simulink model "KUKA_LBR_Simulink_model_flatness_based_control"  (R2017a)
(part 11 of 19)

dblCoriolisCentrifugalFullRow1Col6 = (q14*(KUKA_LBR_param_.dblLink7InertZZ*(cos(q6)*sin(q2)*sin(q3)*sin(q5) + cos(q2)*(cos(q5)*cos(q6)*sin(q4) - cos(q4)*sin(q6)) - cos(q3)*sin(q2)*(cos(q4)*cos(q5)*cos(q6) + sin(q4)*sin(q6))) - (-(cos(q5)*(cos(q3)*sin(q1) + cos(q1)*cos(q2)*sin(q3))) + (cos(q4)*sin(q1)*sin(q3) - cos(q1)*(cos(q2)*cos(q3)*cos(q4) + sin(q2)*sin(q4)))*sin(q5))*(KUKA_LBR_param_.dblLink7InertXX*(cos(q6)*(-(cos(q4)*sin(q1)*sin(q2)) + (cos(q2)*cos(q3)*sin(q1) + cos(q1)*sin(q3))*sin(q4)) - (cos(q5)*sin(q1)*sin(q2)*sin(q4) + cos(q1)*(cos(q4)*cos(q5)*sin(q3) + cos(q3)*sin(q5)) + cos(q2)*sin(q1)*(cos(q3)*cos(q4)*cos(q5) - sin(q3)*sin(q5)))*sin(q6)) + KUKA_LBR_param_.dblLink7InertXY*(cos(q6)*(sin(q1)*sin(q3)*sin(q4) + cos(q1)*(cos(q4)*sin(q2) - cos(q2)*cos(q3)*sin(q4))) + (-(sin(q1)*(cos(q4)*cos(q5)*sin(q3) + cos(q3)*sin(q5))) + cos(q1)*(cos(q5)*sin(q2)*sin(q4) + cos(q2)*(cos(q3)*cos(q4)*cos(q5) - sin(q3)*sin(q5))))*sin(q6))) - (cos(q1)*(cos(q3)*cos(q5) - cos(q4)*sin(q3)*sin(q5)) - sin(q1)*(sin(q2)*sin(q4)*sin(q5) + cos(q2)*(cos(q5)*sin(q3) + cos(q3)*cos(q4)*sin(q5))))*(KUKA_LBR_param_.dblLink7InertXY*(cos(q6)*(-(cos(q4)*sin(q1)*sin(q2)) + (cos(q2)*cos(q3)*sin(q1) + cos(q1)*sin(q3))*sin(q4)) - (cos(q5)*sin(q1)*sin(q2)*sin(q4) + cos(q1)*(cos(q4)*cos(q5)*sin(q3) + cos(q3)*sin(q5)) + cos(q2)*sin(q1)*(cos(q3)*cos(q4)*cos(q5) - sin(q3)*sin(q5)))*sin(q6)) + KUKA_LBR_param_.dblLink7InertYY*(cos(q6)*(sin(q1)*sin(q3)*sin(q4) + cos(q1)*(cos(q4)*sin(q2) - cos(q2)*cos(q3)*sin(q4))) + (-(sin(q1)*(cos(q4)*cos(q5)*sin(q3) + cos(q3)*sin(q5))) + cos(q1)*(cos(q5)*sin(q2)*sin(q4) + cos(q2)*(cos(q3)*cos(q4)*cos(q5) - sin(q3)*sin(q5))))*sin(q6))) - (cos(q5)*sin(q2)*sin(q3) + (cos(q3)*cos(q4)*sin(q2) - cos(q2)*sin(q4))*sin(q5))*(KUKA_LBR_param_.dblLink7InertXZ*(cos(q6)*(-(cos(q4)*sin(q1)*sin(q2)) + (cos(q2)*cos(q3)*sin(q1) + cos(q1)*sin(q3))*sin(q4)) - (cos(q5)*sin(q1)*sin(q2)*sin(q4) + cos(q1)*(cos(q4)*cos(q5)*sin(q3) + cos(q3)*sin(q5)) + cos(q2)*sin(q1)*(cos(q3)*cos(q4)*cos(q5) - sin(q3)*sin(q5)))*sin(q6)) + KUKA_LBR_param_.dblLink7InertYZ*(cos(q6)*(sin(q1)*sin(q3)*sin(q4) + cos(q1)*(cos(q4)*sin(q2) - cos(q2)*cos(q3)*sin(q4))) + (-(sin(q1)*(cos(q4)*cos(q5)*sin(q3) + cos(q3)*sin(q5))) + cos(q1)*(cos(q5)*sin(q2)*sin(q4) + cos(q2)*(cos(q3)*cos(q4)*cos(q5) - sin(q3)*sin(q5))))*sin(q6))) + KUKA_LBR_param_.dblLink7InertYZ*(sin(q1)*sin(q2)*(cos(q5)*cos(q6)*sin(q4) - cos(q4)*sin(q6)) + cos(q1)*(cos(q4)*cos(q5)*cos(q6)*sin(q3) + cos(q3)*cos(q6)*sin(q5) + sin(q3)*sin(q4)*sin(q6)) + cos(q2)*sin(q1)*(-(cos(q6)*sin(q3)*sin(q5)) + cos(q3)*(cos(q4)*cos(q5)*cos(q6) + sin(q4)*sin(q6)))) + KUKA_LBR_param_.dblLink7InertXZ*(-(sin(q1)*(cos(q4)*cos(q5)*cos(q6)*sin(q3) + cos(q3)*cos(q6)*sin(q5) + sin(q3)*sin(q4)*sin(q6))) + cos(q1)*(sin(q2)*(cos(q5)*cos(q6)*sin(q4) - cos(q4)*sin(q6)) + cos(q2)*(cos(q3)*cos(q4)*cos(q5)*cos(q6) - cos(q6)*sin(q3)*sin(q5) + cos(q3)*sin(q4)*sin(q6)))) - (cos(q1)*(-(cos(q3)*cos(q5)) + cos(q4)*sin(q3)*sin(q5)) + sin(q1)*(sin(q2)*sin(q4)*sin(q5) + cos(q2)*(cos(q5)*sin(q3) + cos(q3)*cos(q4)*sin(q5))))*(KUKA_LBR_param_.dblLink7InertXX*(cos(q6)*(sin(q1)*sin(q3)*sin(q4) + cos(q1)*(cos(q4)*sin(q2) - cos(q2)*cos(q3)*sin(q4))) - (cos(q5)*(cos(q4)*sin(q1)*sin(q3) - cos(q1)*(cos(q2)*cos(q3)*cos(q4) + sin(q2)*sin(q4))) + (cos(q3)*sin(q1) + cos(q1)*cos(q2)*sin(q3))*sin(q5))*sin(q6)) + KUKA_LBR_param_.dblLink7InertXY*(cos(q6)*(cos(q4)*sin(q1)*sin(q2) - (cos(q2)*cos(q3)*sin(q1) + cos(q1)*sin(q3))*sin(q4)) + (cos(q5)*sin(q1)*sin(q2)*sin(q4) + cos(q1)*(cos(q4)*cos(q5)*sin(q3) + cos(q3)*sin(q5)) + cos(q2)*sin(q1)*(cos(q3)*cos(q4)*cos(q5) - sin(q3)*sin(q5)))*sin(q6)) + KUKA_LBR_param_.dblLink7InertXZ*(cos(q2)*(cos(q4)*cos(q6) + cos(q5)*sin(q4)*sin(q6)) + sin(q2)*(sin(q3)*sin(q5)*sin(q6) + cos(q3)*(cos(q6)*sin(q4) - cos(q4)*cos(q5)*sin(q6))))) - (sin(q1)*(-(cos(q3)*cos(q5)) + cos(q4)*sin(q3)*sin(q5)) - cos(q1)*(sin(q2)*sin(q4)*sin(q5) + cos(q2)*(cos(q5)*sin(q3) + cos(q3)*cos(q4)*sin(q5))))*(KUKA_LBR_param_.dblLink7InertXY*(cos(q6)*(sin(q1)*sin(q3)*sin(q4) + cos(q1)*(cos(q4)*sin(q2) - cos(q2)*cos(q3)*sin(q4))) - (cos(q5)*(cos(q4)*sin(q1)*sin(q3) - cos(q1)*(cos(q2)*cos(q3)*cos(q4) + sin(q2)*sin(q4))) + (cos(q3)*sin(q1) + cos(q1)*cos(q2)*sin(q3))*sin(q5))*sin(q6)) + KUKA_LBR_param_.dblLink7InertYY*(cos(q6)*(cos(q4)*sin(q1)*sin(q2) - (cos(q2)*cos(q3)*sin(q1) + cos(q1)*sin(q3))*sin(q4)) + (cos(q5)*sin(q1)*sin(q2)*sin(q4) + cos(q1)*(cos(q4)*cos(q5)*sin(q3) + cos(q3)*sin(q5)) + cos(q2)*sin(q1)*(cos(q3)*cos(q4)*cos(q5) - sin(q3)*sin(q5)))*sin(q6)) + KUKA_LBR_param_.dblLink7InertYZ*(cos(q2)*(cos(q4)*cos(q6) + cos(q5)*sin(q4)*sin(q6)) + sin(q2)*(sin(q3)*sin(q5)*sin(q6) + cos(q3)*(cos(q6)*sin(q4) - cos(q4)*cos(q5)*sin(q6))))) - KUKA_LBR_param_.dblLink7Mass*(sin(q1)*(cos(q6)*(-(KUKA_LBR_param_.dblLink7CogX*cos(q7)*sin(q3)*sin(q4)) + KUKA_LBR_param_.dblLink7CogZ*cos(q3)*sin(q5) + KUKA_LBR_param_.dblLink7CogY*sin(q3)*sin(q4)*sin(q7)) + sin(q6)*(KUKA_LBR_param_.dblLink7CogZ*sin(q3)*sin(q4) + cos(q3)*sin(q5)*(KUKA_LBR_param_.dblLink7CogX*cos(q7) - KUKA_LBR_param_.dblLink7CogY*sin(q7))) + cos(q4)*cos(q5)*sin(q3)*(KUKA_LBR_param_.dblLink7CogZ*cos(q6) + sin(q6)*(KUKA_LBR_param_.dblLink7CogX*cos(q7) - KUKA_LBR_param_.dblLink7CogY*sin(q7)))) - cos(q1)*(sin(q2)*(cos(q4)*(KUKA_LBR_param_.dblLink7CogX*cos(q6)*cos(q7) - KUKA_LBR_param_.dblLink7CogZ*sin(q6) - KUKA_LBR_param_.dblLink7CogY*cos(q6)*sin(q7)) + cos(q5)*sin(q4)*(KUKA_LBR_param_.dblLink7CogZ*cos(q6) + KUKA_LBR_param_.dblLink7CogX*cos(q7)*sin(q6) - KUKA_LBR_param_.dblLink7CogY*sin(q6)*sin(q7))) + cos(q2)*(-(sin(q3)*sin(q5)*(KUKA_LBR_param_.dblLink7CogZ*cos(q6) + sin(q6)*(KUKA_LBR_param_.dblLink7CogX*cos(q7) - KUKA_LBR_param_.dblLink7CogY*sin(q7)))) + cos(q3)*(sin(q4)*(-(KUKA_LBR_param_.dblLink7CogX*cos(q6)*cos(q7)) + KUKA_LBR_param_.dblLink7CogZ*sin(q6) + KUKA_LBR_param_.dblLink7CogY*cos(q6)*sin(q7)) + cos(q4)*cos(q5)*(KUKA_LBR_param_.dblLink7CogZ*cos(q6) + KUKA_LBR_param_.dblLink7CogX*cos(q7)*sin(q6) - KUKA_LBR_param_.dblLink7CogY*sin(q6)*sin(q7))))))*(cos(q1)*(cos(q3)*(-(cos(q6)*sin(q5)*(KUKA_LBR_param_.dblLink7CogY*cos(q7) + KUKA_LBR_param_.dblLink7CogX*sin(q7))) + cos(q5)*(KUKA_LBR_param_.dblLink7CogX*cos(q7) - KUKA_LBR_param_.dblLink7CogY*sin(q7))) - sin(q3)*(sin(q4)*sin(q6)*(KUKA_LBR_param_.dblLink7CogY*cos(q7) + KUKA_LBR_param_.dblLink7CogX*sin(q7)) + cos(q4)*(cos(q5)*cos(q6)*(KUKA_LBR_param_.dblLink7CogY*cos(q7) + KUKA_LBR_param_.dblLink7CogX*sin(q7)) + sin(q5)*(KUKA_LBR_param_.dblLink7CogX*cos(q7) - KUKA_LBR_param_.dblLink7CogY*sin(q7))))) + sin(q1)*(-(sin(q2)*(KUKA_LBR_param_.dblLink7CogX*cos(q7)*sin(q4)*sin(q5) - KUKA_LBR_param_.dblLink7CogY*sin(q4)*sin(q5)*sin(q7) + cos(q5)*cos(q6)*sin(q4)*(KUKA_LBR_param_.dblLink7CogY*cos(q7) + KUKA_LBR_param_.dblLink7CogX*sin(q7)) - cos(q4)*sin(q6)*(KUKA_LBR_param_.dblLink7CogY*cos(q7) + KUKA_LBR_param_.dblLink7CogX*sin(q7)))) + cos(q2)*(sin(q3)*(cos(q6)*sin(q5)*(KUKA_LBR_param_.dblLink7CogY*cos(q7) + KUKA_LBR_param_.dblLink7CogX*sin(q7)) + cos(q5)*(-(KUKA_LBR_param_.dblLink7CogX*cos(q7)) + KUKA_LBR_param_.dblLink7CogY*sin(q7))) - cos(q3)*(sin(q4)*sin(q6)*(KUKA_LBR_param_.dblLink7CogY*cos(q7) + KUKA_LBR_param_.dblLink7CogX*sin(q7)) + cos(q4)*(cos(q5)*cos(q6)*(KUKA_LBR_param_.dblLink7CogY*cos(q7) + KUKA_LBR_param_.dblLink7CogX*sin(q7)) + sin(q5)*(KUKA_LBR_param_.dblLink7CogX*cos(q7) - KUKA_LBR_param_.dblLink7CogY*sin(q7))))))) - KUKA_LBR_param_.dblLink7Mass*(cos(q1)*(-(cos(q3)*sin(q5)*(KUKA_LBR_param_.dblLink7CogZ*cos(q6) + sin(q6)*(KUKA_LBR_param_.dblLink7CogX*cos(q7) - KUKA_LBR_param_.dblLink7CogY*sin(q7)))) + sin(q3)*(-(cos(q4)*cos(q5)*(KUKA_LBR_param_.dblLink7CogZ*cos(q6) + sin(q6)*(KUKA_LBR_param_.dblLink7CogX*cos(q7) - KUKA_LBR_param_.dblLink7CogY*sin(q7)))) - sin(q4)*(KUKA_LBR_param_.dblLink7CogZ*sin(q6) + cos(q6)*(-(KUKA_LBR_param_.dblLink7CogX*cos(q7)) + KUKA_LBR_param_.dblLink7CogY*sin(q7))))) + sin(q1)*(sin(q2)*(cos(q4)*(-(KUKA_LBR_param_.dblLink7CogX*cos(q6)*cos(q7)) + KUKA_LBR_param_.dblLink7CogZ*sin(q6) + KUKA_LBR_param_.dblLink7CogY*cos(q6)*sin(q7)) - cos(q5)*sin(q4)*(KUKA_LBR_param_.dblLink7CogZ*cos(q6) + KUKA_LBR_param_.dblLink7CogX*cos(q7)*sin(q6) - KUKA_LBR_param_.dblLink7CogY*sin(q6)*sin(q7))) - cos(q2)*(-(sin(q3)*sin(q5)*(KUKA_LBR_param_.dblLink7CogZ*cos(q6) + sin(q6)*(KUKA_LBR_param_.dblLink7CogX*cos(q7) - KUKA_LBR_param_.dblLink7CogY*sin(q7)))) + cos(q3)*(sin(q4)*(-(KUKA_LBR_param_.dblLink7CogX*cos(q6)*cos(q7)) + KUKA_LBR_param_.dblLink7CogZ*sin(q6) + KUKA_LBR_param_.dblLink7CogY*cos(q6)*sin(q7)) + cos(q4)*cos(q5)*(KUKA_LBR_param_.dblLink7CogZ*cos(q6) + KUKA_LBR_param_.dblLink7CogX*cos(q7)*sin(q6) - KUKA_LBR_param_.dblLink7CogY*sin(q6)*sin(q7))))))*(sin(q1)*(cos(q3)*(cos(q6)*sin(q5)*(KUKA_LBR_param_.dblLink7CogY*cos(q7) + KUKA_LBR_param_.dblLink7CogX*sin(q7)) + cos(q5)*(-(KUKA_LBR_param_.dblLink7CogX*cos(q7)) + KUKA_LBR_param_.dblLink7CogY*sin(q7))) + sin(q3)*(sin(q4)*sin(q6)*(KUKA_LBR_param_.dblLink7CogY*cos(q7) + KUKA_LBR_param_.dblLink7CogX*sin(q7)) + cos(q4)*(cos(q5)*cos(q6)*(KUKA_LBR_param_.dblLink7CogY*cos(q7) + KUKA_LBR_param_.dblLink7CogX*sin(q7)) + sin(q5)*(KUKA_LBR_param_.dblLink7CogX*cos(q7) - KUKA_LBR_param_.dblLink7CogY*sin(q7))))) - cos(q1)*(sin(q2)*(cos(q7)*(KUKA_LBR_param_.dblLink7CogX*sin(q4)*sin(q5) - KUKA_LBR_param_.dblLink7CogY*cos(q4)*sin(q6)) - (KUKA_LBR_param_.dblLink7CogY*sin(q4)*sin(q5) + KUKA_LBR_param_.dblLink7CogX*cos(q4)*sin(q6))*sin(q7) + cos(q5)*cos(q6)*sin(q4)*(KUKA_LBR_param_.dblLink7CogY*cos(q7) + KUKA_LBR_param_.dblLink7CogX*sin(q7))) + cos(q2)*(sin(q3)*(-(cos(q6)*sin(q5)*(KUKA_LBR_param_.dblLink7CogY*cos(q7) + KUKA_LBR_param_.dblLink7CogX*sin(q7))) + cos(q5)*(KUKA_LBR_param_.dblLink7CogX*cos(q7) - KUKA_LBR_param_.dblLink7CogY*sin(q7))) + cos(q3)*(sin(q4)*sin(q6)*(KUKA_LBR_param_.dblLink7CogY*cos(q7) + KUKA_LBR_param_.dblLink7CogX*sin(q7)) + cos(q4)*(cos(q5)*cos(q6)*(KUKA_LBR_param_.dblLink7CogY*cos(q7) + KUKA_LBR_param_.dblLink7CogX*sin(q7)) + sin(q5)*(KUKA_LBR_param_.dblLink7CogX*cos(q7) - KUKA_LBR_param_.dblLink7CogY*sin(q7))))))) - KUKA_LBR_param_.dblLink7Mass*(-(cos(q1)*(cos(q6)*(-(KUKA_LBR_param_.dblLink7CogX*cos(q7)*sin(q3)*sin(q4)) + KUKA_LBR_param_.dblLink7CogZ*cos(q3)*sin(q5) + KUKA_LBR_param_.dblLink7CogY*sin(q3)*sin(q4)*sin(q7)) + sin(q6)*(KUKA_LBR_param_.dblLink7CogZ*sin(q3)*sin(q4) + cos(q3)*sin(q5)*(KUKA_LBR_param_.dblLink7CogX*cos(q7) - KUKA_LBR_param_.dblLink7CogY*sin(q7))) + cos(q4)*cos(q5)*sin(q3)*(KUKA_LBR_param_.dblLink7CogZ*cos(q6) + sin(q6)*(KUKA_LBR_param_.dblLink7CogX*cos(q7) - KUKA_LBR_param_.dblLink7CogY*sin(q7))))) - sin(q1)*(sin(q2)*(cos(q4)*(KUKA_LBR_param_.dblLink7CogX*cos(q6)*cos(q7) - KUKA_LBR_param_.dblLink7CogZ*sin(q6) - KUKA_LBR_param_.dblLink7CogY*cos(q6)*sin(q7)) + cos(q5)*sin(q4)*(KUKA_LBR_param_.dblLink7CogZ*cos(q6) + KUKA_LBR_param_.dblLink7CogX*cos(q7)*sin(q6) - KUKA_LBR_param_.dblLink7CogY*sin(q6)*sin(q7))) + cos(q2)*(-(sin(q3)*sin(q5)*(KUKA_LBR_param_.dblLink7CogZ*cos(q6) + sin(q6)*(KUKA_LBR_param_.dblLink7CogX*cos(q7) - KUKA_LBR_param_.dblLink7CogY*sin(q7)))) + cos(q3)*(sin(q4)*(-(KUKA_LBR_param_.dblLink7CogX*cos(q6)*cos(q7)) + KUKA_LBR_param_.dblLink7CogZ*sin(q6) + KUKA_LBR_param_.dblLink7CogY*cos(q6)*sin(q7)) + cos(q4)*cos(q5)*(KUKA_LBR_param_.dblLink7CogZ*cos(q6) + KUKA_LBR_param_.dblLink7CogX*cos(q7)*sin(q6) - KUKA_LBR_param_.dblLink7CogY*sin(q6)*sin(q7))))))*(sin(q1)*(cos(q3)*(-(cos(q6)*sin(q5)*(KUKA_LBR_param_.dblLink7CogY*cos(q7) + KUKA_LBR_param_.dblLink7CogX*sin(q7))) + cos(q5)*(KUKA_LBR_param_.dblLink7CogX*cos(q7) - KUKA_LBR_param_.dblLink7CogY*sin(q7))) - sin(q3)*(sin(q4)*sin(q6)*(KUKA_LBR_param_.dblLink7CogY*cos(q7) + KUKA_LBR_param_.dblLink7CogX*sin(q7)) + cos(q4)*(cos(q5)*cos(q6)*(KUKA_LBR_param_.dblLink7CogY*cos(q7) + KUKA_LBR_param_.dblLink7CogX*sin(q7)) + sin(q5)*(KUKA_LBR_param_.dblLink7CogX*cos(q7) - KUKA_LBR_param_.dblLink7CogY*sin(q7))))) + cos(q1)*(sin(q2)*(cos(q7)*(KUKA_LBR_param_.dblLink7CogX*sin(q4)*sin(q5) - KUKA_LBR_param_.dblLink7CogY*cos(q4)*sin(q6)) - (KUKA_LBR_param_.dblLink7CogY*sin(q4)*sin(q5) + KUKA_LBR_param_.dblLink7CogX*cos(q4)*sin(q6))*sin(q7) + cos(q5)*cos(q6)*sin(q4)*(KUKA_LBR_param_.dblLink7CogY*cos(q7) + KUKA_LBR_param_.dblLink7CogX*sin(q7))) + cos(q2)*(sin(q3)*(-(cos(q6)*sin(q5)*(KUKA_LBR_param_.dblLink7CogY*cos(q7) + KUKA_LBR_param_.dblLink7CogX*sin(q7))) + cos(q5)*(KUKA_LBR_param_.dblLink7CogX*cos(q7) - KUKA_LBR_param_.dblLink7CogY*sin(q7))) + cos(q3)*(sin(q4)*sin(q6)*(KUKA_LBR_param_.dblLink7CogY*cos(q7) + KUKA_LBR_param_.dblLink7CogX*sin(q7)) + cos(q4)*(cos(q5)*cos(q6)*(KUKA_LBR_param_.dblLink7CogY*cos(q7) + KUKA_LBR_param_.dblLink7CogX*sin(q7)) + sin(q5)*(KUKA_LBR_param_.dblLink7CogX*cos(q7) - KUKA_LBR_param_.dblLink7CogY*sin(q7))))))) - KUKA_LBR_param_.dblLink7Mass*(KUKA_LBR_param_.dblLink7CogZ*cos(q5)*cos(q6)*sin(q1)*sin(q2)*sin(q4) - KUKA_LBR_param_.dblLink7CogX*cos(q1)*cos(q6)*cos(q7)*sin(q3)*sin(q4) + KUKA_LBR_param_.dblLink7CogZ*cos(q1)*cos(q3)*cos(q6)*sin(q5) + KUKA_LBR_param_.dblLink7CogX*cos(q5)*cos(q7)*sin(q1)*sin(q2)*sin(q4)*sin(q6) + KUKA_LBR_param_.dblLink7CogZ*cos(q1)*sin(q3)*sin(q4)*sin(q6) + KUKA_LBR_param_.dblLink7CogX*cos(q1)*cos(q3)*cos(q7)*sin(q5)*sin(q6) + KUKA_LBR_param_.dblLink7CogY*cos(q1)*cos(q6)*sin(q3)*sin(q4)*sin(q7) - KUKA_LBR_param_.dblLink7CogY*cos(q5)*sin(q1)*sin(q2)*sin(q4)*sin(q6)*sin(q7) - KUKA_LBR_param_.dblLink7CogY*cos(q1)*cos(q3)*sin(q5)*sin(q6)*sin(q7) + cos(q4)*(cos(q6)*(KUKA_LBR_param_.dblLink7CogX*cos(q7)*sin(q1)*sin(q2) + KUKA_LBR_param_.dblLink7CogZ*cos(q1)*cos(q5)*sin(q3) - KUKA_LBR_param_.dblLink7CogY*sin(q1)*sin(q2)*sin(q7)) - sin(q6)*(KUKA_LBR_param_.dblLink7CogZ*sin(q1)*sin(q2) + cos(q1)*cos(q5)*sin(q3)*(-(KUKA_LBR_param_.dblLink7CogX*cos(q7)) + KUKA_LBR_param_.dblLink7CogY*sin(q7)))) + cos(q2)*sin(q1)*(-(sin(q3)*sin(q5)*(KUKA_LBR_param_.dblLink7CogZ*cos(q6) + sin(q6)*(KUKA_LBR_param_.dblLink7CogX*cos(q7) - KUKA_LBR_param_.dblLink7CogY*sin(q7)))) + cos(q3)*(sin(q4)*(-(KUKA_LBR_param_.dblLink7CogX*cos(q6)*cos(q7)) + KUKA_LBR_param_.dblLink7CogZ*sin(q6) + KUKA_LBR_param_.dblLink7CogY*cos(q6)*sin(q7)) + cos(q4)*cos(q5)*(KUKA_LBR_param_.dblLink7CogZ*cos(q6) + KUKA_LBR_param_.dblLink7CogX*cos(q7)*sin(q6) - KUKA_LBR_param_.dblLink7CogY*sin(q6)*sin(q7)))))*(-(sin(q1)*(cos(q3)*(cos(q6)*sin(q5)*(KUKA_LBR_param_.dblLink7CogY*cos(q7) + KUKA_LBR_param_.dblLink7CogX*sin(q7)) + cos(q5)*(-(KUKA_LBR_param_.dblLink7CogX*cos(q7)) + KUKA_LBR_param_.dblLink7CogY*sin(q7))) + sin(q3)*(sin(q4)*sin(q6)*(KUKA_LBR_param_.dblLink7CogY*cos(q7) + KUKA_LBR_param_.dblLink7CogX*sin(q7)) + cos(q4)*(cos(q5)*cos(q6)*(KUKA_LBR_param_.dblLink7CogY*cos(q7) + KUKA_LBR_param_.dblLink7CogX*sin(q7)) + sin(q5)*(KUKA_LBR_param_.dblLink7CogX*cos(q7) - KUKA_LBR_param_.dblLink7CogY*sin(q7)))))) + cos(q1)*(sin(q2)*(cos(q7)*(KUKA_LBR_param_.dblLink7CogX*sin(q4)*sin(q5) - KUKA_LBR_param_.dblLink7CogY*cos(q4)*sin(q6)) - (KUKA_LBR_param_.dblLink7CogY*sin(q4)*sin(q5) + KUKA_LBR_param_.dblLink7CogX*cos(q4)*sin(q6))*sin(q7) + cos(q5)*cos(q6)*sin(q4)*(KUKA_LBR_param_.dblLink7CogY*cos(q7) + KUKA_LBR_param_.dblLink7CogX*sin(q7))) + cos(q2)*(sin(q3)*(-(cos(q6)*sin(q5)*(KUKA_LBR_param_.dblLink7CogY*cos(q7) + KUKA_LBR_param_.dblLink7CogX*sin(q7))) + cos(q5)*(KUKA_LBR_param_.dblLink7CogX*cos(q7) - KUKA_LBR_param_.dblLink7CogY*sin(q7))) + cos(q3)*(sin(q4)*sin(q6)*(KUKA_LBR_param_.dblLink7CogY*cos(q7) + KUKA_LBR_param_.dblLink7CogX*sin(q7)) + cos(q4)*(cos(q5)*cos(q6)*(KUKA_LBR_param_.dblLink7CogY*cos(q7) + KUKA_LBR_param_.dblLink7CogX*sin(q7)) + sin(q5)*(KUKA_LBR_param_.dblLink7CogX*cos(q7) - KUKA_LBR_param_.dblLink7CogY*sin(q7))))))) - KUKA_LBR_param_.dblLink7Mass*(-(sin(q1)*(cos(q6)*(-(KUKA_LBR_param_.dblLink7CogX*cos(q7)*sin(q3)*sin(q4)) + KUKA_LBR_param_.dblLink7CogZ*cos(q3)*sin(q5) + KUKA_LBR_param_.dblLink7CogY*sin(q3)*sin(q4)*sin(q7)) + sin(q6)*(KUKA_LBR_param_.dblLink7CogZ*sin(q3)*sin(q4) + cos(q3)*sin(q5)*(KUKA_LBR_param_.dblLink7CogX*cos(q7) - KUKA_LBR_param_.dblLink7CogY*sin(q7))) + cos(q4)*cos(q5)*sin(q3)*(KUKA_LBR_param_.dblLink7CogZ*cos(q6) + sin(q6)*(KUKA_LBR_param_.dblLink7CogX*cos(q7) - KUKA_LBR_param_.dblLink7CogY*sin(q7))))) + cos(q1)*(sin(q2)*(cos(q4)*(KUKA_LBR_param_.dblLink7CogX*cos(q6)*cos(q7) - KUKA_LBR_param_.dblLink7CogZ*sin(q6) - KUKA_LBR_param_.dblLink7CogY*cos(q6)*sin(q7)) + cos(q5)*sin(q4)*(KUKA_LBR_param_.dblLink7CogZ*cos(q6) + KUKA_LBR_param_.dblLink7CogX*cos(q7)*sin(q6) - KUKA_LBR_param_.dblLink7CogY*sin(q6)*sin(q7))) + cos(q2)*(-(sin(q3)*sin(q5)*(KUKA_LBR_param_.dblLink7CogZ*cos(q6) + sin(q6)*(KUKA_LBR_param_.dblLink7CogX*cos(q7) - KUKA_LBR_param_.dblLink7CogY*sin(q7)))) + cos(q3)*(sin(q4)*(-(KUKA_LBR_param_.dblLink7CogX*cos(q6)*cos(q7)) + KUKA_LBR_param_.dblLink7CogZ*sin(q6) + KUKA_LBR_param_.dblLink7CogY*cos(q6)*sin(q7)) + cos(q4)*cos(q5)*(KUKA_LBR_param_.dblLink7CogZ*cos(q6) + KUKA_LBR_param_.dblLink7CogX*cos(q7)*sin(q6) - KUKA_LBR_param_.dblLink7CogY*sin(q6)*sin(q7))))))*(cos(q1)*(cos(q3)*(-(cos(q6)*sin(q5)*(KUKA_LBR_param_.dblLink7CogY*cos(q7) + KUKA_LBR_param_.dblLink7CogX*sin(q7))) + cos(q5)*(KUKA_LBR_param_.dblLink7CogX*cos(q7) - KUKA_LBR_param_.dblLink7CogY*sin(q7))) - sin(q3)*(sin(q4)*sin(q6)*(KUKA_LBR_param_.dblLink7CogY*cos(q7) + KUKA_LBR_param_.dblLink7CogX*sin(q7)) + cos(q4)*(cos(q5)*cos(q6)*(KUKA_LBR_param_.dblLink7CogY*cos(q7) + KUKA_LBR_param_.dblLink7CogX*sin(q7)) + sin(q5)*(KUKA_LBR_param_.dblLink7CogX*cos(q7) - KUKA_LBR_param_.dblLink7CogY*sin(q7))))) - sin(q1)*(sin(q2)*(cos(q7)*(KUKA_LBR_param_.dblLink7CogX*sin(q4)*sin(q5) - KUKA_LBR_param_.dblLink7CogY*cos(q4)*sin(q6)) - (KUKA_LBR_param_.dblLink7CogY*sin(q4)*sin(q5) + KUKA_LBR_param_.dblLink7CogX*cos(q4)*sin(q6))*sin(q7) + cos(q5)*cos(q6)*sin(q4)*(KUKA_LBR_param_.dblLink7CogY*cos(q7) + KUKA_LBR_param_.dblLink7CogX*sin(q7))) + cos(q2)*(sin(q3)*(-(cos(q6)*sin(q5)*(KUKA_LBR_param_.dblLink7CogY*cos(q7) + KUKA_LBR_param_.dblLink7CogX*sin(q7))) + cos(q5)*(KUKA_LBR_param_.dblLink7CogX*cos(q7) - KUKA_LBR_param_.dblLink7CogY*sin(q7))) + cos(q3)*(sin(q4)*sin(q6)*(KUKA_LBR_param_.dblLink7CogY*cos(q7) + KUKA_LBR_param_.dblLink7CogX*sin(q7)) + cos(q4)*(cos(q5)*cos(q6)*(KUKA_LBR_param_.dblLink7CogY*cos(q7) + KUKA_LBR_param_.dblLink7CogX*sin(q7)) + sin(q5)*(KUKA_LBR_param_.dblLink7CogX*cos(q7) - KUKA_LBR_param_.dblLink7CogY*sin(q7))))))) - KUKA_LBR_param_.dblLink7Mass*(-(sin(q1)*(cos(q6)*(-(KUKA_LBR_param_.dblLink7CogX*cos(q7)*sin(q3)*sin(q4)) + KUKA_LBR_param_.dblLink7CogZ*cos(q3)*sin(q5) + KUKA_LBR_param_.dblLink7CogY*sin(q3)*sin(q4)*sin(q7)) + sin(q6)*(KUKA_LBR_param_.dblLink7CogZ*sin(q3)*sin(q4) + cos(q3)*sin(q5)*(KUKA_LBR_param_.dblLink7CogX*cos(q7) - KUKA_LBR_param_.dblLink7CogY*sin(q7))) + cos(q4)*cos(q5)*sin(q3)*(KUKA_LBR_param_.dblLink7CogZ*cos(q6) + sin(q6)*(KUKA_LBR_param_.dblLink7CogX*cos(q7) - KUKA_LBR_param_.dblLink7CogY*sin(q7))))) + cos(q1)*(sin(q2)*(cos(q4)*(KUKA_LBR_param_.dblLink7CogX*cos(q6)*cos(q7) - KUKA_LBR_param_.dblLink7CogZ*sin(q6) - KUKA_LBR_param_.dblLink7CogY*cos(q6)*sin(q7)) + cos(q5)*sin(q4)*(KUKA_LBR_param_.dblLink7CogZ*cos(q6) + KUKA_LBR_param_.dblLink7CogX*cos(q7)*sin(q6) - KUKA_LBR_param_.dblLink7CogY*sin(q6)*sin(q7))) + cos(q2)*(-(sin(q3)*sin(q5)*(KUKA_LBR_param_.dblLink7CogZ*cos(q6) + sin(q6)*(KUKA_LBR_param_.dblLink7CogX*cos(q7) - KUKA_LBR_param_.dblLink7CogY*sin(q7)))) + cos(q3)*(sin(q4)*(-(KUKA_LBR_param_.dblLink7CogX*cos(q6)*cos(q7)) + KUKA_LBR_param_.dblLink7CogZ*sin(q6) + KUKA_LBR_param_.dblLink7CogY*cos(q6)*sin(q7)) + cos(q4)*cos(q5)*(KUKA_LBR_param_.dblLink7CogZ*cos(q6) + KUKA_LBR_param_.dblLink7CogX*cos(q7)*sin(q6) - KUKA_LBR_param_.dblLink7CogY*sin(q6)*sin(q7))))))*(cos(q1)*(cos(q3)*(cos(q6)*sin(q5)*(KUKA_LBR_param_.dblLink7CogY*cos(q7) + KUKA_LBR_param_.dblLink7CogX*sin(q7)) + cos(q5)*(-(KUKA_LBR_param_.dblLink7CogX*cos(q7)) + KUKA_LBR_param_.dblLink7CogY*sin(q7))) + sin(q3)*(sin(q4)*sin(q6)*(KUKA_LBR_param_.dblLink7CogY*cos(q7) + KUKA_LBR_param_.dblLink7CogX*sin(q7)) + cos(q4)*(cos(q5)*cos(q6)*(KUKA_LBR_param_.dblLink7CogY*cos(q7) + KUKA_LBR_param_.dblLink7CogX*sin(q7)) + sin(q5)*(KUKA_LBR_param_.dblLink7CogX*cos(q7) - KUKA_LBR_param_.dblLink7CogY*sin(q7))))) + sin(q1)*(sin(q2)*(cos(q7)*(KUKA_LBR_param_.dblLink7CogX*sin(q4)*sin(q5) - KUKA_LBR_param_.dblLink7CogY*cos(q4)*sin(q6)) - (KUKA_LBR_param_.dblLink7CogY*sin(q4)*sin(q5) + KUKA_LBR_param_.dblLink7CogX*cos(q4)*sin(q6))*sin(q7) + cos(q5)*cos(q6)*sin(q4)*(KUKA_LBR_param_.dblLink7CogY*cos(q7) + KUKA_LBR_param_.dblLink7CogX*sin(q7))) + cos(q2)*(sin(q3)*(-(cos(q6)*sin(q5)*(KUKA_LBR_param_.dblLink7CogY*cos(q7) + KUKA_LBR_param_.dblLink7CogX*sin(q7))) + cos(q5)*(KUKA_LBR_param_.dblLink7CogX*cos(q7) - KUKA_LBR_param_.dblLink7CogY*sin(q7))) + cos(q3)*(sin(q4)*sin(q6)*(KUKA_LBR_param_.dblLink7CogY*cos(q7) + KUKA_LBR_param_.dblLink7CogX*sin(q7)) + cos(q4)*(cos(q5)*cos(q6)*(KUKA_LBR_param_.dblLink7CogY*cos(q7) + KUKA_LBR_param_.dblLink7CogX*sin(q7)) + sin(q5)*(KUKA_LBR_param_.dblLink7CogX*cos(q7) - KUKA_LBR_param_.dblLink7CogY*sin(q7))))))) + KUKA_LBR_param_.dblLink7Mass*(sin(q1)*(-(cos(q3)*sin(q5)*(KUKA_LBR_param_.dblLink7CogZ*cos(q6) + sin(q6)*(KUKA_LBR_param_.dblLink7CogX*cos(q7) - KUKA_LBR_param_.dblLink7CogY*sin(q7)))) + sin(q3)*(-(cos(q4)*cos(q5)*(KUKA_LBR_param_.dblLink7CogZ*cos(q6) + sin(q6)*(KUKA_LBR_param_.dblLink7CogX*cos(q7) - KUKA_LBR_param_.dblLink7CogY*sin(q7)))) - sin(q4)*(KUKA_LBR_param_.dblLink7CogZ*sin(q6) + cos(q6)*(-(KUKA_LBR_param_.dblLink7CogX*cos(q7)) + KUKA_LBR_param_.dblLink7CogY*sin(q7))))) + cos(q1)*(sin(q2)*(cos(q4)*(KUKA_LBR_param_.dblLink7CogX*cos(q6)*cos(q7) - KUKA_LBR_param_.dblLink7CogZ*sin(q6) - KUKA_LBR_param_.dblLink7CogY*cos(q6)*sin(q7)) + cos(q5)*sin(q4)*(KUKA_LBR_param_.dblLink7CogZ*cos(q6) + KUKA_LBR_param_.dblLink7CogX*cos(q7)*sin(q6) - KUKA_LBR_param_.dblLink7CogY*sin(q6)*sin(q7))) + cos(q2)*(-(sin(q3)*sin(q5)*(KUKA_LBR_param_.dblLink7CogZ*cos(q6) + sin(q6)*(KUKA_LBR_param_.dblLink7CogX*cos(q7) - KUKA_LBR_param_.dblLink7CogY*sin(q7)))) + cos(q3)*(sin(q4)*(-(KUKA_LBR_param_.dblLink7CogX*cos(q6)*cos(q7)) + KUKA_LBR_param_.dblLink7CogZ*sin(q6) + KUKA_LBR_param_.dblLink7CogY*cos(q6)*sin(q7)) + cos(q4)*cos(q5)*(KUKA_LBR_param_.dblLink7CogZ*cos(q6) + KUKA_LBR_param_.dblLink7CogX*cos(q7)*sin(q6) - KUKA_LBR_param_.dblLink7CogY*sin(q6)*sin(q7))))))*(cos(q1)*(cos(q3)*(cos(q6)*sin(q5)*(KUKA_LBR_param_.dblLink7CogY*cos(q7) + KUKA_LBR_param_.dblLink7CogX*sin(q7)) + cos(q5)*(-(KUKA_LBR_param_.dblLink7CogX*cos(q7)) + KUKA_LBR_param_.dblLink7CogY*sin(q7))) + sin(q3)*(sin(q4)*sin(q6)*(KUKA_LBR_param_.dblLink7CogY*cos(q7) + KUKA_LBR_param_.dblLink7CogX*sin(q7)) + cos(q4)*(cos(q5)*cos(q6)*(KUKA_LBR_param_.dblLink7CogY*cos(q7) + KUKA_LBR_param_.dblLink7CogX*sin(q7)) + sin(q5)*(KUKA_LBR_param_.dblLink7CogX*cos(q7) - KUKA_LBR_param_.dblLink7CogY*sin(q7))))) + sin(q1)*(sin(q2)*(cos(q7)*(KUKA_LBR_param_.dblLink7CogX*sin(q4)*sin(q5) - KUKA_LBR_param_.dblLink7CogY*cos(q4)*sin(q6)) - (KUKA_LBR_param_.dblLink7CogY*sin(q4)*sin(q5) + KUKA_LBR_param_.dblLink7CogX*cos(q4)*sin(q6))*sin(q7) + cos(q5)*cos(q6)*sin(q4)*(KUKA_LBR_param_.dblLink7CogY*cos(q7) + KUKA_LBR_param_.dblLink7CogX*sin(q7))) + cos(q2)*(sin(q3)*(-(cos(q6)*sin(q5)*(KUKA_LBR_param_.dblLink7CogY*cos(q7) + KUKA_LBR_param_.dblLink7CogX*sin(q7))) + cos(q5)*(KUKA_LBR_param_.dblLink7CogX*cos(q7) - KUKA_LBR_param_.dblLink7CogY*sin(q7))) + cos(q3)*(sin(q4)*sin(q6)*(KUKA_LBR_param_.dblLink7CogY*cos(q7) + KUKA_LBR_param_.dblLink7CogX*sin(q7)) + cos(q4)*(cos(q5)*cos(q6)*(KUKA_LBR_param_.dblLink7CogY*cos(q7) + KUKA_LBR_param_.dblLink7CogX*sin(q7)) + sin(q5)*(KUKA_LBR_param_.dblLink7CogX*cos(q7) - KUKA_LBR_param_.dblLink7CogY*sin(q7))))))) + KUKA_LBR_param_.dblLink7Mass*(KUKA_LBR_param_.dblLink7CogZ*cos(q5)*cos(q6)*sin(q1)*sin(q2)*sin(q4) - KUKA_LBR_param_.dblLink7CogX*cos(q1)*cos(q6)*cos(q7)*sin(q3)*sin(q4) + KUKA_LBR_param_.dblLink7CogZ*cos(q1)*cos(q3)*cos(q6)*sin(q5) + KUKA_LBR_param_.dblLink7CogX*cos(q5)*cos(q7)*sin(q1)*sin(q2)*sin(q4)*sin(q6) + KUKA_LBR_param_.dblLink7CogZ*cos(q1)*sin(q3)*sin(q4)*sin(q6) + KUKA_LBR_param_.dblLink7CogX*cos(q1)*cos(q3)*cos(q7)*sin(q5)*sin(q6) + KUKA_LBR_param_.dblLink7CogY*cos(q1)*cos(q6)*sin(q3)*sin(q4)*sin(q7) - KUKA_LBR_param_.dblLink7CogY*cos(q5)*sin(q1)*sin(q2)*sin(q4)*sin(q6)*sin(q7) - KUKA_LBR_param_.dblLink7CogY*cos(q1)*cos(q3)*sin(q5)*sin(q6)*sin(q7) + cos(q4)*(cos(q6)*(KUKA_LBR_param_.dblLink7CogX*cos(q7)*sin(q1)*sin(q2) + KUKA_LBR_param_.dblLink7CogZ*cos(q1)*cos(q5)*sin(q3) - KUKA_LBR_param_.dblLink7CogY*sin(q1)*sin(q2)*sin(q7)) - sin(q6)*(KUKA_LBR_param_.dblLink7CogZ*sin(q1)*sin(q2) + cos(q1)*cos(q5)*sin(q3)*(-(KUKA_LBR_param_.dblLink7CogX*cos(q7)) + KUKA_LBR_param_.dblLink7CogY*sin(q7)))) + cos(q2)*sin(q1)*(-(sin(q3)*sin(q5)*(KUKA_LBR_param_.dblLink7CogZ*cos(q6) + sin(q6)*(KUKA_LBR_param_.dblLink7CogX*cos(q7) - KUKA_LBR_param_.dblLink7CogY*sin(q7)))) + cos(q3)*(sin(q4)*(-(KUKA_LBR_param_.dblLink7CogX*cos(q6)*cos(q7)) + KUKA_LBR_param_.dblLink7CogZ*sin(q6) + KUKA_LBR_param_.dblLink7CogY*cos(q6)*sin(q7)) + cos(q4)*cos(q5)*(KUKA_LBR_param_.dblLink7CogZ*cos(q6) + KUKA_LBR_param_.dblLink7CogX*cos(q7)*sin(q6) - KUKA_LBR_param_.dblLink7CogY*sin(q6)*sin(q7)))))*(sin(q1)*(cos(q3)*(-(cos(q6)*sin(q5)*(KUKA_LBR_param_.dblLink7CogY*cos(q7) + KUKA_LBR_param_.dblLink7CogX*sin(q7))) + cos(q5)*(KUKA_LBR_param_.dblLink7CogX*cos(q7) - KUKA_LBR_param_.dblLink7CogY*sin(q7))) - sin(q3)*(sin(q4)*sin(q6)*(KUKA_LBR_param_.dblLink7CogY*cos(q7) + KUKA_LBR_param_.dblLink7CogX*sin(q7)) + cos(q4)*(cos(q5)*cos(q6)*(KUKA_LBR_param_.dblLink7CogY*cos(q7) + KUKA_LBR_param_.dblLink7CogX*sin(q7)) + sin(q5)*(KUKA_LBR_param_.dblLink7CogX*cos(q7) - KUKA_LBR_param_.dblLink7CogY*sin(q7))))) + cos(q1)*(sin(q2)*(KUKA_LBR_param_.dblLink7CogX*cos(q7)*sin(q4)*sin(q5) - KUKA_LBR_param_.dblLink7CogY*sin(q4)*sin(q5)*sin(q7) + cos(q5)*cos(q6)*sin(q4)*(KUKA_LBR_param_.dblLink7CogY*cos(q7) + KUKA_LBR_param_.dblLink7CogX*sin(q7)) - cos(q4)*sin(q6)*(KUKA_LBR_param_.dblLink7CogY*cos(q7) + KUKA_LBR_param_.dblLink7CogX*sin(q7))) + cos(q2)*(sin(q3)*(-(cos(q6)*sin(q5)*(KUKA_LBR_param_.dblLink7CogY*cos(q7) + KUKA_LBR_param_.dblLink7CogX*sin(q7))) + cos(q5)*(KUKA_LBR_param_.dblLink7CogX*cos(q7) - KUKA_LBR_param_.dblLink7CogY*sin(q7))) + cos(q3)*(sin(q4)*sin(q6)*(KUKA_LBR_param_.dblLink7CogY*cos(q7) + KUKA_LBR_param_.dblLink7CogX*sin(q7)) + cos(q4)*(cos(q5)*cos(q6)*(KUKA_LBR_param_.dblLink7CogY*cos(q7) + KUKA_LBR_param_.dblLink7CogX*sin(q7)) + sin(q5)*(KUKA_LBR_param_.dblLink7CogX*cos(q7) - KUKA_LBR_param_.dblLink7CogY*sin(q7))))))) - 2*KUKA_LBR_param_.dblLink7Mass*(sin(q1)*(cos(q6)*sin(q3)*sin(q4) - (cos(q4)*cos(q5)*sin(q3) + cos(q3)*sin(q5))*sin(q6)) + cos(q1)*(cos(q5)*sin(q2)*sin(q4)*sin(q6) + cos(q4)*(cos(q6)*sin(q2) + cos(q2)*cos(q3)*cos(q5)*sin(q6)) - cos(q2)*(cos(q3)*cos(q6)*sin(q4) + sin(q3)*sin(q5)*sin(q6))))*(KUKA_LBR_param_.dblLink7CogY*cos(q7) + KUKA_LBR_param_.dblLink7CogX*sin(q7))*(cos(q1)*(cos(q3)*(cos(q5)*(KUKA_LBR_param_.dblLink7CogY*cos(q7) + KUKA_LBR_param_.dblLink7CogX*sin(q7)) + sin(q5)*(KUKA_LBR_param_.dblLink7CogX*cos(q6)*cos(q7) - KUKA_LBR_param_.dblLink7CogZ*sin(q6) - KUKA_LBR_param_.dblLink7CogY*cos(q6)*sin(q7))) + sin(q3)*(sin(q4)*(KUKA_LBR_param_.dblLink45Len + KUKA_LBR_param_.dblLink7CogZ*cos(q6) + KUKA_LBR_param_.dblLink7CogX*cos(q7)*sin(q6) - KUKA_LBR_param_.dblLink7CogY*sin(q6)*sin(q7)) - cos(q4)*(sin(q5)*(KUKA_LBR_param_.dblLink7CogY*cos(q7) + KUKA_LBR_param_.dblLink7CogX*sin(q7)) + cos(q5)*(-(KUKA_LBR_param_.dblLink7CogX*cos(q6)*cos(q7)) + KUKA_LBR_param_.dblLink7CogZ*sin(q6) + KUKA_LBR_param_.dblLink7CogY*cos(q6)*sin(q7))))) + sin(q1)*(-(sin(q2)*(KUKA_LBR_param_.dblLink23Len + KUKA_LBR_param_.dblLink7CogY*cos(q7)*sin(q4)*sin(q5) + KUKA_LBR_param_.dblLink7CogX*sin(q4)*sin(q5)*sin(q7) + cos(q5)*sin(q4)*(-(KUKA_LBR_param_.dblLink7CogX*cos(q6)*cos(q7)) + KUKA_LBR_param_.dblLink7CogZ*sin(q6) + KUKA_LBR_param_.dblLink7CogY*cos(q6)*sin(q7)) + cos(q4)*(KUKA_LBR_param_.dblLink45Len + KUKA_LBR_param_.dblLink7CogZ*cos(q6) + KUKA_LBR_param_.dblLink7CogX*cos(q7)*sin(q6) - KUKA_LBR_param_.dblLink7CogY*sin(q6)*sin(q7)))) + cos(q2)*(-(sin(q3)*(cos(q5)*(KUKA_LBR_param_.dblLink7CogY*cos(q7) + KUKA_LBR_param_.dblLink7CogX*sin(q7)) + sin(q5)*(KUKA_LBR_param_.dblLink7CogX*cos(q6)*cos(q7) - KUKA_LBR_param_.dblLink7CogZ*sin(q6) - KUKA_LBR_param_.dblLink7CogY*cos(q6)*sin(q7)))) + cos(q3)*(sin(q4)*(KUKA_LBR_param_.dblLink45Len + KUKA_LBR_param_.dblLink7CogZ*cos(q6) + KUKA_LBR_param_.dblLink7CogX*cos(q7)*sin(q6) - KUKA_LBR_param_.dblLink7CogY*sin(q6)*sin(q7)) - cos(q4)*(sin(q5)*(KUKA_LBR_param_.dblLink7CogY*cos(q7) + KUKA_LBR_param_.dblLink7CogX*sin(q7)) + cos(q5)*(-(KUKA_LBR_param_.dblLink7CogX*cos(q6)*cos(q7)) + KUKA_LBR_param_.dblLink7CogZ*sin(q6) + KUKA_LBR_param_.dblLink7CogY*cos(q6)*sin(q7))))))) - 2*KUKA_LBR_param_.dblLink7Mass*(-(cos(q1)*cos(q6)*sin(q3)*sin(q4)) + cos(q5)*sin(q1)*sin(q2)*sin(q4)*sin(q6) + cos(q1)*cos(q3)*sin(q5)*sin(q6) + cos(q4)*(cos(q6)*sin(q1)*sin(q2) + cos(q5)*(cos(q2)*cos(q3)*sin(q1) + cos(q1)*sin(q3))*sin(q6)) - cos(q2)*sin(q1)*(cos(q3)*cos(q6)*sin(q4) + sin(q3)*sin(q5)*sin(q6)))*(KUKA_LBR_param_.dblLink7CogY*cos(q7) + KUKA_LBR_param_.dblLink7CogX*sin(q7))*(sin(q1)*(cos(q3)*(cos(q5)*(KUKA_LBR_param_.dblLink7CogY*cos(q7) + KUKA_LBR_param_.dblLink7CogX*sin(q7)) + sin(q5)*(KUKA_LBR_param_.dblLink7CogX*cos(q6)*cos(q7) - KUKA_LBR_param_.dblLink7CogZ*sin(q6) - KUKA_LBR_param_.dblLink7CogY*cos(q6)*sin(q7))) + sin(q3)*(sin(q4)*(KUKA_LBR_param_.dblLink45Len + KUKA_LBR_param_.dblLink7CogZ*cos(q6) + KUKA_LBR_param_.dblLink7CogX*cos(q7)*sin(q6) - KUKA_LBR_param_.dblLink7CogY*sin(q6)*sin(q7)) - cos(q4)*(sin(q5)*(KUKA_LBR_param_.dblLink7CogY*cos(q7) + KUKA_LBR_param_.dblLink7CogX*sin(q7)) + cos(q5)*(-(KUKA_LBR_param_.dblLink7CogX*cos(q6)*cos(q7)) + KUKA_LBR_param_.dblLink7CogZ*sin(q6) + KUKA_LBR_param_.dblLink7CogY*cos(q6)*sin(q7))))) + cos(q1)*(sin(q2)*(KUKA_LBR_param_.dblLink23Len + KUKA_LBR_param_.dblLink7CogY*cos(q7)*sin(q4)*sin(q5) + KUKA_LBR_param_.dblLink7CogX*sin(q4)*sin(q5)*sin(q7) + cos(q5)*sin(q4)*(-(KUKA_LBR_param_.dblLink7CogX*cos(q6)*cos(q7)) + KUKA_LBR_param_.dblLink7CogZ*sin(q6) + KUKA_LBR_param_.dblLink7CogY*cos(q6)*sin(q7)) + cos(q4)*(KUKA_LBR_param_.dblLink45Len + KUKA_LBR_param_.dblLink7CogZ*cos(q6) + KUKA_LBR_param_.dblLink7CogX*cos(q7)*sin(q6) - KUKA_LBR_param_.dblLink7CogY*sin(q6)*sin(q7))) + cos(q2)*(sin(q3)*(cos(q5)*(KUKA_LBR_param_.dblLink7CogY*cos(q7) + KUKA_LBR_param_.dblLink7CogX*sin(q7)) + sin(q5)*(KUKA_LBR_param_.dblLink7CogX*cos(q6)*cos(q7) - KUKA_LBR_param_.dblLink7CogZ*sin(q6) - KUKA_LBR_param_.dblLink7CogY*cos(q6)*sin(q7))) + cos(q3)*(-(sin(q4)*(KUKA_LBR_param_.dblLink45Len + KUKA_LBR_param_.dblLink7CogZ*cos(q6) + KUKA_LBR_param_.dblLink7CogX*cos(q7)*sin(q6) - KUKA_LBR_param_.dblLink7CogY*sin(q6)*sin(q7))) + cos(q4)*(sin(q5)*(KUKA_LBR_param_.dblLink7CogY*cos(q7) + KUKA_LBR_param_.dblLink7CogX*sin(q7)) + cos(q5)*(-(KUKA_LBR_param_.dblLink7CogX*cos(q6)*cos(q7)) + KUKA_LBR_param_.dblLink7CogZ*sin(q6) + KUKA_LBR_param_.dblLink7CogY*cos(q6)*sin(q7)))))))))/2.0;
dblCoriolisCentrifugalFullRow1Col7 = (q14*(-((cos(q6)*(sin(q1)*sin(q3)*sin(q4) + cos(q1)*(cos(q4)*sin(q2) - cos(q2)*cos(q3)*sin(q4))) - (cos(q5)*(cos(q4)*sin(q1)*sin(q3) - cos(q1)*(cos(q2)*cos(q3)*cos(q4) + sin(q2)*sin(q4))) + (cos(q3)*sin(q1) + cos(q1)*cos(q2)*sin(q3))*sin(q5))*sin(q6))*(KUKA_LBR_param_.dblLink7InertXX*(cos(q6)*(-(cos(q4)*sin(q1)*sin(q2)) + (cos(q2)*cos(q3)*sin(q1) + cos(q1)*sin(q3))*sin(q4)) - (cos(q5)*sin(q1)*sin(q2)*sin(q4) + cos(q1)*(cos(q4)*cos(q5)*sin(q3) + cos(q3)*sin(q5)) + cos(q2)*sin(q1)*(cos(q3)*cos(q4)*cos(q5) - sin(q3)*sin(q5)))*sin(q6)) + KUKA_LBR_param_.dblLink7InertXY*(cos(q6)*(sin(q1)*sin(q3)*sin(q4) + cos(q1)*(cos(q4)*sin(q2) - cos(q2)*cos(q3)*sin(q4))) + (-(sin(q1)*(cos(q4)*cos(q5)*sin(q3) + cos(q3)*sin(q5))) + cos(q1)*(cos(q5)*sin(q2)*sin(q4) + cos(q2)*(cos(q3)*cos(q4)*cos(q5) - sin(q3)*sin(q5))))*sin(q6)))) - (cos(q6)*(cos(q4)*sin(q1)*sin(q2) - (cos(q2)*cos(q3)*sin(q1) + cos(q1)*sin(q3))*sin(q4)) + (cos(q5)*sin(q1)*sin(q2)*sin(q4) + cos(q1)*(cos(q4)*cos(q5)*sin(q3) + cos(q3)*sin(q5)) + cos(q2)*sin(q1)*(cos(q3)*cos(q4)*cos(q5) - sin(q3)*sin(q5)))*sin(q6))*(KUKA_LBR_param_.dblLink7InertXY*(cos(q6)*(-(cos(q4)*sin(q1)*sin(q2)) + (cos(q2)*cos(q3)*sin(q1) + cos(q1)*sin(q3))*sin(q4)) - (cos(q5)*sin(q1)*sin(q2)*sin(q4) + cos(q1)*(cos(q4)*cos(q5)*sin(q3) + cos(q3)*sin(q5)) + cos(q2)*sin(q1)*(cos(q3)*cos(q4)*cos(q5) - sin(q3)*sin(q5)))*sin(q6)) + KUKA_LBR_param_.dblLink7InertYY*(cos(q6)*(sin(q1)*sin(q3)*sin(q4) + cos(q1)*(cos(q4)*sin(q2) - cos(q2)*cos(q3)*sin(q4))) + (-(sin(q1)*(cos(q4)*cos(q5)*sin(q3) + cos(q3)*sin(q5))) + cos(q1)*(cos(q5)*sin(q2)*sin(q4) + cos(q2)*(cos(q3)*cos(q4)*cos(q5) - sin(q3)*sin(q5))))*sin(q6))) - (KUKA_LBR_param_.dblLink7InertXZ*(cos(q6)*(-(cos(q4)*sin(q1)*sin(q2)) + (cos(q2)*cos(q3)*sin(q1) + cos(q1)*sin(q3))*sin(q4)) - (cos(q5)*sin(q1)*sin(q2)*sin(q4) + cos(q1)*(cos(q4)*cos(q5)*sin(q3) + cos(q3)*sin(q5)) + cos(q2)*sin(q1)*(cos(q3)*cos(q4)*cos(q5) - sin(q3)*sin(q5)))*sin(q6)) + KUKA_LBR_param_.dblLink7InertYZ*(cos(q6)*(sin(q1)*sin(q3)*sin(q4) + cos(q1)*(cos(q4)*sin(q2) - cos(q2)*cos(q3)*sin(q4))) + (-(sin(q1)*(cos(q4)*cos(q5)*sin(q3) + cos(q3)*sin(q5))) + cos(q1)*(cos(q5)*sin(q2)*sin(q4) + cos(q2)*(cos(q3)*cos(q4)*cos(q5) - sin(q3)*sin(q5))))*sin(q6)))*(cos(q2)*(cos(q4)*cos(q6) + cos(q5)*sin(q4)*sin(q6)) + sin(q2)*(sin(q3)*sin(q5)*sin(q6) + cos(q3)*(cos(q6)*sin(q4) - cos(q4)*cos(q5)*sin(q6)))) - (cos(q6)*(-(cos(q4)*sin(q1)*sin(q2)) + (cos(q2)*cos(q3)*sin(q1) + cos(q1)*sin(q3))*sin(q4)) - (cos(q5)*sin(q1)*sin(q2)*sin(q4) + cos(q1)*(cos(q4)*cos(q5)*sin(q3) + cos(q3)*sin(q5)) + cos(q2)*sin(q1)*(cos(q3)*cos(q4)*cos(q5) - sin(q3)*sin(q5)))*sin(q6))*(KUKA_LBR_param_.dblLink7InertXX*(cos(q6)*(sin(q1)*sin(q3)*sin(q4) + cos(q1)*(cos(q4)*sin(q2) - cos(q2)*cos(q3)*sin(q4))) - (cos(q5)*(cos(q4)*sin(q1)*sin(q3) - cos(q1)*(cos(q2)*cos(q3)*cos(q4) + sin(q2)*sin(q4))) + (cos(q3)*sin(q1) + cos(q1)*cos(q2)*sin(q3))*sin(q5))*sin(q6)) + KUKA_LBR_param_.dblLink7InertXY*(cos(q6)*(cos(q4)*sin(q1)*sin(q2) - (cos(q2)*cos(q3)*sin(q1) + cos(q1)*sin(q3))*sin(q4)) + (cos(q5)*sin(q1)*sin(q2)*sin(q4) + cos(q1)*(cos(q4)*cos(q5)*sin(q3) + cos(q3)*sin(q5)) + cos(q2)*sin(q1)*(cos(q3)*cos(q4)*cos(q5) - sin(q3)*sin(q5)))*sin(q6)) + KUKA_LBR_param_.dblLink7InertXZ*(cos(q2)*(cos(q4)*cos(q6) + cos(q5)*sin(q4)*sin(q6)) + sin(q2)*(sin(q3)*sin(q5)*sin(q6) + cos(q3)*(cos(q6)*sin(q4) - cos(q4)*cos(q5)*sin(q6))))) - (cos(q6)*(sin(q1)*sin(q3)*sin(q4) + cos(q1)*(cos(q4)*sin(q2) - cos(q2)*cos(q3)*sin(q4))) + (-(sin(q1)*(cos(q4)*cos(q5)*sin(q3) + cos(q3)*sin(q5))) + cos(q1)*(cos(q5)*sin(q2)*sin(q4) + cos(q2)*(cos(q3)*cos(q4)*cos(q5) - sin(q3)*sin(q5))))*sin(q6))*(KUKA_LBR_param_.dblLink7InertXY*(cos(q6)*(sin(q1)*sin(q3)*sin(q4) + cos(q1)*(cos(q4)*sin(q2) - cos(q2)*cos(q3)*sin(q4))) - (cos(q5)*(cos(q4)*sin(q1)*sin(q3) - cos(q1)*(cos(q2)*cos(q3)*cos(q4) + sin(q2)*sin(q4))) + (cos(q3)*sin(q1) + cos(q1)*cos(q2)*sin(q3))*sin(q5))*sin(q6)) + KUKA_LBR_param_.dblLink7InertYY*(cos(q6)*(cos(q4)*sin(q1)*sin(q2) - (cos(q2)*cos(q3)*sin(q1) + cos(q1)*sin(q3))*sin(q4)) + (cos(q5)*sin(q1)*sin(q2)*sin(q4) + cos(q1)*(cos(q4)*cos(q5)*sin(q3) + cos(q3)*sin(q5)) + cos(q2)*sin(q1)*(cos(q3)*cos(q4)*cos(q5) - sin(q3)*sin(q5)))*sin(q6)) + KUKA_LBR_param_.dblLink7InertYZ*(cos(q2)*(cos(q4)*cos(q6) + cos(q5)*sin(q4)*sin(q6)) + sin(q2)*(sin(q3)*sin(q5)*sin(q6) + cos(q3)*(cos(q6)*sin(q4) - cos(q4)*cos(q5)*sin(q6))))) - 2*KUKA_LBR_param_.dblLink7Mass*(cos(q1)*(cos(q3)*(-(cos(q6)*sin(q5)*(KUKA_LBR_param_.dblLink7CogY*cos(q7) + KUKA_LBR_param_.dblLink7CogX*sin(q7))) + cos(q5)*(KUKA_LBR_param_.dblLink7CogX*cos(q7) - KUKA_LBR_param_.dblLink7CogY*sin(q7))) - sin(q3)*(sin(q4)*sin(q6)*(KUKA_LBR_param_.dblLink7CogY*cos(q7) + KUKA_LBR_param_.dblLink7CogX*sin(q7)) + cos(q4)*(cos(q5)*cos(q6)*(KUKA_LBR_param_.dblLink7CogY*cos(q7) + KUKA_LBR_param_.dblLink7CogX*sin(q7)) + sin(q5)*(KUKA_LBR_param_.dblLink7CogX*cos(q7) - KUKA_LBR_param_.dblLink7CogY*sin(q7))))) + sin(q1)*(-(sin(q2)*(KUKA_LBR_param_.dblLink7CogX*cos(q7)*sin(q4)*sin(q5) - KUKA_LBR_param_.dblLink7CogY*sin(q4)*sin(q5)*sin(q7) + cos(q5)*cos(q6)*sin(q4)*(KUKA_LBR_param_.dblLink7CogY*cos(q7) + KUKA_LBR_param_.dblLink7CogX*sin(q7)) - cos(q4)*sin(q6)*(KUKA_LBR_param_.dblLink7CogY*cos(q7) + KUKA_LBR_param_.dblLink7CogX*sin(q7)))) + cos(q2)*(sin(q3)*(cos(q6)*sin(q5)*(KUKA_LBR_param_.dblLink7CogY*cos(q7) + KUKA_LBR_param_.dblLink7CogX*sin(q7)) + cos(q5)*(-(KUKA_LBR_param_.dblLink7CogX*cos(q7)) + KUKA_LBR_param_.dblLink7CogY*sin(q7))) - cos(q3)*(sin(q4)*sin(q6)*(KUKA_LBR_param_.dblLink7CogY*cos(q7) + KUKA_LBR_param_.dblLink7CogX*sin(q7)) + cos(q4)*(cos(q5)*cos(q6)*(KUKA_LBR_param_.dblLink7CogY*cos(q7) + KUKA_LBR_param_.dblLink7CogX*sin(q7)) + sin(q5)*(KUKA_LBR_param_.dblLink7CogX*cos(q7) - KUKA_LBR_param_.dblLink7CogY*sin(q7)))))))*(sin(q1)*(cos(q3)*(cos(q6)*sin(q5)*(KUKA_LBR_param_.dblLink7CogY*cos(q7) + KUKA_LBR_param_.dblLink7CogX*sin(q7)) + cos(q5)*(-(KUKA_LBR_param_.dblLink7CogX*cos(q7)) + KUKA_LBR_param_.dblLink7CogY*sin(q7))) + sin(q3)*(sin(q4)*sin(q6)*(KUKA_LBR_param_.dblLink7CogY*cos(q7) + KUKA_LBR_param_.dblLink7CogX*sin(q7)) + cos(q4)*(cos(q5)*cos(q6)*(KUKA_LBR_param_.dblLink7CogY*cos(q7) + KUKA_LBR_param_.dblLink7CogX*sin(q7)) + sin(q5)*(KUKA_LBR_param_.dblLink7CogX*cos(q7) - KUKA_LBR_param_.dblLink7CogY*sin(q7))))) - cos(q1)*(sin(q2)*(cos(q7)*(KUKA_LBR_param_.dblLink7CogX*sin(q4)*sin(q5) - KUKA_LBR_param_.dblLink7CogY*cos(q4)*sin(q6)) - (KUKA_LBR_param_.dblLink7CogY*sin(q4)*sin(q5) + KUKA_LBR_param_.dblLink7CogX*cos(q4)*sin(q6))*sin(q7) + cos(q5)*cos(q6)*sin(q4)*(KUKA_LBR_param_.dblLink7CogY*cos(q7) + KUKA_LBR_param_.dblLink7CogX*sin(q7))) + cos(q2)*(sin(q3)*(-(cos(q6)*sin(q5)*(KUKA_LBR_param_.dblLink7CogY*cos(q7) + KUKA_LBR_param_.dblLink7CogX*sin(q7))) + cos(q5)*(KUKA_LBR_param_.dblLink7CogX*cos(q7) - KUKA_LBR_param_.dblLink7CogY*sin(q7))) + cos(q3)*(sin(q4)*sin(q6)*(KUKA_LBR_param_.dblLink7CogY*cos(q7) + KUKA_LBR_param_.dblLink7CogX*sin(q7)) + cos(q4)*(cos(q5)*cos(q6)*(KUKA_LBR_param_.dblLink7CogY*cos(q7) + KUKA_LBR_param_.dblLink7CogX*sin(q7)) + sin(q5)*(KUKA_LBR_param_.dblLink7CogX*cos(q7) - KUKA_LBR_param_.dblLink7CogY*sin(q7))))))) - 2*KUKA_LBR_param_.dblLink7Mass*(sin(q1)*(cos(q3)*(-(cos(q6)*sin(q5)*(KUKA_LBR_param_.dblLink7CogY*cos(q7) + KUKA_LBR_param_.dblLink7CogX*sin(q7))) + cos(q5)*(KUKA_LBR_param_.dblLink7CogX*cos(q7) - KUKA_LBR_param_.dblLink7CogY*sin(q7))) - sin(q3)*(sin(q4)*sin(q6)*(KUKA_LBR_param_.dblLink7CogY*cos(q7) + KUKA_LBR_param_.dblLink7CogX*sin(q7)) + cos(q4)*(cos(q5)*cos(q6)*(KUKA_LBR_param_.dblLink7CogY*cos(q7) + KUKA_LBR_param_.dblLink7CogX*sin(q7)) + sin(q5)*(KUKA_LBR_param_.dblLink7CogX*cos(q7) - KUKA_LBR_param_.dblLink7CogY*sin(q7))))) + cos(q1)*(sin(q2)*(cos(q7)*(KUKA_LBR_param_.dblLink7CogX*sin(q4)*sin(q5) - KUKA_LBR_param_.dblLink7CogY*cos(q4)*sin(q6)) - (KUKA_LBR_param_.dblLink7CogY*sin(q4)*sin(q5) + KUKA_LBR_param_.dblLink7CogX*cos(q4)*sin(q6))*sin(q7) + cos(q5)*cos(q6)*sin(q4)*(KUKA_LBR_param_.dblLink7CogY*cos(q7) + KUKA_LBR_param_.dblLink7CogX*sin(q7))) + cos(q2)*(sin(q3)*(-(cos(q6)*sin(q5)*(KUKA_LBR_param_.dblLink7CogY*cos(q7) + KUKA_LBR_param_.dblLink7CogX*sin(q7))) + cos(q5)*(KUKA_LBR_param_.dblLink7CogX*cos(q7) - KUKA_LBR_param_.dblLink7CogY*sin(q7))) + cos(q3)*(sin(q4)*sin(q6)*(KUKA_LBR_param_.dblLink7CogY*cos(q7) + KUKA_LBR_param_.dblLink7CogX*sin(q7)) + cos(q4)*(cos(q5)*cos(q6)*(KUKA_LBR_param_.dblLink7CogY*cos(q7) + KUKA_LBR_param_.dblLink7CogX*sin(q7)) + sin(q5)*(KUKA_LBR_param_.dblLink7CogX*cos(q7) - KUKA_LBR_param_.dblLink7CogY*sin(q7)))))))*(cos(q1)*(cos(q3)*(-(cos(q6)*sin(q5)*(KUKA_LBR_param_.dblLink7CogY*cos(q7) + KUKA_LBR_param_.dblLink7CogX*sin(q7))) + cos(q5)*(KUKA_LBR_param_.dblLink7CogX*cos(q7) - KUKA_LBR_param_.dblLink7CogY*sin(q7))) - sin(q3)*(sin(q4)*sin(q6)*(KUKA_LBR_param_.dblLink7CogY*cos(q7) + KUKA_LBR_param_.dblLink7CogX*sin(q7)) + cos(q4)*(cos(q5)*cos(q6)*(KUKA_LBR_param_.dblLink7CogY*cos(q7) + KUKA_LBR_param_.dblLink7CogX*sin(q7)) + sin(q5)*(KUKA_LBR_param_.dblLink7CogX*cos(q7) - KUKA_LBR_param_.dblLink7CogY*sin(q7))))) - sin(q1)*(sin(q2)*(cos(q7)*(KUKA_LBR_param_.dblLink7CogX*sin(q4)*sin(q5) - KUKA_LBR_param_.dblLink7CogY*cos(q4)*sin(q6)) - (KUKA_LBR_param_.dblLink7CogY*sin(q4)*sin(q5) + KUKA_LBR_param_.dblLink7CogX*cos(q4)*sin(q6))*sin(q7) + cos(q5)*cos(q6)*sin(q4)*(KUKA_LBR_param_.dblLink7CogY*cos(q7) + KUKA_LBR_param_.dblLink7CogX*sin(q7))) + cos(q2)*(sin(q3)*(-(cos(q6)*sin(q5)*(KUKA_LBR_param_.dblLink7CogY*cos(q7) + KUKA_LBR_param_.dblLink7CogX*sin(q7))) + cos(q5)*(KUKA_LBR_param_.dblLink7CogX*cos(q7) - KUKA_LBR_param_.dblLink7CogY*sin(q7))) + cos(q3)*(sin(q4)*sin(q6)*(KUKA_LBR_param_.dblLink7CogY*cos(q7) + KUKA_LBR_param_.dblLink7CogX*sin(q7)) + cos(q4)*(cos(q5)*cos(q6)*(KUKA_LBR_param_.dblLink7CogY*cos(q7) + KUKA_LBR_param_.dblLink7CogX*sin(q7)) + sin(q5)*(KUKA_LBR_param_.dblLink7CogX*cos(q7) - KUKA_LBR_param_.dblLink7CogY*sin(q7))))))) - 2*KUKA_LBR_param_.dblLink7Mass*(-(sin(q1)*(cos(q3)*(cos(q6)*sin(q5)*(KUKA_LBR_param_.dblLink7CogY*cos(q7) + KUKA_LBR_param_.dblLink7CogX*sin(q7)) + cos(q5)*(-(KUKA_LBR_param_.dblLink7CogX*cos(q7)) + KUKA_LBR_param_.dblLink7CogY*sin(q7))) + sin(q3)*(sin(q4)*sin(q6)*(KUKA_LBR_param_.dblLink7CogY*cos(q7) + KUKA_LBR_param_.dblLink7CogX*sin(q7)) + cos(q4)*(cos(q5)*cos(q6)*(KUKA_LBR_param_.dblLink7CogY*cos(q7) + KUKA_LBR_param_.dblLink7CogX*sin(q7)) + sin(q5)*(KUKA_LBR_param_.dblLink7CogX*cos(q7) - KUKA_LBR_param_.dblLink7CogY*sin(q7)))))) + cos(q1)*(sin(q2)*(cos(q7)*(KUKA_LBR_param_.dblLink7CogX*sin(q4)*sin(q5) - KUKA_LBR_param_.dblLink7CogY*cos(q4)*sin(q6)) - (KUKA_LBR_param_.dblLink7CogY*sin(q4)*sin(q5) + KUKA_LBR_param_.dblLink7CogX*cos(q4)*sin(q6))*sin(q7) + cos(q5)*cos(q6)*sin(q4)*(KUKA_LBR_param_.dblLink7CogY*cos(q7) + KUKA_LBR_param_.dblLink7CogX*sin(q7))) + cos(q2)*(sin(q3)*(-(cos(q6)*sin(q5)*(KUKA_LBR_param_.dblLink7CogY*cos(q7) + KUKA_LBR_param_.dblLink7CogX*sin(q7))) + cos(q5)*(KUKA_LBR_param_.dblLink7CogX*cos(q7) - KUKA_LBR_param_.dblLink7CogY*sin(q7))) + cos(q3)*(sin(q4)*sin(q6)*(KUKA_LBR_param_.dblLink7CogY*cos(q7) + KUKA_LBR_param_.dblLink7CogX*sin(q7)) + cos(q4)*(cos(q5)*cos(q6)*(KUKA_LBR_param_.dblLink7CogY*cos(q7) + KUKA_LBR_param_.dblLink7CogX*sin(q7)) + sin(q5)*(KUKA_LBR_param_.dblLink7CogX*cos(q7) - KUKA_LBR_param_.dblLink7CogY*sin(q7)))))))*(cos(q1)*(cos(q3)*(cos(q6)*sin(q5)*(KUKA_LBR_param_.dblLink7CogY*cos(q7) + KUKA_LBR_param_.dblLink7CogX*sin(q7)) + cos(q5)*(-(KUKA_LBR_param_.dblLink7CogX*cos(q7)) + KUKA_LBR_param_.dblLink7CogY*sin(q7))) + sin(q3)*(sin(q4)*sin(q6)*(KUKA_LBR_param_.dblLink7CogY*cos(q7) + KUKA_LBR_param_.dblLink7CogX*sin(q7)) + cos(q4)*(cos(q5)*cos(q6)*(KUKA_LBR_param_.dblLink7CogY*cos(q7) + KUKA_LBR_param_.dblLink7CogX*sin(q7)) + sin(q5)*(KUKA_LBR_param_.dblLink7CogX*cos(q7) - KUKA_LBR_param_.dblLink7CogY*sin(q7))))) + sin(q1)*(sin(q2)*(cos(q7)*(KUKA_LBR_param_.dblLink7CogX*sin(q4)*sin(q5) - KUKA_LBR_param_.dblLink7CogY*cos(q4)*sin(q6)) - (KUKA_LBR_param_.dblLink7CogY*sin(q4)*sin(q5) + KUKA_LBR_param_.dblLink7CogX*cos(q4)*sin(q6))*sin(q7) + cos(q5)*cos(q6)*sin(q4)*(KUKA_LBR_param_.dblLink7CogY*cos(q7) + KUKA_LBR_param_.dblLink7CogX*sin(q7))) + cos(q2)*(sin(q3)*(-(cos(q6)*sin(q5)*(KUKA_LBR_param_.dblLink7CogY*cos(q7) + KUKA_LBR_param_.dblLink7CogX*sin(q7))) + cos(q5)*(KUKA_LBR_param_.dblLink7CogX*cos(q7) - KUKA_LBR_param_.dblLink7CogY*sin(q7))) + cos(q3)*(sin(q4)*sin(q6)*(KUKA_LBR_param_.dblLink7CogY*cos(q7) + KUKA_LBR_param_.dblLink7CogX*sin(q7)) + cos(q4)*(cos(q5)*cos(q6)*(KUKA_LBR_param_.dblLink7CogY*cos(q7) + KUKA_LBR_param_.dblLink7CogX*sin(q7)) + sin(q5)*(KUKA_LBR_param_.dblLink7CogX*cos(q7) - KUKA_LBR_param_.dblLink7CogY*sin(q7))))))) + 2*KUKA_LBR_param_.dblLink7Mass*(cos(q1)*(cos(q3)*(cos(q6)*sin(q5)*(KUKA_LBR_param_.dblLink7CogY*cos(q7) + KUKA_LBR_param_.dblLink7CogX*sin(q7)) + cos(q5)*(-(KUKA_LBR_param_.dblLink7CogX*cos(q7)) + KUKA_LBR_param_.dblLink7CogY*sin(q7))) + sin(q3)*(sin(q4)*sin(q6)*(KUKA_LBR_param_.dblLink7CogY*cos(q7) + KUKA_LBR_param_.dblLink7CogX*sin(q7)) + cos(q4)*(cos(q5)*cos(q6)*(KUKA_LBR_param_.dblLink7CogY*cos(q7) + KUKA_LBR_param_.dblLink7CogX*sin(q7)) + sin(q5)*(KUKA_LBR_param_.dblLink7CogX*cos(q7) - KUKA_LBR_param_.dblLink7CogY*sin(q7))))) + sin(q1)*(sin(q2)*(cos(q7)*(KUKA_LBR_param_.dblLink7CogX*sin(q4)*sin(q5) - KUKA_LBR_param_.dblLink7CogY*cos(q4)*sin(q6)) - (KUKA_LBR_param_.dblLink7CogY*sin(q4)*sin(q5) + KUKA_LBR_param_.dblLink7CogX*cos(q4)*sin(q6))*sin(q7) + cos(q5)*cos(q6)*sin(q4)*(KUKA_LBR_param_.dblLink7CogY*cos(q7) + KUKA_LBR_param_.dblLink7CogX*sin(q7))) + cos(q2)*(sin(q3)*(-(cos(q6)*sin(q5)*(KUKA_LBR_param_.dblLink7CogY*cos(q7) + KUKA_LBR_param_.dblLink7CogX*sin(q7))) + cos(q5)*(KUKA_LBR_param_.dblLink7CogX*cos(q7) - KUKA_LBR_param_.dblLink7CogY*sin(q7))) + cos(q3)*(sin(q4)*sin(q6)*(KUKA_LBR_param_.dblLink7CogY*cos(q7) + KUKA_LBR_param_.dblLink7CogX*sin(q7)) + cos(q4)*(cos(q5)*cos(q6)*(KUKA_LBR_param_.dblLink7CogY*cos(q7) + KUKA_LBR_param_.dblLink7CogX*sin(q7)) + sin(q5)*(KUKA_LBR_param_.dblLink7CogX*cos(q7) - KUKA_LBR_param_.dblLink7CogY*sin(q7)))))))*(sin(q1)*(cos(q3)*(-(cos(q6)*sin(q5)*(KUKA_LBR_param_.dblLink7CogY*cos(q7) + KUKA_LBR_param_.dblLink7CogX*sin(q7))) + cos(q5)*(KUKA_LBR_param_.dblLink7CogX*cos(q7) - KUKA_LBR_param_.dblLink7CogY*sin(q7))) - sin(q3)*(sin(q4)*sin(q6)*(KUKA_LBR_param_.dblLink7CogY*cos(q7) + KUKA_LBR_param_.dblLink7CogX*sin(q7)) + cos(q4)*(cos(q5)*cos(q6)*(KUKA_LBR_param_.dblLink7CogY*cos(q7) + KUKA_LBR_param_.dblLink7CogX*sin(q7)) + sin(q5)*(KUKA_LBR_param_.dblLink7CogX*cos(q7) - KUKA_LBR_param_.dblLink7CogY*sin(q7))))) + cos(q1)*(sin(q2)*(KUKA_LBR_param_.dblLink7CogX*cos(q7)*sin(q4)*sin(q5) - KUKA_LBR_param_.dblLink7CogY*sin(q4)*sin(q5)*sin(q7) + cos(q5)*cos(q6)*sin(q4)*(KUKA_LBR_param_.dblLink7CogY*cos(q7) + KUKA_LBR_param_.dblLink7CogX*sin(q7)) - cos(q4)*sin(q6)*(KUKA_LBR_param_.dblLink7CogY*cos(q7) + KUKA_LBR_param_.dblLink7CogX*sin(q7))) + cos(q2)*(sin(q3)*(-(cos(q6)*sin(q5)*(KUKA_LBR_param_.dblLink7CogY*cos(q7) + KUKA_LBR_param_.dblLink7CogX*sin(q7))) + cos(q5)*(KUKA_LBR_param_.dblLink7CogX*cos(q7) - KUKA_LBR_param_.dblLink7CogY*sin(q7))) + cos(q3)*(sin(q4)*sin(q6)*(KUKA_LBR_param_.dblLink7CogY*cos(q7) + KUKA_LBR_param_.dblLink7CogX*sin(q7)) + cos(q4)*(cos(q5)*cos(q6)*(KUKA_LBR_param_.dblLink7CogY*cos(q7) + KUKA_LBR_param_.dblLink7CogX*sin(q7)) + sin(q5)*(KUKA_LBR_param_.dblLink7CogX*cos(q7) - KUKA_LBR_param_.dblLink7CogY*sin(q7))))))) - 2*KUKA_LBR_param_.dblLink7Mass*(sin(q1)*(cos(q3)*(cos(q5)*(KUKA_LBR_param_.dblLink7CogY*cos(q7) + KUKA_LBR_param_.dblLink7CogX*sin(q7)) + cos(q6)*sin(q5)*(KUKA_LBR_param_.dblLink7CogX*cos(q7) - KUKA_LBR_param_.dblLink7CogY*sin(q7))) + sin(q3)*(sin(q4)*sin(q6)*(KUKA_LBR_param_.dblLink7CogX*cos(q7) - KUKA_LBR_param_.dblLink7CogY*sin(q7)) + cos(q4)*(-(sin(q5)*(KUKA_LBR_param_.dblLink7CogY*cos(q7) + KUKA_LBR_param_.dblLink7CogX*sin(q7))) + cos(q5)*cos(q6)*(KUKA_LBR_param_.dblLink7CogX*cos(q7) - KUKA_LBR_param_.dblLink7CogY*sin(q7))))) + cos(q1)*(sin(q2)*(KUKA_LBR_param_.dblLink7CogY*cos(q7)*sin(q4)*sin(q5) + KUKA_LBR_param_.dblLink7CogX*cos(q4)*cos(q7)*sin(q6) + KUKA_LBR_param_.dblLink7CogX*sin(q4)*sin(q5)*sin(q7) - KUKA_LBR_param_.dblLink7CogY*cos(q4)*sin(q6)*sin(q7) - cos(q5)*cos(q6)*sin(q4)*(KUKA_LBR_param_.dblLink7CogX*cos(q7) - KUKA_LBR_param_.dblLink7CogY*sin(q7))) + cos(q2)*(sin(q3)*(cos(q5)*(KUKA_LBR_param_.dblLink7CogY*cos(q7) + KUKA_LBR_param_.dblLink7CogX*sin(q7)) + cos(q6)*sin(q5)*(KUKA_LBR_param_.dblLink7CogX*cos(q7) - KUKA_LBR_param_.dblLink7CogY*sin(q7))) + cos(q3)*(sin(q4)*sin(q6)*(-(KUKA_LBR_param_.dblLink7CogX*cos(q7)) + KUKA_LBR_param_.dblLink7CogY*sin(q7)) + cos(q4)*(-(KUKA_LBR_param_.dblLink7CogX*cos(q5)*cos(q6)*cos(q7)) + KUKA_LBR_param_.dblLink7CogY*cos(q7)*sin(q5) + KUKA_LBR_param_.dblLink7CogY*cos(q5)*cos(q6)*sin(q7) + KUKA_LBR_param_.dblLink7CogX*sin(q5)*sin(q7))))))*(cos(q1)*(cos(q3)*(cos(q5)*(KUKA_LBR_param_.dblLink7CogY*cos(q7) + KUKA_LBR_param_.dblLink7CogX*sin(q7)) + sin(q5)*(KUKA_LBR_param_.dblLink7CogX*cos(q6)*cos(q7) - KUKA_LBR_param_.dblLink7CogZ*sin(q6) - KUKA_LBR_param_.dblLink7CogY*cos(q6)*sin(q7))) + sin(q3)*(sin(q4)*(KUKA_LBR_param_.dblLink45Len + KUKA_LBR_param_.dblLink7CogZ*cos(q6) + KUKA_LBR_param_.dblLink7CogX*cos(q7)*sin(q6) - KUKA_LBR_param_.dblLink7CogY*sin(q6)*sin(q7)) - cos(q4)*(sin(q5)*(KUKA_LBR_param_.dblLink7CogY*cos(q7) + KUKA_LBR_param_.dblLink7CogX*sin(q7)) + cos(q5)*(-(KUKA_LBR_param_.dblLink7CogX*cos(q6)*cos(q7)) + KUKA_LBR_param_.dblLink7CogZ*sin(q6) + KUKA_LBR_param_.dblLink7CogY*cos(q6)*sin(q7))))) + sin(q1)*(-(sin(q2)*(KUKA_LBR_param_.dblLink23Len + KUKA_LBR_param_.dblLink7CogY*cos(q7)*sin(q4)*sin(q5) + KUKA_LBR_param_.dblLink7CogX*sin(q4)*sin(q5)*sin(q7) + cos(q5)*sin(q4)*(-(KUKA_LBR_param_.dblLink7CogX*cos(q6)*cos(q7)) + KUKA_LBR_param_.dblLink7CogZ*sin(q6) + KUKA_LBR_param_.dblLink7CogY*cos(q6)*sin(q7)) + cos(q4)*(KUKA_LBR_param_.dblLink45Len + KUKA_LBR_param_.dblLink7CogZ*cos(q6) + KUKA_LBR_param_.dblLink7CogX*cos(q7)*sin(q6) - KUKA_LBR_param_.dblLink7CogY*sin(q6)*sin(q7)))) + cos(q2)*(-(sin(q3)*(cos(q5)*(KUKA_LBR_param_.dblLink7CogY*cos(q7) + KUKA_LBR_param_.dblLink7CogX*sin(q7)) + sin(q5)*(KUKA_LBR_param_.dblLink7CogX*cos(q6)*cos(q7) - KUKA_LBR_param_.dblLink7CogZ*sin(q6) - KUKA_LBR_param_.dblLink7CogY*cos(q6)*sin(q7)))) + cos(q3)*(sin(q4)*(KUKA_LBR_param_.dblLink45Len + KUKA_LBR_param_.dblLink7CogZ*cos(q6) + KUKA_LBR_param_.dblLink7CogX*cos(q7)*sin(q6) - KUKA_LBR_param_.dblLink7CogY*sin(q6)*sin(q7)) - cos(q4)*(sin(q5)*(KUKA_LBR_param_.dblLink7CogY*cos(q7) + KUKA_LBR_param_.dblLink7CogX*sin(q7)) + cos(q5)*(-(KUKA_LBR_param_.dblLink7CogX*cos(q6)*cos(q7)) + KUKA_LBR_param_.dblLink7CogZ*sin(q6) + KUKA_LBR_param_.dblLink7CogY*cos(q6)*sin(q7))))))) + 2*KUKA_LBR_param_.dblLink7Mass*(cos(q1)*(cos(q3)*(cos(q5)*(KUKA_LBR_param_.dblLink7CogY*cos(q7) + KUKA_LBR_param_.dblLink7CogX*sin(q7)) + cos(q6)*sin(q5)*(KUKA_LBR_param_.dblLink7CogX*cos(q7) - KUKA_LBR_param_.dblLink7CogY*sin(q7))) + sin(q3)*(sin(q4)*sin(q6)*(KUKA_LBR_param_.dblLink7CogX*cos(q7) - KUKA_LBR_param_.dblLink7CogY*sin(q7)) + cos(q4)*(-(sin(q5)*(KUKA_LBR_param_.dblLink7CogY*cos(q7) + KUKA_LBR_param_.dblLink7CogX*sin(q7))) + cos(q5)*cos(q6)*(KUKA_LBR_param_.dblLink7CogX*cos(q7) - KUKA_LBR_param_.dblLink7CogY*sin(q7))))) + sin(q1)*(sin(q2)*(-(cos(q7)*(KUKA_LBR_param_.dblLink7CogY*sin(q4)*sin(q5) + KUKA_LBR_param_.dblLink7CogX*cos(q4)*sin(q6))) + (-(KUKA_LBR_param_.dblLink7CogX*sin(q4)*sin(q5)) + KUKA_LBR_param_.dblLink7CogY*cos(q4)*sin(q6))*sin(q7) + cos(q5)*cos(q6)*sin(q4)*(KUKA_LBR_param_.dblLink7CogX*cos(q7) - KUKA_LBR_param_.dblLink7CogY*sin(q7))) + cos(q2)*(-(sin(q3)*(cos(q5)*(KUKA_LBR_param_.dblLink7CogY*cos(q7) + KUKA_LBR_param_.dblLink7CogX*sin(q7)) + cos(q6)*sin(q5)*(KUKA_LBR_param_.dblLink7CogX*cos(q7) - KUKA_LBR_param_.dblLink7CogY*sin(q7)))) + cos(q3)*(sin(q4)*sin(q6)*(KUKA_LBR_param_.dblLink7CogX*cos(q7) - KUKA_LBR_param_.dblLink7CogY*sin(q7)) + cos(q4)*(-(sin(q5)*(KUKA_LBR_param_.dblLink7CogY*cos(q7) + KUKA_LBR_param_.dblLink7CogX*sin(q7))) + cos(q5)*cos(q6)*(KUKA_LBR_param_.dblLink7CogX*cos(q7) - KUKA_LBR_param_.dblLink7CogY*sin(q7)))))))*(sin(q1)*(cos(q3)*(cos(q5)*(KUKA_LBR_param_.dblLink7CogY*cos(q7) + KUKA_LBR_param_.dblLink7CogX*sin(q7)) + sin(q5)*(KUKA_LBR_param_.dblLink7CogX*cos(q6)*cos(q7) - KUKA_LBR_param_.dblLink7CogZ*sin(q6) - KUKA_LBR_param_.dblLink7CogY*cos(q6)*sin(q7))) + sin(q3)*(sin(q4)*(KUKA_LBR_param_.dblLink45Len + KUKA_LBR_param_.dblLink7CogZ*cos(q6) + KUKA_LBR_param_.dblLink7CogX*cos(q7)*sin(q6) - KUKA_LBR_param_.dblLink7CogY*sin(q6)*sin(q7)) - cos(q4)*(sin(q5)*(KUKA_LBR_param_.dblLink7CogY*cos(q7) + KUKA_LBR_param_.dblLink7CogX*sin(q7)) + cos(q5)*(-(KUKA_LBR_param_.dblLink7CogX*cos(q6)*cos(q7)) + KUKA_LBR_param_.dblLink7CogZ*sin(q6) + KUKA_LBR_param_.dblLink7CogY*cos(q6)*sin(q7))))) + cos(q1)*(sin(q2)*(KUKA_LBR_param_.dblLink23Len + KUKA_LBR_param_.dblLink7CogY*cos(q7)*sin(q4)*sin(q5) + KUKA_LBR_param_.dblLink7CogX*sin(q4)*sin(q5)*sin(q7) + cos(q5)*sin(q4)*(-(KUKA_LBR_param_.dblLink7CogX*cos(q6)*cos(q7)) + KUKA_LBR_param_.dblLink7CogZ*sin(q6) + KUKA_LBR_param_.dblLink7CogY*cos(q6)*sin(q7)) + cos(q4)*(KUKA_LBR_param_.dblLink45Len + KUKA_LBR_param_.dblLink7CogZ*cos(q6) + KUKA_LBR_param_.dblLink7CogX*cos(q7)*sin(q6) - KUKA_LBR_param_.dblLink7CogY*sin(q6)*sin(q7))) + cos(q2)*(sin(q3)*(cos(q5)*(KUKA_LBR_param_.dblLink7CogY*cos(q7) + KUKA_LBR_param_.dblLink7CogX*sin(q7)) + sin(q5)*(KUKA_LBR_param_.dblLink7CogX*cos(q6)*cos(q7) - KUKA_LBR_param_.dblLink7CogZ*sin(q6) - KUKA_LBR_param_.dblLink7CogY*cos(q6)*sin(q7))) + cos(q3)*(-(sin(q4)*(KUKA_LBR_param_.dblLink45Len + KUKA_LBR_param_.dblLink7CogZ*cos(q6) + KUKA_LBR_param_.dblLink7CogX*cos(q7)*sin(q6) - KUKA_LBR_param_.dblLink7CogY*sin(q6)*sin(q7))) + cos(q4)*(sin(q5)*(KUKA_LBR_param_.dblLink7CogY*cos(q7) + KUKA_LBR_param_.dblLink7CogX*sin(q7)) + cos(q5)*(-(KUKA_LBR_param_.dblLink7CogX*cos(q6)*cos(q7)) + KUKA_LBR_param_.dblLink7CogZ*sin(q6) + KUKA_LBR_param_.dblLink7CogY*cos(q6)*sin(q7)))))))))/2.0;
dblCoriolisCentrifugalFullRow2Col1 = (q14*((-(KUKA_LBR_param_.dblLink7InertXX*cos(q1)) - KUKA_LBR_param_.dblLink7InertXY*sin(q1))*(cos(q6)*(sin(q1)*sin(q3)*sin(q4) + cos(q1)*(cos(q4)*sin(q2) - cos(q2)*cos(q3)*sin(q4))) - (cos(q5)*(cos(q4)*sin(q1)*sin(q3) - cos(q1)*(cos(q2)*cos(q3)*cos(q4) + sin(q2)*sin(q4))) + (cos(q3)*sin(q1) + cos(q1)*cos(q2)*sin(q3))*sin(q5))*sin(q6)) + (KUKA_LBR_param_.dblLink7InertXY*cos(q1) - KUKA_LBR_param_.dblLink7InertXX*sin(q1))*(cos(q6)*(-(cos(q4)*sin(q1)*sin(q2)) + (cos(q2)*cos(q3)*sin(q1) + cos(q1)*sin(q3))*sin(q4)) - (cos(q5)*sin(q1)*sin(q2)*sin(q4) + cos(q1)*(cos(q4)*cos(q5)*sin(q3) + cos(q3)*sin(q5)) + cos(q2)*sin(q1)*(cos(q3)*cos(q4)*cos(q5) - sin(q3)*sin(q5)))*sin(q6)) + (-(KUKA_LBR_param_.dblLink7InertXY*cos(q1)) - KUKA_LBR_param_.dblLink7InertYY*sin(q1))*(cos(q6)*(cos(q4)*sin(q1)*sin(q2) - (cos(q2)*cos(q3)*sin(q1) + cos(q1)*sin(q3))*sin(q4)) + (cos(q5)*sin(q1)*sin(q2)*sin(q4) + cos(q1)*(cos(q4)*cos(q5)*sin(q3) + cos(q3)*sin(q5)) + cos(q2)*sin(q1)*(cos(q3)*cos(q4)*cos(q5) - sin(q3)*sin(q5)))*sin(q6)) + (KUKA_LBR_param_.dblLink7InertYY*cos(q1) - KUKA_LBR_param_.dblLink7InertXY*sin(q1))*(cos(q6)*(sin(q1)*sin(q3)*sin(q4) + cos(q1)*(cos(q4)*sin(q2) - cos(q2)*cos(q3)*sin(q4))) + (-(sin(q1)*(cos(q4)*cos(q5)*sin(q3) + cos(q3)*sin(q5))) + cos(q1)*(cos(q5)*sin(q2)*sin(q4) + cos(q2)*(cos(q3)*cos(q4)*cos(q5) - sin(q3)*sin(q5))))*sin(q6)) + KUKA_LBR_param_.dblLink7InertZZ*(cos(q5)*sin(q2)*sin(q4)*sin(q6) + cos(q4)*(cos(q6)*sin(q2) + cos(q2)*cos(q3)*cos(q5)*sin(q6)) - cos(q2)*(cos(q3)*cos(q6)*sin(q4) + sin(q3)*sin(q5)*sin(q6))) - KUKA_LBR_param_.dblLink7InertXZ*cos(q1)*(cos(q2)*(cos(q4)*cos(q6) + cos(q5)*sin(q4)*sin(q6)) + sin(q2)*(sin(q3)*sin(q5)*sin(q6) + cos(q3)*(cos(q6)*sin(q4) - cos(q4)*cos(q5)*sin(q6)))) - KUKA_LBR_param_.dblLink7InertYZ*sin(q1)*(cos(q2)*(cos(q4)*cos(q6) + cos(q5)*sin(q4)*sin(q6)) + sin(q2)*(sin(q3)*sin(q5)*sin(q6) + cos(q3)*(cos(q6)*sin(q4) - cos(q4)*cos(q5)*sin(q6)))) - (KUKA_LBR_param_.dblLink7InertXZ*cos(q1) + KUKA_LBR_param_.dblLink7InertYZ*sin(q1))*(cos(q2)*(cos(q4)*cos(q6) + cos(q5)*sin(q4)*sin(q6)) + sin(q2)*(sin(q3)*sin(q5)*sin(q6) + cos(q3)*(cos(q6)*sin(q4) - cos(q4)*cos(q5)*sin(q6)))) + KUKA_LBR_param_.dblLink7Mass*sin(q1)*(-(cos(q2)*(KUKA_LBR_param_.dblLink23Len + KUKA_LBR_param_.dblLink7CogY*cos(q7)*sin(q4)*sin(q5) + KUKA_LBR_param_.dblLink7CogX*sin(q4)*sin(q5)*sin(q7) + cos(q5)*sin(q4)*(-(KUKA_LBR_param_.dblLink7CogX*cos(q6)*cos(q7)) + KUKA_LBR_param_.dblLink7CogZ*sin(q6) + KUKA_LBR_param_.dblLink7CogY*cos(q6)*sin(q7)) + cos(q4)*(KUKA_LBR_param_.dblLink45Len + KUKA_LBR_param_.dblLink7CogZ*cos(q6) + KUKA_LBR_param_.dblLink7CogX*cos(q7)*sin(q6) - KUKA_LBR_param_.dblLink7CogY*sin(q6)*sin(q7)))) - sin(q2)*(-(sin(q3)*(cos(q5)*(KUKA_LBR_param_.dblLink7CogY*cos(q7) + KUKA_LBR_param_.dblLink7CogX*sin(q7)) + sin(q5)*(KUKA_LBR_param_.dblLink7CogX*cos(q6)*cos(q7) - KUKA_LBR_param_.dblLink7CogZ*sin(q6) - KUKA_LBR_param_.dblLink7CogY*cos(q6)*sin(q7)))) + cos(q3)*(sin(q4)*(KUKA_LBR_param_.dblLink45Len + KUKA_LBR_param_.dblLink7CogZ*cos(q6) + KUKA_LBR_param_.dblLink7CogX*cos(q7)*sin(q6) - KUKA_LBR_param_.dblLink7CogY*sin(q6)*sin(q7)) - cos(q4)*(sin(q5)*(KUKA_LBR_param_.dblLink7CogY*cos(q7) + KUKA_LBR_param_.dblLink7CogX*sin(q7)) + cos(q5)*(-(KUKA_LBR_param_.dblLink7CogX*cos(q6)*cos(q7)) + KUKA_LBR_param_.dblLink7CogZ*sin(q6) + KUKA_LBR_param_.dblLink7CogY*cos(q6)*sin(q7))))))*(sin(q1)*(cos(q3)*(cos(q6)*sin(q5)*(KUKA_LBR_param_.dblLink7CogY*cos(q7) + KUKA_LBR_param_.dblLink7CogX*sin(q7)) + cos(q5)*(-(KUKA_LBR_param_.dblLink7CogX*cos(q7)) + KUKA_LBR_param_.dblLink7CogY*sin(q7))) + sin(q3)*(sin(q4)*sin(q6)*(KUKA_LBR_param_.dblLink7CogY*cos(q7) + KUKA_LBR_param_.dblLink7CogX*sin(q7)) + cos(q4)*(cos(q5)*cos(q6)*(KUKA_LBR_param_.dblLink7CogY*cos(q7) + KUKA_LBR_param_.dblLink7CogX*sin(q7)) + sin(q5)*(KUKA_LBR_param_.dblLink7CogX*cos(q7) - KUKA_LBR_param_.dblLink7CogY*sin(q7))))) - cos(q1)*(sin(q2)*(cos(q7)*(KUKA_LBR_param_.dblLink7CogX*sin(q4)*sin(q5) - KUKA_LBR_param_.dblLink7CogY*cos(q4)*sin(q6)) - (KUKA_LBR_param_.dblLink7CogY*sin(q4)*sin(q5) + KUKA_LBR_param_.dblLink7CogX*cos(q4)*sin(q6))*sin(q7) + cos(q5)*cos(q6)*sin(q4)*(KUKA_LBR_param_.dblLink7CogY*cos(q7) + KUKA_LBR_param_.dblLink7CogX*sin(q7))) + cos(q2)*(sin(q3)*(-(cos(q6)*sin(q5)*(KUKA_LBR_param_.dblLink7CogY*cos(q7) + KUKA_LBR_param_.dblLink7CogX*sin(q7))) + cos(q5)*(KUKA_LBR_param_.dblLink7CogX*cos(q7) - KUKA_LBR_param_.dblLink7CogY*sin(q7))) + cos(q3)*(sin(q4)*sin(q6)*(KUKA_LBR_param_.dblLink7CogY*cos(q7) + KUKA_LBR_param_.dblLink7CogX*sin(q7)) + cos(q4)*(cos(q5)*cos(q6)*(KUKA_LBR_param_.dblLink7CogY*cos(q7) + KUKA_LBR_param_.dblLink7CogX*sin(q7)) + sin(q5)*(KUKA_LBR_param_.dblLink7CogX*cos(q7) - KUKA_LBR_param_.dblLink7CogY*sin(q7))))))) - KUKA_LBR_param_.dblLink7Mass*sin(q1)*(cos(q2)*(KUKA_LBR_param_.dblLink23Len + KUKA_LBR_param_.dblLink7CogY*cos(q7)*sin(q4)*sin(q5) + KUKA_LBR_param_.dblLink7CogX*sin(q4)*sin(q5)*sin(q7) + cos(q5)*sin(q4)*(-(KUKA_LBR_param_.dblLink7CogX*cos(q6)*cos(q7)) + KUKA_LBR_param_.dblLink7CogZ*sin(q6) + KUKA_LBR_param_.dblLink7CogY*cos(q6)*sin(q7)) + cos(q4)*(KUKA_LBR_param_.dblLink45Len + KUKA_LBR_param_.dblLink7CogZ*cos(q6) + KUKA_LBR_param_.dblLink7CogX*cos(q7)*sin(q6) - KUKA_LBR_param_.dblLink7CogY*sin(q6)*sin(q7))) + sin(q2)*(-(sin(q3)*(cos(q5)*(KUKA_LBR_param_.dblLink7CogY*cos(q7) + KUKA_LBR_param_.dblLink7CogX*sin(q7)) + sin(q5)*(KUKA_LBR_param_.dblLink7CogX*cos(q6)*cos(q7) - KUKA_LBR_param_.dblLink7CogZ*sin(q6) - KUKA_LBR_param_.dblLink7CogY*cos(q6)*sin(q7)))) + cos(q3)*(sin(q4)*(KUKA_LBR_param_.dblLink45Len + KUKA_LBR_param_.dblLink7CogZ*cos(q6) + KUKA_LBR_param_.dblLink7CogX*cos(q7)*sin(q6) - KUKA_LBR_param_.dblLink7CogY*sin(q6)*sin(q7)) - cos(q4)*(sin(q5)*(KUKA_LBR_param_.dblLink7CogY*cos(q7) + KUKA_LBR_param_.dblLink7CogX*sin(q7)) + cos(q5)*(-(KUKA_LBR_param_.dblLink7CogX*cos(q6)*cos(q7)) + KUKA_LBR_param_.dblLink7CogZ*sin(q6) + KUKA_LBR_param_.dblLink7CogY*cos(q6)*sin(q7))))))*(sin(q1)*(cos(q3)*(-(cos(q6)*sin(q5)*(KUKA_LBR_param_.dblLink7CogY*cos(q7) + KUKA_LBR_param_.dblLink7CogX*sin(q7))) + cos(q5)*(KUKA_LBR_param_.dblLink7CogX*cos(q7) - KUKA_LBR_param_.dblLink7CogY*sin(q7))) - sin(q3)*(sin(q4)*sin(q6)*(KUKA_LBR_param_.dblLink7CogY*cos(q7) + KUKA_LBR_param_.dblLink7CogX*sin(q7)) + cos(q4)*(cos(q5)*cos(q6)*(KUKA_LBR_param_.dblLink7CogY*cos(q7) + KUKA_LBR_param_.dblLink7CogX*sin(q7)) + sin(q5)*(KUKA_LBR_param_.dblLink7CogX*cos(q7) - KUKA_LBR_param_.dblLink7CogY*sin(q7))))) + cos(q1)*(sin(q2)*(cos(q7)*(KUKA_LBR_param_.dblLink7CogX*sin(q4)*sin(q5) - KUKA_LBR_param_.dblLink7CogY*cos(q4)*sin(q6)) - (KUKA_LBR_param_.dblLink7CogY*sin(q4)*sin(q5) + KUKA_LBR_param_.dblLink7CogX*cos(q4)*sin(q6))*sin(q7) + cos(q5)*cos(q6)*sin(q4)*(KUKA_LBR_param_.dblLink7CogY*cos(q7) + KUKA_LBR_param_.dblLink7CogX*sin(q7))) + cos(q2)*(sin(q3)*(-(cos(q6)*sin(q5)*(KUKA_LBR_param_.dblLink7CogY*cos(q7) + KUKA_LBR_param_.dblLink7CogX*sin(q7))) + cos(q5)*(KUKA_LBR_param_.dblLink7CogX*cos(q7) - KUKA_LBR_param_.dblLink7CogY*sin(q7))) + cos(q3)*(sin(q4)*sin(q6)*(KUKA_LBR_param_.dblLink7CogY*cos(q7) + KUKA_LBR_param_.dblLink7CogX*sin(q7)) + cos(q4)*(cos(q5)*cos(q6)*(KUKA_LBR_param_.dblLink7CogY*cos(q7) + KUKA_LBR_param_.dblLink7CogX*sin(q7)) + sin(q5)*(KUKA_LBR_param_.dblLink7CogX*cos(q7) - KUKA_LBR_param_.dblLink7CogY*sin(q7))))))) + KUKA_LBR_param_.dblLink7Mass*sin(q1)*(cos(q2)*(KUKA_LBR_param_.dblLink23Len + KUKA_LBR_param_.dblLink7CogY*cos(q7)*sin(q4)*sin(q5) + KUKA_LBR_param_.dblLink7CogX*sin(q4)*sin(q5)*sin(q7) + cos(q5)*sin(q4)*(-(KUKA_LBR_param_.dblLink7CogX*cos(q6)*cos(q7)) + KUKA_LBR_param_.dblLink7CogZ*sin(q6) + KUKA_LBR_param_.dblLink7CogY*cos(q6)*sin(q7)) + cos(q4)*(KUKA_LBR_param_.dblLink45Len + KUKA_LBR_param_.dblLink7CogZ*cos(q6) + KUKA_LBR_param_.dblLink7CogX*cos(q7)*sin(q6) - KUKA_LBR_param_.dblLink7CogY*sin(q6)*sin(q7))) + sin(q2)*(-(sin(q3)*(cos(q5)*(KUKA_LBR_param_.dblLink7CogY*cos(q7) + KUKA_LBR_param_.dblLink7CogX*sin(q7)) + sin(q5)*(KUKA_LBR_param_.dblLink7CogX*cos(q6)*cos(q7) - KUKA_LBR_param_.dblLink7CogZ*sin(q6) - KUKA_LBR_param_.dblLink7CogY*cos(q6)*sin(q7)))) + cos(q3)*(sin(q4)*(KUKA_LBR_param_.dblLink45Len + KUKA_LBR_param_.dblLink7CogZ*cos(q6) + KUKA_LBR_param_.dblLink7CogX*cos(q7)*sin(q6) - KUKA_LBR_param_.dblLink7CogY*sin(q6)*sin(q7)) - cos(q4)*(sin(q5)*(KUKA_LBR_param_.dblLink7CogY*cos(q7) + KUKA_LBR_param_.dblLink7CogX*sin(q7)) + cos(q5)*(-(KUKA_LBR_param_.dblLink7CogX*cos(q6)*cos(q7)) + KUKA_LBR_param_.dblLink7CogZ*sin(q6) + KUKA_LBR_param_.dblLink7CogY*cos(q6)*sin(q7))))))*(-(sin(q1)*(cos(q3)*(cos(q6)*sin(q5)*(KUKA_LBR_param_.dblLink7CogY*cos(q7) + KUKA_LBR_param_.dblLink7CogX*sin(q7)) + cos(q5)*(-(KUKA_LBR_param_.dblLink7CogX*cos(q7)) + KUKA_LBR_param_.dblLink7CogY*sin(q7))) + sin(q3)*(sin(q4)*sin(q6)*(KUKA_LBR_param_.dblLink7CogY*cos(q7) + KUKA_LBR_param_.dblLink7CogX*sin(q7)) + cos(q4)*(cos(q5)*cos(q6)*(KUKA_LBR_param_.dblLink7CogY*cos(q7) + KUKA_LBR_param_.dblLink7CogX*sin(q7)) + sin(q5)*(KUKA_LBR_param_.dblLink7CogX*cos(q7) - KUKA_LBR_param_.dblLink7CogY*sin(q7)))))) + cos(q1)*(sin(q2)*(cos(q7)*(KUKA_LBR_param_.dblLink7CogX*sin(q4)*sin(q5) - KUKA_LBR_param_.dblLink7CogY*cos(q4)*sin(q6)) - (KUKA_LBR_param_.dblLink7CogY*sin(q4)*sin(q5) + KUKA_LBR_param_.dblLink7CogX*cos(q4)*sin(q6))*sin(q7) + cos(q5)*cos(q6)*sin(q4)*(KUKA_LBR_param_.dblLink7CogY*cos(q7) + KUKA_LBR_param_.dblLink7CogX*sin(q7))) + cos(q2)*(sin(q3)*(-(cos(q6)*sin(q5)*(KUKA_LBR_param_.dblLink7CogY*cos(q7) + KUKA_LBR_param_.dblLink7CogX*sin(q7))) + cos(q5)*(KUKA_LBR_param_.dblLink7CogX*cos(q7) - KUKA_LBR_param_.dblLink7CogY*sin(q7))) + cos(q3)*(sin(q4)*sin(q6)*(KUKA_LBR_param_.dblLink7CogY*cos(q7) + KUKA_LBR_param_.dblLink7CogX*sin(q7)) + cos(q4)*(cos(q5)*cos(q6)*(KUKA_LBR_param_.dblLink7CogY*cos(q7) + KUKA_LBR_param_.dblLink7CogX*sin(q7)) + sin(q5)*(KUKA_LBR_param_.dblLink7CogX*cos(q7) - KUKA_LBR_param_.dblLink7CogY*sin(q7))))))) + KUKA_LBR_param_.dblLink7Mass*cos(q1)*(cos(q2)*(KUKA_LBR_param_.dblLink23Len + KUKA_LBR_param_.dblLink7CogY*cos(q7)*sin(q4)*sin(q5) + KUKA_LBR_param_.dblLink7CogX*sin(q4)*sin(q5)*sin(q7) + cos(q5)*sin(q4)*(-(KUKA_LBR_param_.dblLink7CogX*cos(q6)*cos(q7)) + KUKA_LBR_param_.dblLink7CogZ*sin(q6) + KUKA_LBR_param_.dblLink7CogY*cos(q6)*sin(q7)) + cos(q4)*(KUKA_LBR_param_.dblLink45Len + KUKA_LBR_param_.dblLink7CogZ*cos(q6) + KUKA_LBR_param_.dblLink7CogX*cos(q7)*sin(q6) - KUKA_LBR_param_.dblLink7CogY*sin(q6)*sin(q7))) + sin(q2)*(-(sin(q3)*(cos(q5)*(KUKA_LBR_param_.dblLink7CogY*cos(q7) + KUKA_LBR_param_.dblLink7CogX*sin(q7)) + sin(q5)*(KUKA_LBR_param_.dblLink7CogX*cos(q6)*cos(q7) - KUKA_LBR_param_.dblLink7CogZ*sin(q6) - KUKA_LBR_param_.dblLink7CogY*cos(q6)*sin(q7)))) + cos(q3)*(sin(q4)*(KUKA_LBR_param_.dblLink45Len + KUKA_LBR_param_.dblLink7CogZ*cos(q6) + KUKA_LBR_param_.dblLink7CogX*cos(q7)*sin(q6) - KUKA_LBR_param_.dblLink7CogY*sin(q6)*sin(q7)) - cos(q4)*(sin(q5)*(KUKA_LBR_param_.dblLink7CogY*cos(q7) + KUKA_LBR_param_.dblLink7CogX*sin(q7)) + cos(q5)*(-(KUKA_LBR_param_.dblLink7CogX*cos(q6)*cos(q7)) + KUKA_LBR_param_.dblLink7CogZ*sin(q6) + KUKA_LBR_param_.dblLink7CogY*cos(q6)*sin(q7))))))*(cos(q1)*(cos(q3)*(-(cos(q6)*sin(q5)*(KUKA_LBR_param_.dblLink7CogY*cos(q7) + KUKA_LBR_param_.dblLink7CogX*sin(q7))) + cos(q5)*(KUKA_LBR_param_.dblLink7CogX*cos(q7) - KUKA_LBR_param_.dblLink7CogY*sin(q7))) - sin(q3)*(sin(q4)*sin(q6)*(KUKA_LBR_param_.dblLink7CogY*cos(q7) + KUKA_LBR_param_.dblLink7CogX*sin(q7)) + cos(q4)*(cos(q5)*cos(q6)*(KUKA_LBR_param_.dblLink7CogY*cos(q7) + KUKA_LBR_param_.dblLink7CogX*sin(q7)) + sin(q5)*(KUKA_LBR_param_.dblLink7CogX*cos(q7) - KUKA_LBR_param_.dblLink7CogY*sin(q7))))) - sin(q1)*(sin(q2)*(cos(q7)*(KUKA_LBR_param_.dblLink7CogX*sin(q4)*sin(q5) - KUKA_LBR_param_.dblLink7CogY*cos(q4)*sin(q6)) - (KUKA_LBR_param_.dblLink7CogY*sin(q4)*sin(q5) + KUKA_LBR_param_.dblLink7CogX*cos(q4)*sin(q6))*sin(q7) + cos(q5)*cos(q6)*sin(q4)*(KUKA_LBR_param_.dblLink7CogY*cos(q7) + KUKA_LBR_param_.dblLink7CogX*sin(q7))) + cos(q2)*(sin(q3)*(-(cos(q6)*sin(q5)*(KUKA_LBR_param_.dblLink7CogY*cos(q7) + KUKA_LBR_param_.dblLink7CogX*sin(q7))) + cos(q5)*(KUKA_LBR_param_.dblLink7CogX*cos(q7) - KUKA_LBR_param_.dblLink7CogY*sin(q7))) + cos(q3)*(sin(q4)*sin(q6)*(KUKA_LBR_param_.dblLink7CogY*cos(q7) + KUKA_LBR_param_.dblLink7CogX*sin(q7)) + cos(q4)*(cos(q5)*cos(q6)*(KUKA_LBR_param_.dblLink7CogY*cos(q7) + KUKA_LBR_param_.dblLink7CogX*sin(q7)) + sin(q5)*(KUKA_LBR_param_.dblLink7CogX*cos(q7) - KUKA_LBR_param_.dblLink7CogY*sin(q7))))))) + KUKA_LBR_param_.dblLink7Mass*cos(q1)*(cos(q2)*(KUKA_LBR_param_.dblLink23Len + KUKA_LBR_param_.dblLink7CogY*cos(q7)*sin(q4)*sin(q5) + KUKA_LBR_param_.dblLink7CogX*sin(q4)*sin(q5)*sin(q7) + cos(q5)*sin(q4)*(-(KUKA_LBR_param_.dblLink7CogX*cos(q6)*cos(q7)) + KUKA_LBR_param_.dblLink7CogZ*sin(q6) + KUKA_LBR_param_.dblLink7CogY*cos(q6)*sin(q7)) + cos(q4)*(KUKA_LBR_param_.dblLink45Len + KUKA_LBR_param_.dblLink7CogZ*cos(q6) + KUKA_LBR_param_.dblLink7CogX*cos(q7)*sin(q6) - KUKA_LBR_param_.dblLink7CogY*sin(q6)*sin(q7))) + sin(q2)*(-(sin(q3)*(cos(q5)*(KUKA_LBR_param_.dblLink7CogY*cos(q7) + KUKA_LBR_param_.dblLink7CogX*sin(q7)) + sin(q5)*(KUKA_LBR_param_.dblLink7CogX*cos(q6)*cos(q7) - KUKA_LBR_param_.dblLink7CogZ*sin(q6) - KUKA_LBR_param_.dblLink7CogY*cos(q6)*sin(q7)))) + cos(q3)*(sin(q4)*(KUKA_LBR_param_.dblLink45Len + KUKA_LBR_param_.dblLink7CogZ*cos(q6) + KUKA_LBR_param_.dblLink7CogX*cos(q7)*sin(q6) - KUKA_LBR_param_.dblLink7CogY*sin(q6)*sin(q7)) - cos(q4)*(sin(q5)*(KUKA_LBR_param_.dblLink7CogY*cos(q7) + KUKA_LBR_param_.dblLink7CogX*sin(q7)) + cos(q5)*(-(KUKA_LBR_param_.dblLink7CogX*cos(q6)*cos(q7)) + KUKA_LBR_param_.dblLink7CogZ*sin(q6) + KUKA_LBR_param_.dblLink7CogY*cos(q6)*sin(q7))))))*(cos(q1)*(cos(q3)*(cos(q6)*sin(q5)*(KUKA_LBR_param_.dblLink7CogY*cos(q7) + KUKA_LBR_param_.dblLink7CogX*sin(q7)) + cos(q5)*(-(KUKA_LBR_param_.dblLink7CogX*cos(q7)) + KUKA_LBR_param_.dblLink7CogY*sin(q7))) + sin(q3)*(sin(q4)*sin(q6)*(KUKA_LBR_param_.dblLink7CogY*cos(q7) + KUKA_LBR_param_.dblLink7CogX*sin(q7)) + cos(q4)*(cos(q5)*cos(q6)*(KUKA_LBR_param_.dblLink7CogY*cos(q7) + KUKA_LBR_param_.dblLink7CogX*sin(q7)) + sin(q5)*(KUKA_LBR_param_.dblLink7CogX*cos(q7) - KUKA_LBR_param_.dblLink7CogY*sin(q7))))) + sin(q1)*(sin(q2)*(cos(q7)*(KUKA_LBR_param_.dblLink7CogX*sin(q4)*sin(q5) - KUKA_LBR_param_.dblLink7CogY*cos(q4)*sin(q6)) - (KUKA_LBR_param_.dblLink7CogY*sin(q4)*sin(q5) + KUKA_LBR_param_.dblLink7CogX*cos(q4)*sin(q6))*sin(q7) + cos(q5)*cos(q6)*sin(q4)*(KUKA_LBR_param_.dblLink7CogY*cos(q7) + KUKA_LBR_param_.dblLink7CogX*sin(q7))) + cos(q2)*(sin(q3)*(-(cos(q6)*sin(q5)*(KUKA_LBR_param_.dblLink7CogY*cos(q7) + KUKA_LBR_param_.dblLink7CogX*sin(q7))) + cos(q5)*(KUKA_LBR_param_.dblLink7CogX*cos(q7) - KUKA_LBR_param_.dblLink7CogY*sin(q7))) + cos(q3)*(sin(q4)*sin(q6)*(KUKA_LBR_param_.dblLink7CogY*cos(q7) + KUKA_LBR_param_.dblLink7CogX*sin(q7)) + cos(q4)*(cos(q5)*cos(q6)*(KUKA_LBR_param_.dblLink7CogY*cos(q7) + KUKA_LBR_param_.dblLink7CogX*sin(q7)) + sin(q5)*(KUKA_LBR_param_.dblLink7CogX*cos(q7) - KUKA_LBR_param_.dblLink7CogY*sin(q7))))))) - KUKA_LBR_param_.dblLink7Mass*cos(q1)*(cos(q2)*(KUKA_LBR_param_.dblLink23Len + KUKA_LBR_param_.dblLink7CogY*cos(q7)*sin(q4)*sin(q5) + KUKA_LBR_param_.dblLink7CogX*sin(q4)*sin(q5)*sin(q7) + cos(q5)*sin(q4)*(-(KUKA_LBR_param_.dblLink7CogX*cos(q6)*cos(q7)) + KUKA_LBR_param_.dblLink7CogZ*sin(q6) + KUKA_LBR_param_.dblLink7CogY*cos(q6)*sin(q7)) + cos(q4)*(KUKA_LBR_param_.dblLink45Len + KUKA_LBR_param_.dblLink7CogZ*cos(q6) + KUKA_LBR_param_.dblLink7CogX*cos(q7)*sin(q6) - KUKA_LBR_param_.dblLink7CogY*sin(q6)*sin(q7))) - sin(q2)*(sin(q3)*(cos(q5)*(KUKA_LBR_param_.dblLink7CogY*cos(q7) + KUKA_LBR_param_.dblLink7CogX*sin(q7)) + sin(q5)*(KUKA_LBR_param_.dblLink7CogX*cos(q6)*cos(q7) - KUKA_LBR_param_.dblLink7CogZ*sin(q6) - KUKA_LBR_param_.dblLink7CogY*cos(q6)*sin(q7))) + cos(q3)*(-(sin(q4)*(KUKA_LBR_param_.dblLink45Len + KUKA_LBR_param_.dblLink7CogZ*cos(q6) + KUKA_LBR_param_.dblLink7CogX*cos(q7)*sin(q6) - KUKA_LBR_param_.dblLink7CogY*sin(q6)*sin(q7))) + cos(q4)*(sin(q5)*(KUKA_LBR_param_.dblLink7CogY*cos(q7) + KUKA_LBR_param_.dblLink7CogX*sin(q7)) + cos(q5)*(-(KUKA_LBR_param_.dblLink7CogX*cos(q6)*cos(q7)) + KUKA_LBR_param_.dblLink7CogZ*sin(q6) + KUKA_LBR_param_.dblLink7CogY*cos(q6)*sin(q7))))))*(cos(q1)*(cos(q3)*(cos(q6)*sin(q5)*(KUKA_LBR_param_.dblLink7CogY*cos(q7) + KUKA_LBR_param_.dblLink7CogX*sin(q7)) + cos(q5)*(-(KUKA_LBR_param_.dblLink7CogX*cos(q7)) + KUKA_LBR_param_.dblLink7CogY*sin(q7))) + sin(q3)*(sin(q4)*sin(q6)*(KUKA_LBR_param_.dblLink7CogY*cos(q7) + KUKA_LBR_param_.dblLink7CogX*sin(q7)) + cos(q4)*(cos(q5)*cos(q6)*(KUKA_LBR_param_.dblLink7CogY*cos(q7) + KUKA_LBR_param_.dblLink7CogX*sin(q7)) + sin(q5)*(KUKA_LBR_param_.dblLink7CogX*cos(q7) - KUKA_LBR_param_.dblLink7CogY*sin(q7))))) + sin(q1)*(sin(q2)*(cos(q7)*(KUKA_LBR_param_.dblLink7CogX*sin(q4)*sin(q5) - KUKA_LBR_param_.dblLink7CogY*cos(q4)*sin(q6)) - (KUKA_LBR_param_.dblLink7CogY*sin(q4)*sin(q5) + KUKA_LBR_param_.dblLink7CogX*cos(q4)*sin(q6))*sin(q7) + cos(q5)*cos(q6)*sin(q4)*(KUKA_LBR_param_.dblLink7CogY*cos(q7) + KUKA_LBR_param_.dblLink7CogX*sin(q7))) + cos(q2)*(sin(q3)*(-(cos(q6)*sin(q5)*(KUKA_LBR_param_.dblLink7CogY*cos(q7) + KUKA_LBR_param_.dblLink7CogX*sin(q7))) + cos(q5)*(KUKA_LBR_param_.dblLink7CogX*cos(q7) - KUKA_LBR_param_.dblLink7CogY*sin(q7))) + cos(q3)*(sin(q4)*sin(q6)*(KUKA_LBR_param_.dblLink7CogY*cos(q7) + KUKA_LBR_param_.dblLink7CogX*sin(q7)) + cos(q4)*(cos(q5)*cos(q6)*(KUKA_LBR_param_.dblLink7CogY*cos(q7) + KUKA_LBR_param_.dblLink7CogX*sin(q7)) + sin(q5)*(KUKA_LBR_param_.dblLink7CogX*cos(q7) - KUKA_LBR_param_.dblLink7CogY*sin(q7))))))) + KUKA_LBR_param_.dblLink7Mass*sin(q1)*(cos(q2)*(KUKA_LBR_param_.dblLink23Len + KUKA_LBR_param_.dblLink7CogY*cos(q7)*sin(q4)*sin(q5) + KUKA_LBR_param_.dblLink7CogX*sin(q4)*sin(q5)*sin(q7) + cos(q5)*sin(q4)*(-(KUKA_LBR_param_.dblLink7CogX*cos(q6)*cos(q7)) + KUKA_LBR_param_.dblLink7CogZ*sin(q6) + KUKA_LBR_param_.dblLink7CogY*cos(q6)*sin(q7)) + cos(q4)*(KUKA_LBR_param_.dblLink45Len + KUKA_LBR_param_.dblLink7CogZ*cos(q6) + KUKA_LBR_param_.dblLink7CogX*cos(q7)*sin(q6) - KUKA_LBR_param_.dblLink7CogY*sin(q6)*sin(q7))) + sin(q2)*(-(sin(q3)*(cos(q5)*(KUKA_LBR_param_.dblLink7CogY*cos(q7) + KUKA_LBR_param_.dblLink7CogX*sin(q7)) + sin(q5)*(KUKA_LBR_param_.dblLink7CogX*cos(q6)*cos(q7) - KUKA_LBR_param_.dblLink7CogZ*sin(q6) - KUKA_LBR_param_.dblLink7CogY*cos(q6)*sin(q7)))) + cos(q3)*(sin(q4)*(KUKA_LBR_param_.dblLink45Len + KUKA_LBR_param_.dblLink7CogZ*cos(q6) + KUKA_LBR_param_.dblLink7CogX*cos(q7)*sin(q6) - KUKA_LBR_param_.dblLink7CogY*sin(q6)*sin(q7)) - cos(q4)*(sin(q5)*(KUKA_LBR_param_.dblLink7CogY*cos(q7) + KUKA_LBR_param_.dblLink7CogX*sin(q7)) + cos(q5)*(-(KUKA_LBR_param_.dblLink7CogX*cos(q6)*cos(q7)) + KUKA_LBR_param_.dblLink7CogZ*sin(q6) + KUKA_LBR_param_.dblLink7CogY*cos(q6)*sin(q7))))))*(sin(q1)*(cos(q3)*(-(cos(q6)*sin(q5)*(KUKA_LBR_param_.dblLink7CogY*cos(q7) + KUKA_LBR_param_.dblLink7CogX*sin(q7))) + cos(q5)*(KUKA_LBR_param_.dblLink7CogX*cos(q7) - KUKA_LBR_param_.dblLink7CogY*sin(q7))) - sin(q3)*(sin(q4)*sin(q6)*(KUKA_LBR_param_.dblLink7CogY*cos(q7) + KUKA_LBR_param_.dblLink7CogX*sin(q7)) + cos(q4)*(cos(q5)*cos(q6)*(KUKA_LBR_param_.dblLink7CogY*cos(q7) + KUKA_LBR_param_.dblLink7CogX*sin(q7)) + sin(q5)*(KUKA_LBR_param_.dblLink7CogX*cos(q7) - KUKA_LBR_param_.dblLink7CogY*sin(q7))))) + cos(q1)*(sin(q2)*(KUKA_LBR_param_.dblLink7CogX*cos(q7)*sin(q4)*sin(q5) - KUKA_LBR_param_.dblLink7CogY*sin(q4)*sin(q5)*sin(q7) + cos(q5)*cos(q6)*sin(q4)*(KUKA_LBR_param_.dblLink7CogY*cos(q7) + KUKA_LBR_param_.dblLink7CogX*sin(q7)) - cos(q4)*sin(q6)*(KUKA_LBR_param_.dblLink7CogY*cos(q7) + KUKA_LBR_param_.dblLink7CogX*sin(q7))) + cos(q2)*(sin(q3)*(-(cos(q6)*sin(q5)*(KUKA_LBR_param_.dblLink7CogY*cos(q7) + KUKA_LBR_param_.dblLink7CogX*sin(q7))) + cos(q5)*(KUKA_LBR_param_.dblLink7CogX*cos(q7) - KUKA_LBR_param_.dblLink7CogY*sin(q7))) + cos(q3)*(sin(q4)*sin(q6)*(KUKA_LBR_param_.dblLink7CogY*cos(q7) + KUKA_LBR_param_.dblLink7CogX*sin(q7)) + cos(q4)*(cos(q5)*cos(q6)*(KUKA_LBR_param_.dblLink7CogY*cos(q7) + KUKA_LBR_param_.dblLink7CogX*sin(q7)) + sin(q5)*(KUKA_LBR_param_.dblLink7CogX*cos(q7) - KUKA_LBR_param_.dblLink7CogY*sin(q7))))))) - KUKA_LBR_param_.dblLink7Mass*cos(q1)*(cos(q2)*(KUKA_LBR_param_.dblLink23Len + KUKA_LBR_param_.dblLink7CogY*cos(q7)*sin(q4)*sin(q5) + KUKA_LBR_param_.dblLink7CogX*sin(q4)*sin(q5)*sin(q7) + cos(q5)*sin(q4)*(-(KUKA_LBR_param_.dblLink7CogX*cos(q6)*cos(q7)) + KUKA_LBR_param_.dblLink7CogZ*sin(q6) + KUKA_LBR_param_.dblLink7CogY*cos(q6)*sin(q7)) + cos(q4)*(KUKA_LBR_param_.dblLink45Len + KUKA_LBR_param_.dblLink7CogZ*cos(q6) + KUKA_LBR_param_.dblLink7CogX*cos(q7)*sin(q6) - KUKA_LBR_param_.dblLink7CogY*sin(q6)*sin(q7))) + sin(q2)*(-(sin(q3)*(cos(q5)*(KUKA_LBR_param_.dblLink7CogY*cos(q7) + KUKA_LBR_param_.dblLink7CogX*sin(q7)) + sin(q5)*(KUKA_LBR_param_.dblLink7CogX*cos(q6)*cos(q7) - KUKA_LBR_param_.dblLink7CogZ*sin(q6) - KUKA_LBR_param_.dblLink7CogY*cos(q6)*sin(q7)))) + cos(q3)*(sin(q4)*(KUKA_LBR_param_.dblLink45Len + KUKA_LBR_param_.dblLink7CogZ*cos(q6) + KUKA_LBR_param_.dblLink7CogX*cos(q7)*sin(q6) - KUKA_LBR_param_.dblLink7CogY*sin(q6)*sin(q7)) - cos(q4)*(sin(q5)*(KUKA_LBR_param_.dblLink7CogY*cos(q7) + KUKA_LBR_param_.dblLink7CogX*sin(q7)) + cos(q5)*(-(KUKA_LBR_param_.dblLink7CogX*cos(q6)*cos(q7)) + KUKA_LBR_param_.dblLink7CogZ*sin(q6) + KUKA_LBR_param_.dblLink7CogY*cos(q6)*sin(q7))))))*(cos(q1)*(cos(q3)*(cos(q6)*sin(q5)*(KUKA_LBR_param_.dblLink7CogY*cos(q7) + KUKA_LBR_param_.dblLink7CogX*sin(q7)) + cos(q5)*(-(KUKA_LBR_param_.dblLink7CogX*cos(q7)) + KUKA_LBR_param_.dblLink7CogY*sin(q7))) + sin(q3)*(sin(q4)*sin(q6)*(KUKA_LBR_param_.dblLink7CogY*cos(q7) + KUKA_LBR_param_.dblLink7CogX*sin(q7)) + cos(q4)*(cos(q5)*cos(q6)*(KUKA_LBR_param_.dblLink7CogY*cos(q7) + KUKA_LBR_param_.dblLink7CogX*sin(q7)) + sin(q5)*(KUKA_LBR_param_.dblLink7CogX*cos(q7) - KUKA_LBR_param_.dblLink7CogY*sin(q7))))) + sin(q1)*(sin(q2)*(KUKA_LBR_param_.dblLink7CogX*cos(q7)*sin(q4)*sin(q5) - KUKA_LBR_param_.dblLink7CogY*sin(q4)*sin(q5)*sin(q7) + cos(q5)*cos(q6)*sin(q4)*(KUKA_LBR_param_.dblLink7CogY*cos(q7) + KUKA_LBR_param_.dblLink7CogX*sin(q7)) - cos(q4)*sin(q6)*(KUKA_LBR_param_.dblLink7CogY*cos(q7) + KUKA_LBR_param_.dblLink7CogX*sin(q7))) + cos(q2)*(sin(q3)*(-(cos(q6)*sin(q5)*(KUKA_LBR_param_.dblLink7CogY*cos(q7) + KUKA_LBR_param_.dblLink7CogX*sin(q7))) + cos(q5)*(KUKA_LBR_param_.dblLink7CogX*cos(q7) - KUKA_LBR_param_.dblLink7CogY*sin(q7))) + cos(q3)*(sin(q4)*sin(q6)*(KUKA_LBR_param_.dblLink7CogY*cos(q7) + KUKA_LBR_param_.dblLink7CogX*sin(q7)) + cos(q4)*(cos(q5)*cos(q6)*(KUKA_LBR_param_.dblLink7CogY*cos(q7) + KUKA_LBR_param_.dblLink7CogX*sin(q7)) + sin(q5)*(KUKA_LBR_param_.dblLink7CogX*cos(q7) - KUKA_LBR_param_.dblLink7CogY*sin(q7))))))) - KUKA_LBR_param_.dblLink7Mass*cos(q1)*(cos(q2)*(cos(q7)*(KUKA_LBR_param_.dblLink7CogX*sin(q4)*sin(q5) - KUKA_LBR_param_.dblLink7CogY*cos(q4)*sin(q6)) - (KUKA_LBR_param_.dblLink7CogY*sin(q4)*sin(q5) + KUKA_LBR_param_.dblLink7CogX*cos(q4)*sin(q6))*sin(q7) + cos(q5)*cos(q6)*sin(q4)*(KUKA_LBR_param_.dblLink7CogY*cos(q7) + KUKA_LBR_param_.dblLink7CogX*sin(q7))) - sin(q2)*(sin(q3)*(-(cos(q6)*sin(q5)*(KUKA_LBR_param_.dblLink7CogY*cos(q7) + KUKA_LBR_param_.dblLink7CogX*sin(q7))) + cos(q5)*(KUKA_LBR_param_.dblLink7CogX*cos(q7) - KUKA_LBR_param_.dblLink7CogY*sin(q7))) + cos(q3)*(sin(q4)*sin(q6)*(KUKA_LBR_param_.dblLink7CogY*cos(q7) + KUKA_LBR_param_.dblLink7CogX*sin(q7)) + cos(q4)*(cos(q5)*cos(q6)*(KUKA_LBR_param_.dblLink7CogY*cos(q7) + KUKA_LBR_param_.dblLink7CogX*sin(q7)) + sin(q5)*(KUKA_LBR_param_.dblLink7CogX*cos(q7) - KUKA_LBR_param_.dblLink7CogY*sin(q7))))))*(cos(q1)*(cos(q3)*(cos(q5)*(KUKA_LBR_param_.dblLink7CogY*cos(q7) + KUKA_LBR_param_.dblLink7CogX*sin(q7)) + sin(q5)*(KUKA_LBR_param_.dblLink7CogX*cos(q6)*cos(q7) - KUKA_LBR_param_.dblLink7CogZ*sin(q6) - KUKA_LBR_param_.dblLink7CogY*cos(q6)*sin(q7))) + sin(q3)*(sin(q4)*(KUKA_LBR_param_.dblLink45Len + KUKA_LBR_param_.dblLink7CogZ*cos(q6) + KUKA_LBR_param_.dblLink7CogX*cos(q7)*sin(q6) - KUKA_LBR_param_.dblLink7CogY*sin(q6)*sin(q7)) - cos(q4)*(sin(q5)*(KUKA_LBR_param_.dblLink7CogY*cos(q7) + KUKA_LBR_param_.dblLink7CogX*sin(q7)) + cos(q5)*(-(KUKA_LBR_param_.dblLink7CogX*cos(q6)*cos(q7)) + KUKA_LBR_param_.dblLink7CogZ*sin(q6) + KUKA_LBR_param_.dblLink7CogY*cos(q6)*sin(q7))))) + sin(q1)*(-(sin(q2)*(KUKA_LBR_param_.dblLink23Len + KUKA_LBR_param_.dblLink7CogY*cos(q7)*sin(q4)*sin(q5) + KUKA_LBR_param_.dblLink7CogX*sin(q4)*sin(q5)*sin(q7) + cos(q5)*sin(q4)*(-(KUKA_LBR_param_.dblLink7CogX*cos(q6)*cos(q7)) + KUKA_LBR_param_.dblLink7CogZ*sin(q6) + KUKA_LBR_param_.dblLink7CogY*cos(q6)*sin(q7)) + cos(q4)*(KUKA_LBR_param_.dblLink45Len + KUKA_LBR_param_.dblLink7CogZ*cos(q6) + KUKA_LBR_param_.dblLink7CogX*cos(q7)*sin(q6) - KUKA_LBR_param_.dblLink7CogY*sin(q6)*sin(q7)))) + cos(q2)*(-(sin(q3)*(cos(q5)*(KUKA_LBR_param_.dblLink7CogY*cos(q7) + KUKA_LBR_param_.dblLink7CogX*sin(q7)) + sin(q5)*(KUKA_LBR_param_.dblLink7CogX*cos(q6)*cos(q7) - KUKA_LBR_param_.dblLink7CogZ*sin(q6) - KUKA_LBR_param_.dblLink7CogY*cos(q6)*sin(q7)))) + cos(q3)*(sin(q4)*(KUKA_LBR_param_.dblLink45Len + KUKA_LBR_param_.dblLink7CogZ*cos(q6) + KUKA_LBR_param_.dblLink7CogX*cos(q7)*sin(q6) - KUKA_LBR_param_.dblLink7CogY*sin(q6)*sin(q7)) - cos(q4)*(sin(q5)*(KUKA_LBR_param_.dblLink7CogY*cos(q7) + KUKA_LBR_param_.dblLink7CogX*sin(q7)) + cos(q5)*(-(KUKA_LBR_param_.dblLink7CogX*cos(q6)*cos(q7)) + KUKA_LBR_param_.dblLink7CogZ*sin(q6) + KUKA_LBR_param_.dblLink7CogY*cos(q6)*sin(q7))))))) + KUKA_LBR_param_.dblLink7Mass*sin(q1)*(cos(q2)*(KUKA_LBR_param_.dblLink7CogX*cos(q7)*sin(q4)*sin(q5) - KUKA_LBR_param_.dblLink7CogY*sin(q4)*sin(q5)*sin(q7) + cos(q5)*cos(q6)*sin(q4)*(KUKA_LBR_param_.dblLink7CogY*cos(q7) + KUKA_LBR_param_.dblLink7CogX*sin(q7)) - cos(q4)*sin(q6)*(KUKA_LBR_param_.dblLink7CogY*cos(q7) + KUKA_LBR_param_.dblLink7CogX*sin(q7))) + sin(q2)*(sin(q3)*(cos(q6)*sin(q5)*(KUKA_LBR_param_.dblLink7CogY*cos(q7) + KUKA_LBR_param_.dblLink7CogX*sin(q7)) + cos(q5)*(-(KUKA_LBR_param_.dblLink7CogX*cos(q7)) + KUKA_LBR_param_.dblLink7CogY*sin(q7))) - cos(q3)*(sin(q4)*sin(q6)*(KUKA_LBR_param_.dblLink7CogY*cos(q7) + KUKA_LBR_param_.dblLink7CogX*sin(q7)) + cos(q4)*(cos(q5)*cos(q6)*(KUKA_LBR_param_.dblLink7CogY*cos(q7) + KUKA_LBR_param_.dblLink7CogX*sin(q7)) + sin(q5)*(KUKA_LBR_param_.dblLink7CogX*cos(q7) - KUKA_LBR_param_.dblLink7CogY*sin(q7))))))*(sin(q1)*(cos(q3)*(cos(q5)*(KUKA_LBR_param_.dblLink7CogY*cos(q7) + KUKA_LBR_param_.dblLink7CogX*sin(q7)) + sin(q5)*(KUKA_LBR_param_.dblLink7CogX*cos(q6)*cos(q7) - KUKA_LBR_param_.dblLink7CogZ*sin(q6) - KUKA_LBR_param_.dblLink7CogY*cos(q6)*sin(q7))) + sin(q3)*(sin(q4)*(KUKA_LBR_param_.dblLink45Len + KUKA_LBR_param_.dblLink7CogZ*cos(q6) + KUKA_LBR_param_.dblLink7CogX*cos(q7)*sin(q6) - KUKA_LBR_param_.dblLink7CogY*sin(q6)*sin(q7)) - cos(q4)*(sin(q5)*(KUKA_LBR_param_.dblLink7CogY*cos(q7) + KUKA_LBR_param_.dblLink7CogX*sin(q7)) + cos(q5)*(-(KUKA_LBR_param_.dblLink7CogX*cos(q6)*cos(q7)) + KUKA_LBR_param_.dblLink7CogZ*sin(q6) + KUKA_LBR_param_.dblLink7CogY*cos(q6)*sin(q7))))) + cos(q1)*(sin(q2)*(KUKA_LBR_param_.dblLink23Len + KUKA_LBR_param_.dblLink7CogY*cos(q7)*sin(q4)*sin(q5) + KUKA_LBR_param_.dblLink7CogX*sin(q4)*sin(q5)*sin(q7) + cos(q5)*sin(q4)*(-(KUKA_LBR_param_.dblLink7CogX*cos(q6)*cos(q7)) + KUKA_LBR_param_.dblLink7CogZ*sin(q6) + KUKA_LBR_param_.dblLink7CogY*cos(q6)*sin(q7)) + cos(q4)*(KUKA_LBR_param_.dblLink45Len + KUKA_LBR_param_.dblLink7CogZ*cos(q6) + KUKA_LBR_param_.dblLink7CogX*cos(q7)*sin(q6) - KUKA_LBR_param_.dblLink7CogY*sin(q6)*sin(q7))) + cos(q2)*(sin(q3)*(cos(q5)*(KUKA_LBR_param_.dblLink7CogY*cos(q7) + KUKA_LBR_param_.dblLink7CogX*sin(q7)) + sin(q5)*(KUKA_LBR_param_.dblLink7CogX*cos(q6)*cos(q7) - KUKA_LBR_param_.dblLink7CogZ*sin(q6) - KUKA_LBR_param_.dblLink7CogY*cos(q6)*sin(q7))) + cos(q3)*(-(sin(q4)*(KUKA_LBR_param_.dblLink45Len + KUKA_LBR_param_.dblLink7CogZ*cos(q6) + KUKA_LBR_param_.dblLink7CogX*cos(q7)*sin(q6) - KUKA_LBR_param_.dblLink7CogY*sin(q6)*sin(q7))) + cos(q4)*(sin(q5)*(KUKA_LBR_param_.dblLink7CogY*cos(q7) + KUKA_LBR_param_.dblLink7CogX*sin(q7)) + cos(q5)*(-(KUKA_LBR_param_.dblLink7CogX*cos(q6)*cos(q7)) + KUKA_LBR_param_.dblLink7CogZ*sin(q6) + KUKA_LBR_param_.dblLink7CogY*cos(q6)*sin(q7))))))) - KUKA_LBR_param_.dblLink7Mass*sin(q1)*(cos(q2)*(cos(q7)*(KUKA_LBR_param_.dblLink7CogX*sin(q4)*sin(q5) - KUKA_LBR_param_.dblLink7CogY*cos(q4)*sin(q6)) - (KUKA_LBR_param_.dblLink7CogY*sin(q4)*sin(q5) + KUKA_LBR_param_.dblLink7CogX*cos(q4)*sin(q6))*sin(q7) + cos(q5)*cos(q6)*sin(q4)*(KUKA_LBR_param_.dblLink7CogY*cos(q7) + KUKA_LBR_param_.dblLink7CogX*sin(q7))) - sin(q2)*(sin(q3)*(-(cos(q6)*sin(q5)*(KUKA_LBR_param_.dblLink7CogY*cos(q7) + KUKA_LBR_param_.dblLink7CogX*sin(q7))) + cos(q5)*(KUKA_LBR_param_.dblLink7CogX*cos(q7) - KUKA_LBR_param_.dblLink7CogY*sin(q7))) + cos(q3)*(sin(q4)*sin(q6)*(KUKA_LBR_param_.dblLink7CogY*cos(q7) + KUKA_LBR_param_.dblLink7CogX*sin(q7)) + cos(q4)*(cos(q5)*cos(q6)*(KUKA_LBR_param_.dblLink7CogY*cos(q7) + KUKA_LBR_param_.dblLink7CogX*sin(q7)) + sin(q5)*(KUKA_LBR_param_.dblLink7CogX*cos(q7) - KUKA_LBR_param_.dblLink7CogY*sin(q7))))))*(sin(q1)*(cos(q3)*(cos(q5)*(KUKA_LBR_param_.dblLink7CogY*cos(q7) + KUKA_LBR_param_.dblLink7CogX*sin(q7)) + sin(q5)*(KUKA_LBR_param_.dblLink7CogX*cos(q6)*cos(q7) - KUKA_LBR_param_.dblLink7CogZ*sin(q6) - KUKA_LBR_param_.dblLink7CogY*cos(q6)*sin(q7))) + sin(q3)*(sin(q4)*(KUKA_LBR_param_.dblLink45Len + KUKA_LBR_param_.dblLink7CogZ*cos(q6) + KUKA_LBR_param_.dblLink7CogX*cos(q7)*sin(q6) - KUKA_LBR_param_.dblLink7CogY*sin(q6)*sin(q7)) - cos(q4)*(sin(q5)*(KUKA_LBR_param_.dblLink7CogY*cos(q7) + KUKA_LBR_param_.dblLink7CogX*sin(q7)) + cos(q5)*(-(KUKA_LBR_param_.dblLink7CogX*cos(q6)*cos(q7)) + KUKA_LBR_param_.dblLink7CogZ*sin(q6) + KUKA_LBR_param_.dblLink7CogY*cos(q6)*sin(q7))))) + cos(q1)*(sin(q2)*(KUKA_LBR_param_.dblLink23Len + KUKA_LBR_param_.dblLink7CogY*cos(q7)*sin(q4)*sin(q5) + KUKA_LBR_param_.dblLink7CogX*sin(q4)*sin(q5)*sin(q7) + cos(q5)*sin(q4)*(-(KUKA_LBR_param_.dblLink7CogX*cos(q6)*cos(q7)) + KUKA_LBR_param_.dblLink7CogZ*sin(q6) + KUKA_LBR_param_.dblLink7CogY*cos(q6)*sin(q7)) + cos(q4)*(KUKA_LBR_param_.dblLink45Len + KUKA_LBR_param_.dblLink7CogZ*cos(q6) + KUKA_LBR_param_.dblLink7CogX*cos(q7)*sin(q6) - KUKA_LBR_param_.dblLink7CogY*sin(q6)*sin(q7))) + cos(q2)*(sin(q3)*(cos(q5)*(KUKA_LBR_param_.dblLink7CogY*cos(q7) + KUKA_LBR_param_.dblLink7CogX*sin(q7)) + sin(q5)*(KUKA_LBR_param_.dblLink7CogX*cos(q6)*cos(q7) - KUKA_LBR_param_.dblLink7CogZ*sin(q6) - KUKA_LBR_param_.dblLink7CogY*cos(q6)*sin(q7))) + cos(q3)*(-(sin(q4)*(KUKA_LBR_param_.dblLink45Len + KUKA_LBR_param_.dblLink7CogZ*cos(q6) + KUKA_LBR_param_.dblLink7CogX*cos(q7)*sin(q6) - KUKA_LBR_param_.dblLink7CogY*sin(q6)*sin(q7))) + cos(q4)*(sin(q5)*(KUKA_LBR_param_.dblLink7CogY*cos(q7) + KUKA_LBR_param_.dblLink7CogX*sin(q7)) + cos(q5)*(-(KUKA_LBR_param_.dblLink7CogX*cos(q6)*cos(q7)) + KUKA_LBR_param_.dblLink7CogZ*sin(q6) + KUKA_LBR_param_.dblLink7CogY*cos(q6)*sin(q7))))))) - KUKA_LBR_param_.dblLink7Mass*cos(q1)*(cos(q2)*(KUKA_LBR_param_.dblLink7CogX*cos(q7)*sin(q4)*sin(q5) - KUKA_LBR_param_.dblLink7CogY*sin(q4)*sin(q5)*sin(q7) + cos(q5)*cos(q6)*sin(q4)*(KUKA_LBR_param_.dblLink7CogY*cos(q7) + KUKA_LBR_param_.dblLink7CogX*sin(q7)) - cos(q4)*sin(q6)*(KUKA_LBR_param_.dblLink7CogY*cos(q7) + KUKA_LBR_param_.dblLink7CogX*sin(q7))) + sin(q2)*(sin(q3)*(cos(q6)*sin(q5)*(KUKA_LBR_param_.dblLink7CogY*cos(q7) + KUKA_LBR_param_.dblLink7CogX*sin(q7)) + cos(q5)*(-(KUKA_LBR_param_.dblLink7CogX*cos(q7)) + KUKA_LBR_param_.dblLink7CogY*sin(q7))) - cos(q3)*(sin(q4)*sin(q6)*(KUKA_LBR_param_.dblLink7CogY*cos(q7) + KUKA_LBR_param_.dblLink7CogX*sin(q7)) + cos(q4)*(cos(q5)*cos(q6)*(KUKA_LBR_param_.dblLink7CogY*cos(q7) + KUKA_LBR_param_.dblLink7CogX*sin(q7)) + sin(q5)*(KUKA_LBR_param_.dblLink7CogX*cos(q7) - KUKA_LBR_param_.dblLink7CogY*sin(q7))))))*(cos(q1)*(-(cos(q3)*(cos(q5)*(KUKA_LBR_param_.dblLink7CogY*cos(q7) + KUKA_LBR_param_.dblLink7CogX*sin(q7)) + sin(q5)*(KUKA_LBR_param_.dblLink7CogX*cos(q6)*cos(q7) - KUKA_LBR_param_.dblLink7CogZ*sin(q6) - KUKA_LBR_param_.dblLink7CogY*cos(q6)*sin(q7)))) + sin(q3)*(-(sin(q4)*(KUKA_LBR_param_.dblLink45Len + KUKA_LBR_param_.dblLink7CogZ*cos(q6) + KUKA_LBR_param_.dblLink7CogX*cos(q7)*sin(q6) - KUKA_LBR_param_.dblLink7CogY*sin(q6)*sin(q7))) + cos(q4)*(sin(q5)*(KUKA_LBR_param_.dblLink7CogY*cos(q7) + KUKA_LBR_param_.dblLink7CogX*sin(q7)) + cos(q5)*(-(KUKA_LBR_param_.dblLink7CogX*cos(q6)*cos(q7)) + KUKA_LBR_param_.dblLink7CogZ*sin(q6) + KUKA_LBR_param_.dblLink7CogY*cos(q6)*sin(q7))))) + sin(q1)*(sin(q2)*(KUKA_LBR_param_.dblLink23Len + KUKA_LBR_param_.dblLink7CogY*cos(q7)*sin(q4)*sin(q5) + KUKA_LBR_param_.dblLink7CogX*sin(q4)*sin(q5)*sin(q7) + cos(q5)*sin(q4)*(-(KUKA_LBR_param_.dblLink7CogX*cos(q6)*cos(q7)) + KUKA_LBR_param_.dblLink7CogZ*sin(q6) + KUKA_LBR_param_.dblLink7CogY*cos(q6)*sin(q7)) + cos(q4)*(KUKA_LBR_param_.dblLink45Len + KUKA_LBR_param_.dblLink7CogZ*cos(q6) + KUKA_LBR_param_.dblLink7CogX*cos(q7)*sin(q6) - KUKA_LBR_param_.dblLink7CogY*sin(q6)*sin(q7))) + cos(q2)*(sin(q3)*(cos(q5)*(KUKA_LBR_param_.dblLink7CogY*cos(q7) + KUKA_LBR_param_.dblLink7CogX*sin(q7)) + sin(q5)*(KUKA_LBR_param_.dblLink7CogX*cos(q6)*cos(q7) - KUKA_LBR_param_.dblLink7CogZ*sin(q6) - KUKA_LBR_param_.dblLink7CogY*cos(q6)*sin(q7))) + cos(q3)*(-(sin(q4)*(KUKA_LBR_param_.dblLink45Len + KUKA_LBR_param_.dblLink7CogZ*cos(q6) + KUKA_LBR_param_.dblLink7CogX*cos(q7)*sin(q6) - KUKA_LBR_param_.dblLink7CogY*sin(q6)*sin(q7))) + cos(q4)*(sin(q5)*(KUKA_LBR_param_.dblLink7CogY*cos(q7) + KUKA_LBR_param_.dblLink7CogX*sin(q7)) + cos(q5)*(-(KUKA_LBR_param_.dblLink7CogX*cos(q6)*cos(q7)) + KUKA_LBR_param_.dblLink7CogZ*sin(q6) + KUKA_LBR_param_.dblLink7CogY*cos(q6)*sin(q7)))))))))/2.0;
dblCoriolisCentrifugalFullRow2Col2 = (q14*((KUKA_LBR_param_.dblLink7InertYZ*cos(q1) - KUKA_LBR_param_.dblLink7InertXZ*sin(q1))*(-(sin(q2)*(cos(q4)*cos(q6) + cos(q5)*sin(q4)*sin(q6))) + cos(q2)*(sin(q3)*sin(q5)*sin(q6) + cos(q3)*(cos(q6)*sin(q4) - cos(q4)*cos(q5)*sin(q6)))) + cos(q1)*(KUKA_LBR_param_.dblLink7InertXY*cos(q1) - KUKA_LBR_param_.dblLink7InertXX*sin(q1))*(cos(q2)*(cos(q4)*cos(q6) + cos(q5)*sin(q4)*sin(q6)) + sin(q2)*(sin(q3)*sin(q5)*sin(q6) + cos(q3)*(cos(q6)*sin(q4) - cos(q4)*cos(q5)*sin(q6)))) + sin(q1)*(KUKA_LBR_param_.dblLink7InertYY*cos(q1) - KUKA_LBR_param_.dblLink7InertXY*sin(q1))*(cos(q2)*(cos(q4)*cos(q6) + cos(q5)*sin(q4)*sin(q6)) + sin(q2)*(sin(q3)*sin(q5)*sin(q6) + cos(q3)*(cos(q6)*sin(q4) - cos(q4)*cos(q5)*sin(q6)))) + sin(q1)*(KUKA_LBR_param_.dblLink7InertXZ*(-(sin(q2)*(cos(q4)*cos(q6) + cos(q5)*sin(q4)*sin(q6))) + cos(q2)*(sin(q3)*sin(q5)*sin(q6) + cos(q3)*(cos(q6)*sin(q4) - cos(q4)*cos(q5)*sin(q6)))) + KUKA_LBR_param_.dblLink7InertXX*cos(q1)*(cos(q2)*(cos(q4)*cos(q6) + cos(q5)*sin(q4)*sin(q6)) + sin(q2)*(sin(q3)*sin(q5)*sin(q6) + cos(q3)*(cos(q6)*sin(q4) - cos(q4)*cos(q5)*sin(q6)))) + KUKA_LBR_param_.dblLink7InertXY*sin(q1)*(cos(q2)*(cos(q4)*cos(q6) + cos(q5)*sin(q4)*sin(q6)) + sin(q2)*(sin(q3)*sin(q5)*sin(q6) + cos(q3)*(cos(q6)*sin(q4) - cos(q4)*cos(q5)*sin(q6))))) - cos(q1)*(KUKA_LBR_param_.dblLink7InertYZ*(-(sin(q2)*(cos(q4)*cos(q6) + cos(q5)*sin(q4)*sin(q6))) + cos(q2)*(sin(q3)*sin(q5)*sin(q6) + cos(q3)*(cos(q6)*sin(q4) - cos(q4)*cos(q5)*sin(q6)))) + KUKA_LBR_param_.dblLink7InertXY*cos(q1)*(cos(q2)*(cos(q4)*cos(q6) + cos(q5)*sin(q4)*sin(q6)) + sin(q2)*(sin(q3)*sin(q5)*sin(q6) + cos(q3)*(cos(q6)*sin(q4) - cos(q4)*cos(q5)*sin(q6)))) + KUKA_LBR_param_.dblLink7InertYY*sin(q1)*(cos(q2)*(cos(q4)*cos(q6) + cos(q5)*sin(q4)*sin(q6)) + sin(q2)*(sin(q3)*sin(q5)*sin(q6) + cos(q3)*(cos(q6)*sin(q4) - cos(q4)*cos(q5)*sin(q6))))) + 2*KUKA_LBR_param_.dblLink7Mass*(sin(q2)*(KUKA_LBR_param_.dblLink7CogX*cos(q7)*sin(q4)*sin(q5) - KUKA_LBR_param_.dblLink7CogY*sin(q4)*sin(q5)*sin(q7) + cos(q5)*cos(q6)*sin(q4)*(KUKA_LBR_param_.dblLink7CogY*cos(q7) + KUKA_LBR_param_.dblLink7CogX*sin(q7)) - cos(q4)*sin(q6)*(KUKA_LBR_param_.dblLink7CogY*cos(q7) + KUKA_LBR_param_.dblLink7CogX*sin(q7))) - cos(q2)*(sin(q3)*(cos(q6)*sin(q5)*(KUKA_LBR_param_.dblLink7CogY*cos(q7) + KUKA_LBR_param_.dblLink7CogX*sin(q7)) + cos(q5)*(-(KUKA_LBR_param_.dblLink7CogX*cos(q7)) + KUKA_LBR_param_.dblLink7CogY*sin(q7))) - cos(q3)*(sin(q4)*sin(q6)*(KUKA_LBR_param_.dblLink7CogY*cos(q7) + KUKA_LBR_param_.dblLink7CogX*sin(q7)) + cos(q4)*(cos(q5)*cos(q6)*(KUKA_LBR_param_.dblLink7CogY*cos(q7) + KUKA_LBR_param_.dblLink7CogX*sin(q7)) + sin(q5)*(KUKA_LBR_param_.dblLink7CogX*cos(q7) - KUKA_LBR_param_.dblLink7CogY*sin(q7))))))*(sin(q2)*(KUKA_LBR_param_.dblLink23Len + KUKA_LBR_param_.dblLink7CogY*cos(q7)*sin(q4)*sin(q5) + KUKA_LBR_param_.dblLink7CogX*sin(q4)*sin(q5)*sin(q7) + cos(q5)*sin(q4)*(-(KUKA_LBR_param_.dblLink7CogX*cos(q6)*cos(q7)) + KUKA_LBR_param_.dblLink7CogZ*sin(q6) + KUKA_LBR_param_.dblLink7CogY*cos(q6)*sin(q7)) + cos(q4)*(KUKA_LBR_param_.dblLink45Len + KUKA_LBR_param_.dblLink7CogZ*cos(q6) + KUKA_LBR_param_.dblLink7CogX*cos(q7)*sin(q6) - KUKA_LBR_param_.dblLink7CogY*sin(q6)*sin(q7))) - cos(q2)*(-(sin(q3)*(cos(q5)*(KUKA_LBR_param_.dblLink7CogY*cos(q7) + KUKA_LBR_param_.dblLink7CogX*sin(q7)) + sin(q5)*(KUKA_LBR_param_.dblLink7CogX*cos(q6)*cos(q7) - KUKA_LBR_param_.dblLink7CogZ*sin(q6) - KUKA_LBR_param_.dblLink7CogY*cos(q6)*sin(q7)))) + cos(q3)*(sin(q4)*(KUKA_LBR_param_.dblLink45Len + KUKA_LBR_param_.dblLink7CogZ*cos(q6) + KUKA_LBR_param_.dblLink7CogX*cos(q7)*sin(q6) - KUKA_LBR_param_.dblLink7CogY*sin(q6)*sin(q7)) - cos(q4)*(sin(q5)*(KUKA_LBR_param_.dblLink7CogY*cos(q7) + KUKA_LBR_param_.dblLink7CogX*sin(q7)) + cos(q5)*(-(KUKA_LBR_param_.dblLink7CogX*cos(q6)*cos(q7)) + KUKA_LBR_param_.dblLink7CogZ*sin(q6) + KUKA_LBR_param_.dblLink7CogY*cos(q6)*sin(q7)))))) + 2*KUKA_LBR_param_.dblLink7Mass*power(cos(q1),2)*(cos(q2)*(KUKA_LBR_param_.dblLink7CogX*cos(q7)*sin(q4)*sin(q5) - KUKA_LBR_param_.dblLink7CogY*sin(q4)*sin(q5)*sin(q7) + cos(q5)*cos(q6)*sin(q4)*(KUKA_LBR_param_.dblLink7CogY*cos(q7) + KUKA_LBR_param_.dblLink7CogX*sin(q7)) - cos(q4)*sin(q6)*(KUKA_LBR_param_.dblLink7CogY*cos(q7) + KUKA_LBR_param_.dblLink7CogX*sin(q7))) + sin(q2)*(sin(q3)*(cos(q6)*sin(q5)*(KUKA_LBR_param_.dblLink7CogY*cos(q7) + KUKA_LBR_param_.dblLink7CogX*sin(q7)) + cos(q5)*(-(KUKA_LBR_param_.dblLink7CogX*cos(q7)) + KUKA_LBR_param_.dblLink7CogY*sin(q7))) - cos(q3)*(sin(q4)*sin(q6)*(KUKA_LBR_param_.dblLink7CogY*cos(q7) + KUKA_LBR_param_.dblLink7CogX*sin(q7)) + cos(q4)*(cos(q5)*cos(q6)*(KUKA_LBR_param_.dblLink7CogY*cos(q7) + KUKA_LBR_param_.dblLink7CogX*sin(q7)) + sin(q5)*(KUKA_LBR_param_.dblLink7CogX*cos(q7) - KUKA_LBR_param_.dblLink7CogY*sin(q7))))))*(cos(q2)*(KUKA_LBR_param_.dblLink23Len + KUKA_LBR_param_.dblLink7CogY*cos(q7)*sin(q4)*sin(q5) + KUKA_LBR_param_.dblLink7CogX*sin(q4)*sin(q5)*sin(q7) + cos(q5)*sin(q4)*(-(KUKA_LBR_param_.dblLink7CogX*cos(q6)*cos(q7)) + KUKA_LBR_param_.dblLink7CogZ*sin(q6) + KUKA_LBR_param_.dblLink7CogY*cos(q6)*sin(q7)) + cos(q4)*(KUKA_LBR_param_.dblLink45Len + KUKA_LBR_param_.dblLink7CogZ*cos(q6) + KUKA_LBR_param_.dblLink7CogX*cos(q7)*sin(q6) - KUKA_LBR_param_.dblLink7CogY*sin(q6)*sin(q7))) + sin(q2)*(-(sin(q3)*(cos(q5)*(KUKA_LBR_param_.dblLink7CogY*cos(q7) + KUKA_LBR_param_.dblLink7CogX*sin(q7)) + sin(q5)*(KUKA_LBR_param_.dblLink7CogX*cos(q6)*cos(q7) - KUKA_LBR_param_.dblLink7CogZ*sin(q6) - KUKA_LBR_param_.dblLink7CogY*cos(q6)*sin(q7)))) + cos(q3)*(sin(q4)*(KUKA_LBR_param_.dblLink45Len + KUKA_LBR_param_.dblLink7CogZ*cos(q6) + KUKA_LBR_param_.dblLink7CogX*cos(q7)*sin(q6) - KUKA_LBR_param_.dblLink7CogY*sin(q6)*sin(q7)) - cos(q4)*(sin(q5)*(KUKA_LBR_param_.dblLink7CogY*cos(q7) + KUKA_LBR_param_.dblLink7CogX*sin(q7)) + cos(q5)*(-(KUKA_LBR_param_.dblLink7CogX*cos(q6)*cos(q7)) + KUKA_LBR_param_.dblLink7CogZ*sin(q6) + KUKA_LBR_param_.dblLink7CogY*cos(q6)*sin(q7)))))) + 2*KUKA_LBR_param_.dblLink7Mass*power(sin(q1),2)*(cos(q2)*(KUKA_LBR_param_.dblLink7CogX*cos(q7)*sin(q4)*sin(q5) - KUKA_LBR_param_.dblLink7CogY*sin(q4)*sin(q5)*sin(q7) + cos(q5)*cos(q6)*sin(q4)*(KUKA_LBR_param_.dblLink7CogY*cos(q7) + KUKA_LBR_param_.dblLink7CogX*sin(q7)) - cos(q4)*sin(q6)*(KUKA_LBR_param_.dblLink7CogY*cos(q7) + KUKA_LBR_param_.dblLink7CogX*sin(q7))) + sin(q2)*(sin(q3)*(cos(q6)*sin(q5)*(KUKA_LBR_param_.dblLink7CogY*cos(q7) + KUKA_LBR_param_.dblLink7CogX*sin(q7)) + cos(q5)*(-(KUKA_LBR_param_.dblLink7CogX*cos(q7)) + KUKA_LBR_param_.dblLink7CogY*sin(q7))) - cos(q3)*(sin(q4)*sin(q6)*(KUKA_LBR_param_.dblLink7CogY*cos(q7) + KUKA_LBR_param_.dblLink7CogX*sin(q7)) + cos(q4)*(cos(q5)*cos(q6)*(KUKA_LBR_param_.dblLink7CogY*cos(q7) + KUKA_LBR_param_.dblLink7CogX*sin(q7)) + sin(q5)*(KUKA_LBR_param_.dblLink7CogX*cos(q7) - KUKA_LBR_param_.dblLink7CogY*sin(q7))))))*(cos(q2)*(KUKA_LBR_param_.dblLink23Len + KUKA_LBR_param_.dblLink7CogY*cos(q7)*sin(q4)*sin(q5) + KUKA_LBR_param_.dblLink7CogX*sin(q4)*sin(q5)*sin(q7) + cos(q5)*sin(q4)*(-(KUKA_LBR_param_.dblLink7CogX*cos(q6)*cos(q7)) + KUKA_LBR_param_.dblLink7CogZ*sin(q6) + KUKA_LBR_param_.dblLink7CogY*cos(q6)*sin(q7)) + cos(q4)*(KUKA_LBR_param_.dblLink45Len + KUKA_LBR_param_.dblLink7CogZ*cos(q6) + KUKA_LBR_param_.dblLink7CogX*cos(q7)*sin(q6) - KUKA_LBR_param_.dblLink7CogY*sin(q6)*sin(q7))) + sin(q2)*(-(sin(q3)*(cos(q5)*(KUKA_LBR_param_.dblLink7CogY*cos(q7) + KUKA_LBR_param_.dblLink7CogX*sin(q7)) + sin(q5)*(KUKA_LBR_param_.dblLink7CogX*cos(q6)*cos(q7) - KUKA_LBR_param_.dblLink7CogZ*sin(q6) - KUKA_LBR_param_.dblLink7CogY*cos(q6)*sin(q7)))) + cos(q3)*(sin(q4)*(KUKA_LBR_param_.dblLink45Len + KUKA_LBR_param_.dblLink7CogZ*cos(q6) + KUKA_LBR_param_.dblLink7CogX*cos(q7)*sin(q6) - KUKA_LBR_param_.dblLink7CogY*sin(q6)*sin(q7)) - cos(q4)*(sin(q5)*(KUKA_LBR_param_.dblLink7CogY*cos(q7) + KUKA_LBR_param_.dblLink7CogX*sin(q7)) + cos(q5)*(-(KUKA_LBR_param_.dblLink7CogX*cos(q6)*cos(q7)) + KUKA_LBR_param_.dblLink7CogZ*sin(q6) + KUKA_LBR_param_.dblLink7CogY*cos(q6)*sin(q7))))))))/2.0;
dblCoriolisCentrifugalFullRow2Col3 = (q14*((KUKA_LBR_param_.dblLink7InertYZ*cos(q1) - KUKA_LBR_param_.dblLink7InertXZ*sin(q1))*sin(q2)*(-(cos(q6)*sin(q3)*sin(q4)) + (cos(q4)*cos(q5)*sin(q3) + cos(q3)*sin(q5))*sin(q6)) + (KUKA_LBR_param_.dblLink7InertXY*cos(q1) - KUKA_LBR_param_.dblLink7InertXX*sin(q1))*(cos(q3)*(cos(q6)*sin(q1)*sin(q4) - (cos(q4)*cos(q5)*sin(q1) + cos(q1)*cos(q2)*sin(q5))*sin(q6)) + sin(q3)*(sin(q1)*sin(q5)*sin(q6) + cos(q1)*cos(q2)*(cos(q6)*sin(q4) - cos(q4)*cos(q5)*sin(q6)))) + (KUKA_LBR_param_.dblLink7InertYY*cos(q1) - KUKA_LBR_param_.dblLink7InertXY*sin(q1))*(cos(q2)*sin(q1)*(cos(q6)*sin(q3)*sin(q4) - (cos(q4)*cos(q5)*sin(q3) + cos(q3)*sin(q5))*sin(q6)) - cos(q1)*(sin(q3)*sin(q5)*sin(q6) + cos(q3)*(cos(q6)*sin(q4) - cos(q4)*cos(q5)*sin(q6)))) - cos(q1)*cos(q2)*(KUKA_LBR_param_.dblLink7InertXX*(cos(q6)*(sin(q1)*sin(q3)*sin(q4) + cos(q1)*(cos(q4)*sin(q2) - cos(q2)*cos(q3)*sin(q4))) - (cos(q5)*(cos(q4)*sin(q1)*sin(q3) - cos(q1)*(cos(q2)*cos(q3)*cos(q4) + sin(q2)*sin(q4))) + (cos(q3)*sin(q1) + cos(q1)*cos(q2)*sin(q3))*sin(q5))*sin(q6)) + KUKA_LBR_param_.dblLink7InertXY*(cos(q6)*(cos(q4)*sin(q1)*sin(q2) - (cos(q2)*cos(q3)*sin(q1) + cos(q1)*sin(q3))*sin(q4)) + (cos(q5)*sin(q1)*sin(q2)*sin(q4) + cos(q1)*(cos(q4)*cos(q5)*sin(q3) + cos(q3)*sin(q5)) + cos(q2)*sin(q1)*(cos(q3)*cos(q4)*cos(q5) - sin(q3)*sin(q5)))*sin(q6)) + KUKA_LBR_param_.dblLink7InertXZ*(cos(q2)*(cos(q4)*cos(q6) + cos(q5)*sin(q4)*sin(q6)) + sin(q2)*(sin(q3)*sin(q5)*sin(q6) + cos(q3)*(cos(q6)*sin(q4) - cos(q4)*cos(q5)*sin(q6))))) - cos(q2)*sin(q1)*(KUKA_LBR_param_.dblLink7InertXY*(cos(q6)*(sin(q1)*sin(q3)*sin(q4) + cos(q1)*(cos(q4)*sin(q2) - cos(q2)*cos(q3)*sin(q4))) - (cos(q5)*(cos(q4)*sin(q1)*sin(q3) - cos(q1)*(cos(q2)*cos(q3)*cos(q4) + sin(q2)*sin(q4))) + (cos(q3)*sin(q1) + cos(q1)*cos(q2)*sin(q3))*sin(q5))*sin(q6)) + KUKA_LBR_param_.dblLink7InertYY*(cos(q6)*(cos(q4)*sin(q1)*sin(q2) - (cos(q2)*cos(q3)*sin(q1) + cos(q1)*sin(q3))*sin(q4)) + (cos(q5)*sin(q1)*sin(q2)*sin(q4) + cos(q1)*(cos(q4)*cos(q5)*sin(q3) + cos(q3)*sin(q5)) + cos(q2)*sin(q1)*(cos(q3)*cos(q4)*cos(q5) - sin(q3)*sin(q5)))*sin(q6)) + KUKA_LBR_param_.dblLink7InertYZ*(cos(q2)*(cos(q4)*cos(q6) + cos(q5)*sin(q4)*sin(q6)) + sin(q2)*(sin(q3)*sin(q5)*sin(q6) + cos(q3)*(cos(q6)*sin(q4) - cos(q4)*cos(q5)*sin(q6))))) + sin(q2)*(KUKA_LBR_param_.dblLink7InertXZ*(cos(q6)*(sin(q1)*sin(q3)*sin(q4) + cos(q1)*(cos(q4)*sin(q2) - cos(q2)*cos(q3)*sin(q4))) - (cos(q5)*(cos(q4)*sin(q1)*sin(q3) - cos(q1)*(cos(q2)*cos(q3)*cos(q4) + sin(q2)*sin(q4))) + (cos(q3)*sin(q1) + cos(q1)*cos(q2)*sin(q3))*sin(q5))*sin(q6)) + KUKA_LBR_param_.dblLink7InertYZ*(cos(q6)*(cos(q4)*sin(q1)*sin(q2) - (cos(q2)*cos(q3)*sin(q1) + cos(q1)*sin(q3))*sin(q4)) + (cos(q5)*sin(q1)*sin(q2)*sin(q4) + cos(q1)*(cos(q4)*cos(q5)*sin(q3) + cos(q3)*sin(q5)) + cos(q2)*sin(q1)*(cos(q3)*cos(q4)*cos(q5) - sin(q3)*sin(q5)))*sin(q6)) + KUKA_LBR_param_.dblLink7InertZZ*(cos(q2)*(cos(q4)*cos(q6) + cos(q5)*sin(q4)*sin(q6)) + sin(q2)*(sin(q3)*sin(q5)*sin(q6) + cos(q3)*(cos(q6)*sin(q4) - cos(q4)*cos(q5)*sin(q6))))) - cos(q1)*sin(q2)*(KUKA_LBR_param_.dblLink7InertXZ*(-(sin(q2)*(cos(q4)*cos(q6) + cos(q5)*sin(q4)*sin(q6))) + cos(q2)*(sin(q3)*sin(q5)*sin(q6) + cos(q3)*(cos(q6)*sin(q4) - cos(q4)*cos(q5)*sin(q6)))) + KUKA_LBR_param_.dblLink7InertXX*cos(q1)*(cos(q2)*(cos(q4)*cos(q6) + cos(q5)*sin(q4)*sin(q6)) + sin(q2)*(sin(q3)*sin(q5)*sin(q6) + cos(q3)*(cos(q6)*sin(q4) - cos(q4)*cos(q5)*sin(q6)))) + KUKA_LBR_param_.dblLink7InertXY*sin(q1)*(cos(q2)*(cos(q4)*cos(q6) + cos(q5)*sin(q4)*sin(q6)) + sin(q2)*(sin(q3)*sin(q5)*sin(q6) + cos(q3)*(cos(q6)*sin(q4) - cos(q4)*cos(q5)*sin(q6))))) - sin(q1)*sin(q2)*(KUKA_LBR_param_.dblLink7InertYZ*(-(sin(q2)*(cos(q4)*cos(q6) + cos(q5)*sin(q4)*sin(q6))) + cos(q2)*(sin(q3)*sin(q5)*sin(q6) + cos(q3)*(cos(q6)*sin(q4) - cos(q4)*cos(q5)*sin(q6)))) + KUKA_LBR_param_.dblLink7InertXY*cos(q1)*(cos(q2)*(cos(q4)*cos(q6) + cos(q5)*sin(q4)*sin(q6)) + sin(q2)*(sin(q3)*sin(q5)*sin(q6) + cos(q3)*(cos(q6)*sin(q4) - cos(q4)*cos(q5)*sin(q6)))) + KUKA_LBR_param_.dblLink7InertYY*sin(q1)*(cos(q2)*(cos(q4)*cos(q6) + cos(q5)*sin(q4)*sin(q6)) + sin(q2)*(sin(q3)*sin(q5)*sin(q6) + cos(q3)*(cos(q6)*sin(q4) - cos(q4)*cos(q5)*sin(q6))))) - cos(q2)*(KUKA_LBR_param_.dblLink7InertZZ*(-(sin(q2)*(cos(q4)*cos(q6) + cos(q5)*sin(q4)*sin(q6))) + cos(q2)*(sin(q3)*sin(q5)*sin(q6) + cos(q3)*(cos(q6)*sin(q4) - cos(q4)*cos(q5)*sin(q6)))) + KUKA_LBR_param_.dblLink7InertXZ*cos(q1)*(cos(q2)*(cos(q4)*cos(q6) + cos(q5)*sin(q4)*sin(q6)) + sin(q2)*(sin(q3)*sin(q5)*sin(q6) + cos(q3)*(cos(q6)*sin(q4) - cos(q4)*cos(q5)*sin(q6)))) + KUKA_LBR_param_.dblLink7InertYZ*sin(q1)*(cos(q2)*(cos(q4)*cos(q6) + cos(q5)*sin(q4)*sin(q6)) + sin(q2)*(sin(q3)*sin(q5)*sin(q6) + cos(q3)*(cos(q6)*sin(q4) - cos(q4)*cos(q5)*sin(q6))))) - KUKA_LBR_param_.dblLink7Mass*cos(q2)*(-(KUKA_LBR_param_.dblLink7CogY*cos(q6)*cos(q7)*sin(q2)*sin(q3)*sin(q5)) - KUKA_LBR_param_.dblLink7CogX*cos(q2)*cos(q7)*sin(q4)*sin(q5) + KUKA_LBR_param_.dblLink7CogY*cos(q2)*cos(q4)*cos(q7)*sin(q6) - KUKA_LBR_param_.dblLink7CogX*cos(q6)*sin(q2)*sin(q3)*sin(q5)*sin(q7) + KUKA_LBR_param_.dblLink7CogY*cos(q2)*sin(q4)*sin(q5)*sin(q7) + KUKA_LBR_param_.dblLink7CogX*cos(q2)*cos(q4)*sin(q6)*sin(q7) + cos(q5)*(cos(q7)*(KUKA_LBR_param_.dblLink7CogX*sin(q2)*sin(q3) - KUKA_LBR_param_.dblLink7CogY*cos(q2)*cos(q6)*sin(q4)) - (KUKA_LBR_param_.dblLink7CogY*sin(q2)*sin(q3) + KUKA_LBR_param_.dblLink7CogX*cos(q2)*cos(q6)*sin(q4))*sin(q7)) + cos(q3)*sin(q2)*(sin(q4)*sin(q6)*(KUKA_LBR_param_.dblLink7CogY*cos(q7) + KUKA_LBR_param_.dblLink7CogX*sin(q7)) + cos(q4)*(cos(q5)*cos(q6)*(KUKA_LBR_param_.dblLink7CogY*cos(q7) + KUKA_LBR_param_.dblLink7CogX*sin(q7)) + sin(q5)*(KUKA_LBR_param_.dblLink7CogX*cos(q7) - KUKA_LBR_param_.dblLink7CogY*sin(q7)))))*(cos(q3)*(cos(q5)*(KUKA_LBR_param_.dblLink7CogY*cos(q7) + KUKA_LBR_param_.dblLink7CogX*sin(q7)) + sin(q5)*(KUKA_LBR_param_.dblLink7CogX*cos(q6)*cos(q7) - KUKA_LBR_param_.dblLink7CogZ*sin(q6) - KUKA_LBR_param_.dblLink7CogY*cos(q6)*sin(q7))) + sin(q3)*(sin(q4)*(KUKA_LBR_param_.dblLink45Len + KUKA_LBR_param_.dblLink7CogZ*cos(q6) + KUKA_LBR_param_.dblLink7CogX*cos(q7)*sin(q6) - KUKA_LBR_param_.dblLink7CogY*sin(q6)*sin(q7)) - cos(q4)*(sin(q5)*(KUKA_LBR_param_.dblLink7CogY*cos(q7) + KUKA_LBR_param_.dblLink7CogX*sin(q7)) + cos(q5)*(-(KUKA_LBR_param_.dblLink7CogX*cos(q6)*cos(q7)) + KUKA_LBR_param_.dblLink7CogZ*sin(q6) + KUKA_LBR_param_.dblLink7CogY*cos(q6)*sin(q7))))) - KUKA_LBR_param_.dblLink7Mass*cos(q2)*(-(KUKA_LBR_param_.dblLink7CogY*cos(q6)*cos(q7)*sin(q2)*sin(q3)*sin(q5)) - KUKA_LBR_param_.dblLink7CogX*cos(q2)*cos(q7)*sin(q4)*sin(q5) + KUKA_LBR_param_.dblLink7CogY*cos(q2)*cos(q4)*cos(q7)*sin(q6) - KUKA_LBR_param_.dblLink7CogX*cos(q6)*sin(q2)*sin(q3)*sin(q5)*sin(q7) + KUKA_LBR_param_.dblLink7CogY*cos(q2)*sin(q4)*sin(q5)*sin(q7) + KUKA_LBR_param_.dblLink7CogX*cos(q2)*cos(q4)*sin(q6)*sin(q7) + cos(q5)*(cos(q7)*(KUKA_LBR_param_.dblLink7CogX*sin(q2)*sin(q3) - KUKA_LBR_param_.dblLink7CogY*cos(q2)*cos(q6)*sin(q4)) - (KUKA_LBR_param_.dblLink7CogY*sin(q2)*sin(q3) + KUKA_LBR_param_.dblLink7CogX*cos(q2)*cos(q6)*sin(q4))*sin(q7)) + cos(q3)*sin(q2)*(sin(q4)*sin(q6)*(KUKA_LBR_param_.dblLink7CogY*cos(q7) + KUKA_LBR_param_.dblLink7CogX*sin(q7)) + cos(q4)*(cos(q5)*cos(q6)*(KUKA_LBR_param_.dblLink7CogY*cos(q7) + KUKA_LBR_param_.dblLink7CogX*sin(q7)) + sin(q5)*(KUKA_LBR_param_.dblLink7CogX*cos(q7) - KUKA_LBR_param_.dblLink7CogY*sin(q7)))))*(-(cos(q3)*(cos(q5)*(KUKA_LBR_param_.dblLink7CogY*cos(q7) + KUKA_LBR_param_.dblLink7CogX*sin(q7)) + sin(q5)*(KUKA_LBR_param_.dblLink7CogX*cos(q6)*cos(q7) - KUKA_LBR_param_.dblLink7CogZ*sin(q6) - KUKA_LBR_param_.dblLink7CogY*cos(q6)*sin(q7)))) + sin(q3)*(-(sin(q4)*(KUKA_LBR_param_.dblLink45Len + KUKA_LBR_param_.dblLink7CogZ*cos(q6) + KUKA_LBR_param_.dblLink7CogX*cos(q7)*sin(q6) - KUKA_LBR_param_.dblLink7CogY*sin(q6)*sin(q7))) + cos(q4)*(sin(q5)*(KUKA_LBR_param_.dblLink7CogY*cos(q7) + KUKA_LBR_param_.dblLink7CogX*sin(q7)) + cos(q5)*(-(KUKA_LBR_param_.dblLink7CogX*cos(q6)*cos(q7)) + KUKA_LBR_param_.dblLink7CogZ*sin(q6) + KUKA_LBR_param_.dblLink7CogY*cos(q6)*sin(q7))))) + KUKA_LBR_param_.dblLink7Mass*sin(q2)*(-(cos(q3)*(cos(q5)*(KUKA_LBR_param_.dblLink7CogY*cos(q7) + KUKA_LBR_param_.dblLink7CogX*sin(q7)) + sin(q5)*(KUKA_LBR_param_.dblLink7CogX*cos(q6)*cos(q7) - KUKA_LBR_param_.dblLink7CogZ*sin(q6) - KUKA_LBR_param_.dblLink7CogY*cos(q6)*sin(q7)))) + sin(q3)*(-(sin(q4)*(KUKA_LBR_param_.dblLink45Len + KUKA_LBR_param_.dblLink7CogZ*cos(q6) + KUKA_LBR_param_.dblLink7CogX*cos(q7)*sin(q6) - KUKA_LBR_param_.dblLink7CogY*sin(q6)*sin(q7))) + cos(q4)*(sin(q5)*(KUKA_LBR_param_.dblLink7CogY*cos(q7) + KUKA_LBR_param_.dblLink7CogX*sin(q7)) + cos(q5)*(-(KUKA_LBR_param_.dblLink7CogX*cos(q6)*cos(q7)) + KUKA_LBR_param_.dblLink7CogZ*sin(q6) + KUKA_LBR_param_.dblLink7CogY*cos(q6)*sin(q7)))))*(-(sin(q2)*(KUKA_LBR_param_.dblLink7CogX*cos(q7)*sin(q4)*sin(q5) - KUKA_LBR_param_.dblLink7CogY*sin(q4)*sin(q5)*sin(q7) + cos(q5)*cos(q6)*sin(q4)*(KUKA_LBR_param_.dblLink7CogY*cos(q7) + KUKA_LBR_param_.dblLink7CogX*sin(q7)) - cos(q4)*sin(q6)*(KUKA_LBR_param_.dblLink7CogY*cos(q7) + KUKA_LBR_param_.dblLink7CogX*sin(q7)))) + cos(q2)*(sin(q3)*(cos(q6)*sin(q5)*(KUKA_LBR_param_.dblLink7CogY*cos(q7) + KUKA_LBR_param_.dblLink7CogX*sin(q7)) + cos(q5)*(-(KUKA_LBR_param_.dblLink7CogX*cos(q7)) + KUKA_LBR_param_.dblLink7CogY*sin(q7))) - cos(q3)*(sin(q4)*sin(q6)*(KUKA_LBR_param_.dblLink7CogY*cos(q7) + KUKA_LBR_param_.dblLink7CogX*sin(q7)) + cos(q4)*(cos(q5)*cos(q6)*(KUKA_LBR_param_.dblLink7CogY*cos(q7) + KUKA_LBR_param_.dblLink7CogX*sin(q7)) + sin(q5)*(KUKA_LBR_param_.dblLink7CogX*cos(q7) - KUKA_LBR_param_.dblLink7CogY*sin(q7)))))) - KUKA_LBR_param_.dblLink7Mass*sin(q2)*(cos(q3)*(cos(q5)*(KUKA_LBR_param_.dblLink7CogY*cos(q7) + KUKA_LBR_param_.dblLink7CogX*sin(q7)) + sin(q5)*(KUKA_LBR_param_.dblLink7CogX*cos(q6)*cos(q7) - KUKA_LBR_param_.dblLink7CogZ*sin(q6) - KUKA_LBR_param_.dblLink7CogY*cos(q6)*sin(q7))) + sin(q3)*(sin(q4)*(KUKA_LBR_param_.dblLink45Len + KUKA_LBR_param_.dblLink7CogZ*cos(q6) + KUKA_LBR_param_.dblLink7CogX*cos(q7)*sin(q6) - KUKA_LBR_param_.dblLink7CogY*sin(q6)*sin(q7)) - cos(q4)*(sin(q5)*(KUKA_LBR_param_.dblLink7CogY*cos(q7) + KUKA_LBR_param_.dblLink7CogX*sin(q7)) + cos(q5)*(-(KUKA_LBR_param_.dblLink7CogX*cos(q6)*cos(q7)) + KUKA_LBR_param_.dblLink7CogZ*sin(q6) + KUKA_LBR_param_.dblLink7CogY*cos(q6)*sin(q7)))))*(sin(q2)*(cos(q7)*(KUKA_LBR_param_.dblLink7CogX*sin(q4)*sin(q5) - KUKA_LBR_param_.dblLink7CogY*cos(q4)*sin(q6)) - (KUKA_LBR_param_.dblLink7CogY*sin(q4)*sin(q5) + KUKA_LBR_param_.dblLink7CogX*cos(q4)*sin(q6))*sin(q7) + cos(q5)*cos(q6)*sin(q4)*(KUKA_LBR_param_.dblLink7CogY*cos(q7) + KUKA_LBR_param_.dblLink7CogX*sin(q7))) + cos(q2)*(sin(q3)*(-(cos(q6)*sin(q5)*(KUKA_LBR_param_.dblLink7CogY*cos(q7) + KUKA_LBR_param_.dblLink7CogX*sin(q7))) + cos(q5)*(KUKA_LBR_param_.dblLink7CogX*cos(q7) - KUKA_LBR_param_.dblLink7CogY*sin(q7))) + cos(q3)*(sin(q4)*sin(q6)*(KUKA_LBR_param_.dblLink7CogY*cos(q7) + KUKA_LBR_param_.dblLink7CogX*sin(q7)) + cos(q4)*(cos(q5)*cos(q6)*(KUKA_LBR_param_.dblLink7CogY*cos(q7) + KUKA_LBR_param_.dblLink7CogX*sin(q7)) + sin(q5)*(KUKA_LBR_param_.dblLink7CogX*cos(q7) - KUKA_LBR_param_.dblLink7CogY*sin(q7)))))) - KUKA_LBR_param_.dblLink7Mass*sin(q2)*(cos(q3)*(-(cos(q6)*sin(q5)*(KUKA_LBR_param_.dblLink7CogY*cos(q7) + KUKA_LBR_param_.dblLink7CogX*sin(q7))) + cos(q5)*(KUKA_LBR_param_.dblLink7CogX*cos(q7) - KUKA_LBR_param_.dblLink7CogY*sin(q7))) - sin(q3)*(sin(q4)*sin(q6)*(KUKA_LBR_param_.dblLink7CogY*cos(q7) + KUKA_LBR_param_.dblLink7CogX*sin(q7)) + cos(q4)*(cos(q5)*cos(q6)*(KUKA_LBR_param_.dblLink7CogY*cos(q7) + KUKA_LBR_param_.dblLink7CogX*sin(q7)) + sin(q5)*(KUKA_LBR_param_.dblLink7CogX*cos(q7) - KUKA_LBR_param_.dblLink7CogY*sin(q7)))))*(-(sin(q2)*(KUKA_LBR_param_.dblLink23Len + KUKA_LBR_param_.dblLink7CogY*cos(q7)*sin(q4)*sin(q5) + KUKA_LBR_param_.dblLink7CogX*sin(q4)*sin(q5)*sin(q7) + cos(q5)*sin(q4)*(-(KUKA_LBR_param_.dblLink7CogX*cos(q6)*cos(q7)) + KUKA_LBR_param_.dblLink7CogZ*sin(q6) + KUKA_LBR_param_.dblLink7CogY*cos(q6)*sin(q7)) + cos(q4)*(KUKA_LBR_param_.dblLink45Len + KUKA_LBR_param_.dblLink7CogZ*cos(q6) + KUKA_LBR_param_.dblLink7CogX*cos(q7)*sin(q6) - KUKA_LBR_param_.dblLink7CogY*sin(q6)*sin(q7)))) + cos(q2)*(-(sin(q3)*(cos(q5)*(KUKA_LBR_param_.dblLink7CogY*cos(q7) + KUKA_LBR_param_.dblLink7CogX*sin(q7)) + sin(q5)*(KUKA_LBR_param_.dblLink7CogX*cos(q6)*cos(q7) - KUKA_LBR_param_.dblLink7CogZ*sin(q6) - KUKA_LBR_param_.dblLink7CogY*cos(q6)*sin(q7)))) + cos(q3)*(sin(q4)*(KUKA_LBR_param_.dblLink45Len + KUKA_LBR_param_.dblLink7CogZ*cos(q6) + KUKA_LBR_param_.dblLink7CogX*cos(q7)*sin(q6) - KUKA_LBR_param_.dblLink7CogY*sin(q6)*sin(q7)) - cos(q4)*(sin(q5)*(KUKA_LBR_param_.dblLink7CogY*cos(q7) + KUKA_LBR_param_.dblLink7CogX*sin(q7)) + cos(q5)*(-(KUKA_LBR_param_.dblLink7CogX*cos(q6)*cos(q7)) + KUKA_LBR_param_.dblLink7CogZ*sin(q6) + KUKA_LBR_param_.dblLink7CogY*cos(q6)*sin(q7)))))) + KUKA_LBR_param_.dblLink7Mass*sin(q2)*(cos(q3)*(cos(q6)*sin(q5)*(KUKA_LBR_param_.dblLink7CogY*cos(q7) + KUKA_LBR_param_.dblLink7CogX*sin(q7)) + cos(q5)*(-(KUKA_LBR_param_.dblLink7CogX*cos(q7)) + KUKA_LBR_param_.dblLink7CogY*sin(q7))) + sin(q3)*(sin(q4)*sin(q6)*(KUKA_LBR_param_.dblLink7CogY*cos(q7) + KUKA_LBR_param_.dblLink7CogX*sin(q7)) + cos(q4)*(cos(q5)*cos(q6)*(KUKA_LBR_param_.dblLink7CogY*cos(q7) + KUKA_LBR_param_.dblLink7CogX*sin(q7)) + sin(q5)*(KUKA_LBR_param_.dblLink7CogX*cos(q7) - KUKA_LBR_param_.dblLink7CogY*sin(q7)))))*(-(sin(q2)*(KUKA_LBR_param_.dblLink23Len + KUKA_LBR_param_.dblLink7CogY*cos(q7)*sin(q4)*sin(q5) + KUKA_LBR_param_.dblLink7CogX*sin(q4)*sin(q5)*sin(q7) + cos(q5)*sin(q4)*(-(KUKA_LBR_param_.dblLink7CogX*cos(q6)*cos(q7)) + KUKA_LBR_param_.dblLink7CogZ*sin(q6) + KUKA_LBR_param_.dblLink7CogY*cos(q6)*sin(q7)) + cos(q4)*(KUKA_LBR_param_.dblLink45Len + KUKA_LBR_param_.dblLink7CogZ*cos(q6) + KUKA_LBR_param_.dblLink7CogX*cos(q7)*sin(q6) - KUKA_LBR_param_.dblLink7CogY*sin(q6)*sin(q7)))) + cos(q2)*(-(sin(q3)*(cos(q5)*(KUKA_LBR_param_.dblLink7CogY*cos(q7) + KUKA_LBR_param_.dblLink7CogX*sin(q7)) + sin(q5)*(KUKA_LBR_param_.dblLink7CogX*cos(q6)*cos(q7) - KUKA_LBR_param_.dblLink7CogZ*sin(q6) - KUKA_LBR_param_.dblLink7CogY*cos(q6)*sin(q7)))) + cos(q3)*(sin(q4)*(KUKA_LBR_param_.dblLink45Len + KUKA_LBR_param_.dblLink7CogZ*cos(q6) + KUKA_LBR_param_.dblLink7CogX*cos(q7)*sin(q6) - KUKA_LBR_param_.dblLink7CogY*sin(q6)*sin(q7)) - cos(q4)*(sin(q5)*(KUKA_LBR_param_.dblLink7CogY*cos(q7) + KUKA_LBR_param_.dblLink7CogX*sin(q7)) + cos(q5)*(-(KUKA_LBR_param_.dblLink7CogX*cos(q6)*cos(q7)) + KUKA_LBR_param_.dblLink7CogZ*sin(q6) + KUKA_LBR_param_.dblLink7CogY*cos(q6)*sin(q7)))))) + 2*KUKA_LBR_param_.dblLink7Mass*cos(q1)*(sin(q1)*(sin(q3)*(cos(q6)*sin(q5)*(KUKA_LBR_param_.dblLink7CogY*cos(q7) + KUKA_LBR_param_.dblLink7CogX*sin(q7)) + cos(q5)*(-(KUKA_LBR_param_.dblLink7CogX*cos(q7)) + KUKA_LBR_param_.dblLink7CogY*sin(q7))) - cos(q3)*(sin(q4)*sin(q6)*(KUKA_LBR_param_.dblLink7CogY*cos(q7) + KUKA_LBR_param_.dblLink7CogX*sin(q7)) + cos(q4)*(cos(q5)*cos(q6)*(KUKA_LBR_param_.dblLink7CogY*cos(q7) + KUKA_LBR_param_.dblLink7CogX*sin(q7)) + sin(q5)*(KUKA_LBR_param_.dblLink7CogX*cos(q7) - KUKA_LBR_param_.dblLink7CogY*sin(q7))))) + cos(q1)*cos(q2)*(cos(q3)*(-(cos(q6)*sin(q5)*(KUKA_LBR_param_.dblLink7CogY*cos(q7) + KUKA_LBR_param_.dblLink7CogX*sin(q7))) + cos(q5)*(KUKA_LBR_param_.dblLink7CogX*cos(q7) - KUKA_LBR_param_.dblLink7CogY*sin(q7))) - sin(q3)*(sin(q4)*sin(q6)*(KUKA_LBR_param_.dblLink7CogY*cos(q7) + KUKA_LBR_param_.dblLink7CogX*sin(q7)) + cos(q4)*(cos(q5)*cos(q6)*(KUKA_LBR_param_.dblLink7CogY*cos(q7) + KUKA_LBR_param_.dblLink7CogX*sin(q7)) + sin(q5)*(KUKA_LBR_param_.dblLink7CogX*cos(q7) - KUKA_LBR_param_.dblLink7CogY*sin(q7))))))*(cos(q2)*(KUKA_LBR_param_.dblLink23Len + KUKA_LBR_param_.dblLink7CogY*cos(q7)*sin(q4)*sin(q5) + KUKA_LBR_param_.dblLink7CogX*sin(q4)*sin(q5)*sin(q7) + cos(q5)*sin(q4)*(-(KUKA_LBR_param_.dblLink7CogX*cos(q6)*cos(q7)) + KUKA_LBR_param_.dblLink7CogZ*sin(q6) + KUKA_LBR_param_.dblLink7CogY*cos(q6)*sin(q7)) + cos(q4)*(KUKA_LBR_param_.dblLink45Len + KUKA_LBR_param_.dblLink7CogZ*cos(q6) + KUKA_LBR_param_.dblLink7CogX*cos(q7)*sin(q6) - KUKA_LBR_param_.dblLink7CogY*sin(q6)*sin(q7))) + sin(q2)*(-(sin(q3)*(cos(q5)*(KUKA_LBR_param_.dblLink7CogY*cos(q7) + KUKA_LBR_param_.dblLink7CogX*sin(q7)) + sin(q5)*(KUKA_LBR_param_.dblLink7CogX*cos(q6)*cos(q7) - KUKA_LBR_param_.dblLink7CogZ*sin(q6) - KUKA_LBR_param_.dblLink7CogY*cos(q6)*sin(q7)))) + cos(q3)*(sin(q4)*(KUKA_LBR_param_.dblLink45Len + KUKA_LBR_param_.dblLink7CogZ*cos(q6) + KUKA_LBR_param_.dblLink7CogX*cos(q7)*sin(q6) - KUKA_LBR_param_.dblLink7CogY*sin(q6)*sin(q7)) - cos(q4)*(sin(q5)*(KUKA_LBR_param_.dblLink7CogY*cos(q7) + KUKA_LBR_param_.dblLink7CogX*sin(q7)) + cos(q5)*(-(KUKA_LBR_param_.dblLink7CogX*cos(q6)*cos(q7)) + KUKA_LBR_param_.dblLink7CogZ*sin(q6) + KUKA_LBR_param_.dblLink7CogY*cos(q6)*sin(q7)))))) + 2*KUKA_LBR_param_.dblLink7Mass*sin(q1)*(cos(q1)*(sin(q3)*(-(cos(q6)*sin(q5)*(KUKA_LBR_param_.dblLink7CogY*cos(q7) + KUKA_LBR_param_.dblLink7CogX*sin(q7))) + cos(q5)*(KUKA_LBR_param_.dblLink7CogX*cos(q7) - KUKA_LBR_param_.dblLink7CogY*sin(q7))) + cos(q3)*(sin(q4)*sin(q6)*(KUKA_LBR_param_.dblLink7CogY*cos(q7) + KUKA_LBR_param_.dblLink7CogX*sin(q7)) + cos(q4)*(cos(q5)*cos(q6)*(KUKA_LBR_param_.dblLink7CogY*cos(q7) + KUKA_LBR_param_.dblLink7CogX*sin(q7)) + sin(q5)*(KUKA_LBR_param_.dblLink7CogX*cos(q7) - KUKA_LBR_param_.dblLink7CogY*sin(q7))))) + cos(q2)*sin(q1)*(cos(q3)*(-(cos(q6)*sin(q5)*(KUKA_LBR_param_.dblLink7CogY*cos(q7) + KUKA_LBR_param_.dblLink7CogX*sin(q7))) + cos(q5)*(KUKA_LBR_param_.dblLink7CogX*cos(q7) - KUKA_LBR_param_.dblLink7CogY*sin(q7))) - sin(q3)*(sin(q4)*sin(q6)*(KUKA_LBR_param_.dblLink7CogY*cos(q7) + KUKA_LBR_param_.dblLink7CogX*sin(q7)) + cos(q4)*(cos(q5)*cos(q6)*(KUKA_LBR_param_.dblLink7CogY*cos(q7) + KUKA_LBR_param_.dblLink7CogX*sin(q7)) + sin(q5)*(KUKA_LBR_param_.dblLink7CogX*cos(q7) - KUKA_LBR_param_.dblLink7CogY*sin(q7))))))*(cos(q2)*(KUKA_LBR_param_.dblLink23Len + KUKA_LBR_param_.dblLink7CogY*cos(q7)*sin(q4)*sin(q5) + KUKA_LBR_param_.dblLink7CogX*sin(q4)*sin(q5)*sin(q7) + cos(q5)*sin(q4)*(-(KUKA_LBR_param_.dblLink7CogX*cos(q6)*cos(q7)) + KUKA_LBR_param_.dblLink7CogZ*sin(q6) + KUKA_LBR_param_.dblLink7CogY*cos(q6)*sin(q7)) + cos(q4)*(KUKA_LBR_param_.dblLink45Len + KUKA_LBR_param_.dblLink7CogZ*cos(q6) + KUKA_LBR_param_.dblLink7CogX*cos(q7)*sin(q6) - KUKA_LBR_param_.dblLink7CogY*sin(q6)*sin(q7))) + sin(q2)*(-(sin(q3)*(cos(q5)*(KUKA_LBR_param_.dblLink7CogY*cos(q7) + KUKA_LBR_param_.dblLink7CogX*sin(q7)) + sin(q5)*(KUKA_LBR_param_.dblLink7CogX*cos(q6)*cos(q7) - KUKA_LBR_param_.dblLink7CogZ*sin(q6) - KUKA_LBR_param_.dblLink7CogY*cos(q6)*sin(q7)))) + cos(q3)*(sin(q4)*(KUKA_LBR_param_.dblLink45Len + KUKA_LBR_param_.dblLink7CogZ*cos(q6) + KUKA_LBR_param_.dblLink7CogX*cos(q7)*sin(q6) - KUKA_LBR_param_.dblLink7CogY*sin(q6)*sin(q7)) - cos(q4)*(sin(q5)*(KUKA_LBR_param_.dblLink7CogY*cos(q7) + KUKA_LBR_param_.dblLink7CogX*sin(q7)) + cos(q5)*(-(KUKA_LBR_param_.dblLink7CogX*cos(q6)*cos(q7)) + KUKA_LBR_param_.dblLink7CogZ*sin(q6) + KUKA_LBR_param_.dblLink7CogY*cos(q6)*sin(q7)))))) + KUKA_LBR_param_.dblLink7Mass*cos(q1)*(cos(q2)*(KUKA_LBR_param_.dblLink7CogX*cos(q7)*sin(q4)*sin(q5) - KUKA_LBR_param_.dblLink7CogY*sin(q4)*sin(q5)*sin(q7) + cos(q5)*cos(q6)*sin(q4)*(KUKA_LBR_param_.dblLink7CogY*cos(q7) + KUKA_LBR_param_.dblLink7CogX*sin(q7)) - cos(q4)*sin(q6)*(KUKA_LBR_param_.dblLink7CogY*cos(q7) + KUKA_LBR_param_.dblLink7CogX*sin(q7))) + sin(q2)*(sin(q3)*(cos(q6)*sin(q5)*(KUKA_LBR_param_.dblLink7CogY*cos(q7) + KUKA_LBR_param_.dblLink7CogX*sin(q7)) + cos(q5)*(-(KUKA_LBR_param_.dblLink7CogX*cos(q7)) + KUKA_LBR_param_.dblLink7CogY*sin(q7))) - cos(q3)*(sin(q4)*sin(q6)*(KUKA_LBR_param_.dblLink7CogY*cos(q7) + KUKA_LBR_param_.dblLink7CogX*sin(q7)) + cos(q4)*(cos(q5)*cos(q6)*(KUKA_LBR_param_.dblLink7CogY*cos(q7) + KUKA_LBR_param_.dblLink7CogX*sin(q7)) + sin(q5)*(KUKA_LBR_param_.dblLink7CogX*cos(q7) - KUKA_LBR_param_.dblLink7CogY*sin(q7))))))*(sin(q1)*(-(sin(q3)*(cos(q5)*(KUKA_LBR_param_.dblLink7CogY*cos(q7) + KUKA_LBR_param_.dblLink7CogX*sin(q7)) + sin(q5)*(KUKA_LBR_param_.dblLink7CogX*cos(q6)*cos(q7) - KUKA_LBR_param_.dblLink7CogZ*sin(q6) - KUKA_LBR_param_.dblLink7CogY*cos(q6)*sin(q7)))) + cos(q3)*(sin(q4)*(KUKA_LBR_param_.dblLink45Len + KUKA_LBR_param_.dblLink7CogZ*cos(q6) + KUKA_LBR_param_.dblLink7CogX*cos(q7)*sin(q6) - KUKA_LBR_param_.dblLink7CogY*sin(q6)*sin(q7)) - cos(q4)*(sin(q5)*(KUKA_LBR_param_.dblLink7CogY*cos(q7) + KUKA_LBR_param_.dblLink7CogX*sin(q7)) + cos(q5)*(-(KUKA_LBR_param_.dblLink7CogX*cos(q6)*cos(q7)) + KUKA_LBR_param_.dblLink7CogZ*sin(q6) + KUKA_LBR_param_.dblLink7CogY*cos(q6)*sin(q7))))) + cos(q1)*cos(q2)*(cos(q3)*(cos(q5)*(KUKA_LBR_param_.dblLink7CogY*cos(q7) + KUKA_LBR_param_.dblLink7CogX*sin(q7)) + sin(q5)*(KUKA_LBR_param_.dblLink7CogX*cos(q6)*cos(q7) - KUKA_LBR_param_.dblLink7CogZ*sin(q6) - KUKA_LBR_param_.dblLink7CogY*cos(q6)*sin(q7))) + sin(q3)*(sin(q4)*(KUKA_LBR_param_.dblLink45Len + KUKA_LBR_param_.dblLink7CogZ*cos(q6) + KUKA_LBR_param_.dblLink7CogX*cos(q7)*sin(q6) - KUKA_LBR_param_.dblLink7CogY*sin(q6)*sin(q7)) - cos(q4)*(sin(q5)*(KUKA_LBR_param_.dblLink7CogY*cos(q7) + KUKA_LBR_param_.dblLink7CogX*sin(q7)) + cos(q5)*(-(KUKA_LBR_param_.dblLink7CogX*cos(q6)*cos(q7)) + KUKA_LBR_param_.dblLink7CogZ*sin(q6) + KUKA_LBR_param_.dblLink7CogY*cos(q6)*sin(q7)))))) - KUKA_LBR_param_.dblLink7Mass*cos(q1)*(cos(q2)*(cos(q7)*(KUKA_LBR_param_.dblLink7CogX*sin(q4)*sin(q5) - KUKA_LBR_param_.dblLink7CogY*cos(q4)*sin(q6)) - (KUKA_LBR_param_.dblLink7CogY*sin(q4)*sin(q5) + KUKA_LBR_param_.dblLink7CogX*cos(q4)*sin(q6))*sin(q7) + cos(q5)*cos(q6)*sin(q4)*(KUKA_LBR_param_.dblLink7CogY*cos(q7) + KUKA_LBR_param_.dblLink7CogX*sin(q7))) - sin(q2)*(sin(q3)*(-(cos(q6)*sin(q5)*(KUKA_LBR_param_.dblLink7CogY*cos(q7) + KUKA_LBR_param_.dblLink7CogX*sin(q7))) + cos(q5)*(KUKA_LBR_param_.dblLink7CogX*cos(q7) - KUKA_LBR_param_.dblLink7CogY*sin(q7))) + cos(q3)*(sin(q4)*sin(q6)*(KUKA_LBR_param_.dblLink7CogY*cos(q7) + KUKA_LBR_param_.dblLink7CogX*sin(q7)) + cos(q4)*(cos(q5)*cos(q6)*(KUKA_LBR_param_.dblLink7CogY*cos(q7) + KUKA_LBR_param_.dblLink7CogX*sin(q7)) + sin(q5)*(KUKA_LBR_param_.dblLink7CogX*cos(q7) - KUKA_LBR_param_.dblLink7CogY*sin(q7))))))*(sin(q1)*(-(sin(q3)*(cos(q5)*(KUKA_LBR_param_.dblLink7CogY*cos(q7) + KUKA_LBR_param_.dblLink7CogX*sin(q7)) + sin(q5)*(KUKA_LBR_param_.dblLink7CogX*cos(q6)*cos(q7) - KUKA_LBR_param_.dblLink7CogZ*sin(q6) - KUKA_LBR_param_.dblLink7CogY*cos(q6)*sin(q7)))) + cos(q3)*(sin(q4)*(KUKA_LBR_param_.dblLink45Len + KUKA_LBR_param_.dblLink7CogZ*cos(q6) + KUKA_LBR_param_.dblLink7CogX*cos(q7)*sin(q6) - KUKA_LBR_param_.dblLink7CogY*sin(q6)*sin(q7)) - cos(q4)*(sin(q5)*(KUKA_LBR_param_.dblLink7CogY*cos(q7) + KUKA_LBR_param_.dblLink7CogX*sin(q7)) + cos(q5)*(-(KUKA_LBR_param_.dblLink7CogX*cos(q6)*cos(q7)) + KUKA_LBR_param_.dblLink7CogZ*sin(q6) + KUKA_LBR_param_.dblLink7CogY*cos(q6)*sin(q7))))) + cos(q1)*cos(q2)*(cos(q3)*(cos(q5)*(KUKA_LBR_param_.dblLink7CogY*cos(q7) + KUKA_LBR_param_.dblLink7CogX*sin(q7)) + sin(q5)*(KUKA_LBR_param_.dblLink7CogX*cos(q6)*cos(q7) - KUKA_LBR_param_.dblLink7CogZ*sin(q6) - KUKA_LBR_param_.dblLink7CogY*cos(q6)*sin(q7))) + sin(q3)*(sin(q4)*(KUKA_LBR_param_.dblLink45Len + KUKA_LBR_param_.dblLink7CogZ*cos(q6) + KUKA_LBR_param_.dblLink7CogX*cos(q7)*sin(q6) - KUKA_LBR_param_.dblLink7CogY*sin(q6)*sin(q7)) - cos(q4)*(sin(q5)*(KUKA_LBR_param_.dblLink7CogY*cos(q7) + KUKA_LBR_param_.dblLink7CogX*sin(q7)) + cos(q5)*(-(KUKA_LBR_param_.dblLink7CogX*cos(q6)*cos(q7)) + KUKA_LBR_param_.dblLink7CogZ*sin(q6) + KUKA_LBR_param_.dblLink7CogY*cos(q6)*sin(q7)))))) + KUKA_LBR_param_.dblLink7Mass*sin(q1)*(cos(q2)*(KUKA_LBR_param_.dblLink7CogX*cos(q7)*sin(q4)*sin(q5) - KUKA_LBR_param_.dblLink7CogY*sin(q4)*sin(q5)*sin(q7) + cos(q5)*cos(q6)*sin(q4)*(KUKA_LBR_param_.dblLink7CogY*cos(q7) + KUKA_LBR_param_.dblLink7CogX*sin(q7)) - cos(q4)*sin(q6)*(KUKA_LBR_param_.dblLink7CogY*cos(q7) + KUKA_LBR_param_.dblLink7CogX*sin(q7))) + sin(q2)*(sin(q3)*(cos(q6)*sin(q5)*(KUKA_LBR_param_.dblLink7CogY*cos(q7) + KUKA_LBR_param_.dblLink7CogX*sin(q7)) + cos(q5)*(-(KUKA_LBR_param_.dblLink7CogX*cos(q7)) + KUKA_LBR_param_.dblLink7CogY*sin(q7))) - cos(q3)*(sin(q4)*sin(q6)*(KUKA_LBR_param_.dblLink7CogY*cos(q7) + KUKA_LBR_param_.dblLink7CogX*sin(q7)) + cos(q4)*(cos(q5)*cos(q6)*(KUKA_LBR_param_.dblLink7CogY*cos(q7) + KUKA_LBR_param_.dblLink7CogX*sin(q7)) + sin(q5)*(KUKA_LBR_param_.dblLink7CogX*cos(q7) - KUKA_LBR_param_.dblLink7CogY*sin(q7))))))*(cos(q2)*sin(q1)*(cos(q3)*(cos(q5)*(KUKA_LBR_param_.dblLink7CogY*cos(q7) + KUKA_LBR_param_.dblLink7CogX*sin(q7)) + sin(q5)*(KUKA_LBR_param_.dblLink7CogX*cos(q6)*cos(q7) - KUKA_LBR_param_.dblLink7CogZ*sin(q6) - KUKA_LBR_param_.dblLink7CogY*cos(q6)*sin(q7))) + sin(q3)*(sin(q4)*(KUKA_LBR_param_.dblLink45Len + KUKA_LBR_param_.dblLink7CogZ*cos(q6) + KUKA_LBR_param_.dblLink7CogX*cos(q7)*sin(q6) - KUKA_LBR_param_.dblLink7CogY*sin(q6)*sin(q7)) - cos(q4)*(sin(q5)*(KUKA_LBR_param_.dblLink7CogY*cos(q7) + KUKA_LBR_param_.dblLink7CogX*sin(q7)) + cos(q5)*(-(KUKA_LBR_param_.dblLink7CogX*cos(q6)*cos(q7)) + KUKA_LBR_param_.dblLink7CogZ*sin(q6) + KUKA_LBR_param_.dblLink7CogY*cos(q6)*sin(q7))))) + cos(q1)*(sin(q3)*(cos(q5)*(KUKA_LBR_param_.dblLink7CogY*cos(q7) + KUKA_LBR_param_.dblLink7CogX*sin(q7)) + sin(q5)*(KUKA_LBR_param_.dblLink7CogX*cos(q6)*cos(q7) - KUKA_LBR_param_.dblLink7CogZ*sin(q6) - KUKA_LBR_param_.dblLink7CogY*cos(q6)*sin(q7))) + cos(q3)*(-(sin(q4)*(KUKA_LBR_param_.dblLink45Len + KUKA_LBR_param_.dblLink7CogZ*cos(q6) + KUKA_LBR_param_.dblLink7CogX*cos(q7)*sin(q6) - KUKA_LBR_param_.dblLink7CogY*sin(q6)*sin(q7))) + cos(q4)*(sin(q5)*(KUKA_LBR_param_.dblLink7CogY*cos(q7) + KUKA_LBR_param_.dblLink7CogX*sin(q7)) + cos(q5)*(-(KUKA_LBR_param_.dblLink7CogX*cos(q6)*cos(q7)) + KUKA_LBR_param_.dblLink7CogZ*sin(q6) + KUKA_LBR_param_.dblLink7CogY*cos(q6)*sin(q7)))))) - KUKA_LBR_param_.dblLink7Mass*sin(q1)*(cos(q2)*(cos(q7)*(KUKA_LBR_param_.dblLink7CogX*sin(q4)*sin(q5) - KUKA_LBR_param_.dblLink7CogY*cos(q4)*sin(q6)) - (KUKA_LBR_param_.dblLink7CogY*sin(q4)*sin(q5) + KUKA_LBR_param_.dblLink7CogX*cos(q4)*sin(q6))*sin(q7) + cos(q5)*cos(q6)*sin(q4)*(KUKA_LBR_param_.dblLink7CogY*cos(q7) + KUKA_LBR_param_.dblLink7CogX*sin(q7))) - sin(q2)*(sin(q3)*(-(cos(q6)*sin(q5)*(KUKA_LBR_param_.dblLink7CogY*cos(q7) + KUKA_LBR_param_.dblLink7CogX*sin(q7))) + cos(q5)*(KUKA_LBR_param_.dblLink7CogX*cos(q7) - KUKA_LBR_param_.dblLink7CogY*sin(q7))) + cos(q3)*(sin(q4)*sin(q6)*(KUKA_LBR_param_.dblLink7CogY*cos(q7) + KUKA_LBR_param_.dblLink7CogX*sin(q7)) + cos(q4)*(cos(q5)*cos(q6)*(KUKA_LBR_param_.dblLink7CogY*cos(q7) + KUKA_LBR_param_.dblLink7CogX*sin(q7)) + sin(q5)*(KUKA_LBR_param_.dblLink7CogX*cos(q7) - KUKA_LBR_param_.dblLink7CogY*sin(q7))))))*(cos(q2)*sin(q1)*(cos(q3)*(cos(q5)*(KUKA_LBR_param_.dblLink7CogY*cos(q7) + KUKA_LBR_param_.dblLink7CogX*sin(q7)) + sin(q5)*(KUKA_LBR_param_.dblLink7CogX*cos(q6)*cos(q7) - KUKA_LBR_param_.dblLink7CogZ*sin(q6) - KUKA_LBR_param_.dblLink7CogY*cos(q6)*sin(q7))) + sin(q3)*(sin(q4)*(KUKA_LBR_param_.dblLink45Len + KUKA_LBR_param_.dblLink7CogZ*cos(q6) + KUKA_LBR_param_.dblLink7CogX*cos(q7)*sin(q6) - KUKA_LBR_param_.dblLink7CogY*sin(q6)*sin(q7)) - cos(q4)*(sin(q5)*(KUKA_LBR_param_.dblLink7CogY*cos(q7) + KUKA_LBR_param_.dblLink7CogX*sin(q7)) + cos(q5)*(-(KUKA_LBR_param_.dblLink7CogX*cos(q6)*cos(q7)) + KUKA_LBR_param_.dblLink7CogZ*sin(q6) + KUKA_LBR_param_.dblLink7CogY*cos(q6)*sin(q7))))) + cos(q1)*(sin(q3)*(cos(q5)*(KUKA_LBR_param_.dblLink7CogY*cos(q7) + KUKA_LBR_param_.dblLink7CogX*sin(q7)) + sin(q5)*(KUKA_LBR_param_.dblLink7CogX*cos(q6)*cos(q7) - KUKA_LBR_param_.dblLink7CogZ*sin(q6) - KUKA_LBR_param_.dblLink7CogY*cos(q6)*sin(q7))) + cos(q3)*(-(sin(q4)*(KUKA_LBR_param_.dblLink45Len + KUKA_LBR_param_.dblLink7CogZ*cos(q6) + KUKA_LBR_param_.dblLink7CogX*cos(q7)*sin(q6) - KUKA_LBR_param_.dblLink7CogY*sin(q6)*sin(q7))) + cos(q4)*(sin(q5)*(KUKA_LBR_param_.dblLink7CogY*cos(q7) + KUKA_LBR_param_.dblLink7CogX*sin(q7)) + cos(q5)*(-(KUKA_LBR_param_.dblLink7CogX*cos(q6)*cos(q7)) + KUKA_LBR_param_.dblLink7CogZ*sin(q6) + KUKA_LBR_param_.dblLink7CogY*cos(q6)*sin(q7)))))) + KUKA_LBR_param_.dblLink7Mass*cos(q1)*sin(q2)*(cos(q3)*(cos(q5)*(KUKA_LBR_param_.dblLink7CogY*cos(q7) + KUKA_LBR_param_.dblLink7CogX*sin(q7)) + sin(q5)*(KUKA_LBR_param_.dblLink7CogX*cos(q6)*cos(q7) - KUKA_LBR_param_.dblLink7CogZ*sin(q6) - KUKA_LBR_param_.dblLink7CogY*cos(q6)*sin(q7))) + sin(q3)*(sin(q4)*(KUKA_LBR_param_.dblLink45Len + KUKA_LBR_param_.dblLink7CogZ*cos(q6) + KUKA_LBR_param_.dblLink7CogX*cos(q7)*sin(q6) - KUKA_LBR_param_.dblLink7CogY*sin(q6)*sin(q7)) - cos(q4)*(sin(q5)*(KUKA_LBR_param_.dblLink7CogY*cos(q7) + KUKA_LBR_param_.dblLink7CogX*sin(q7)) + cos(q5)*(-(KUKA_LBR_param_.dblLink7CogX*cos(q6)*cos(q7)) + KUKA_LBR_param_.dblLink7CogZ*sin(q6) + KUKA_LBR_param_.dblLink7CogY*cos(q6)*sin(q7)))))*(sin(q1)*(cos(q3)*(-(cos(q6)*sin(q5)*(KUKA_LBR_param_.dblLink7CogY*cos(q7) + KUKA_LBR_param_.dblLink7CogX*sin(q7))) + cos(q5)*(KUKA_LBR_param_.dblLink7CogX*cos(q7) - KUKA_LBR_param_.dblLink7CogY*sin(q7))) - sin(q3)*(sin(q4)*sin(q6)*(KUKA_LBR_param_.dblLink7CogY*cos(q7) + KUKA_LBR_param_.dblLink7CogX*sin(q7)) + cos(q4)*(cos(q5)*cos(q6)*(KUKA_LBR_param_.dblLink7CogY*cos(q7) + KUKA_LBR_param_.dblLink7CogX*sin(q7)) + sin(q5)*(KUKA_LBR_param_.dblLink7CogX*cos(q7) - KUKA_LBR_param_.dblLink7CogY*sin(q7))))) + cos(q1)*(sin(q2)*(cos(q7)*(KUKA_LBR_param_.dblLink7CogX*sin(q4)*sin(q5) - KUKA_LBR_param_.dblLink7CogY*cos(q4)*sin(q6)) - (KUKA_LBR_param_.dblLink7CogY*sin(q4)*sin(q5) + KUKA_LBR_param_.dblLink7CogX*cos(q4)*sin(q6))*sin(q7) + cos(q5)*cos(q6)*sin(q4)*(KUKA_LBR_param_.dblLink7CogY*cos(q7) + KUKA_LBR_param_.dblLink7CogX*sin(q7))) + cos(q2)*(sin(q3)*(-(cos(q6)*sin(q5)*(KUKA_LBR_param_.dblLink7CogY*cos(q7) + KUKA_LBR_param_.dblLink7CogX*sin(q7))) + cos(q5)*(KUKA_LBR_param_.dblLink7CogX*cos(q7) - KUKA_LBR_param_.dblLink7CogY*sin(q7))) + cos(q3)*(sin(q4)*sin(q6)*(KUKA_LBR_param_.dblLink7CogY*cos(q7) + KUKA_LBR_param_.dblLink7CogX*sin(q7)) + cos(q4)*(cos(q5)*cos(q6)*(KUKA_LBR_param_.dblLink7CogY*cos(q7) + KUKA_LBR_param_.dblLink7CogX*sin(q7)) + sin(q5)*(KUKA_LBR_param_.dblLink7CogX*cos(q7) - KUKA_LBR_param_.dblLink7CogY*sin(q7))))))) + KUKA_LBR_param_.dblLink7Mass*cos(q1)*sin(q2)*(-(cos(q3)*(cos(q5)*(KUKA_LBR_param_.dblLink7CogY*cos(q7) + KUKA_LBR_param_.dblLink7CogX*sin(q7)) + sin(q5)*(KUKA_LBR_param_.dblLink7CogX*cos(q6)*cos(q7) - KUKA_LBR_param_.dblLink7CogZ*sin(q6) - KUKA_LBR_param_.dblLink7CogY*cos(q6)*sin(q7)))) + sin(q3)*(-(sin(q4)*(KUKA_LBR_param_.dblLink45Len + KUKA_LBR_param_.dblLink7CogZ*cos(q6) + KUKA_LBR_param_.dblLink7CogX*cos(q7)*sin(q6) - KUKA_LBR_param_.dblLink7CogY*sin(q6)*sin(q7))) + cos(q4)*(sin(q5)*(KUKA_LBR_param_.dblLink7CogY*cos(q7) + KUKA_LBR_param_.dblLink7CogX*sin(q7)) + cos(q5)*(-(KUKA_LBR_param_.dblLink7CogX*cos(q6)*cos(q7)) + KUKA_LBR_param_.dblLink7CogZ*sin(q6) + KUKA_LBR_param_.dblLink7CogY*cos(q6)*sin(q7)))))*(sin(q1)*(cos(q3)*(-(cos(q6)*sin(q5)*(KUKA_LBR_param_.dblLink7CogY*cos(q7) + KUKA_LBR_param_.dblLink7CogX*sin(q7))) + cos(q5)*(KUKA_LBR_param_.dblLink7CogX*cos(q7) - KUKA_LBR_param_.dblLink7CogY*sin(q7))) - sin(q3)*(sin(q4)*sin(q6)*(KUKA_LBR_param_.dblLink7CogY*cos(q7) + KUKA_LBR_param_.dblLink7CogX*sin(q7)) + cos(q4)*(cos(q5)*cos(q6)*(KUKA_LBR_param_.dblLink7CogY*cos(q7) + KUKA_LBR_param_.dblLink7CogX*sin(q7)) + sin(q5)*(KUKA_LBR_param_.dblLink7CogX*cos(q7) - KUKA_LBR_param_.dblLink7CogY*sin(q7))))) + cos(q1)*(sin(q2)*(cos(q7)*(KUKA_LBR_param_.dblLink7CogX*sin(q4)*sin(q5) - KUKA_LBR_param_.dblLink7CogY*cos(q4)*sin(q6)) - (KUKA_LBR_param_.dblLink7CogY*sin(q4)*sin(q5) + KUKA_LBR_param_.dblLink7CogX*cos(q4)*sin(q6))*sin(q7) + cos(q5)*cos(q6)*sin(q4)*(KUKA_LBR_param_.dblLink7CogY*cos(q7) + KUKA_LBR_param_.dblLink7CogX*sin(q7))) + cos(q2)*(sin(q3)*(-(cos(q6)*sin(q5)*(KUKA_LBR_param_.dblLink7CogY*cos(q7) + KUKA_LBR_param_.dblLink7CogX*sin(q7))) + cos(q5)*(KUKA_LBR_param_.dblLink7CogX*cos(q7) - KUKA_LBR_param_.dblLink7CogY*sin(q7))) + cos(q3)*(sin(q4)*sin(q6)*(KUKA_LBR_param_.dblLink7CogY*cos(q7) + KUKA_LBR_param_.dblLink7CogX*sin(q7)) + cos(q4)*(cos(q5)*cos(q6)*(KUKA_LBR_param_.dblLink7CogY*cos(q7) + KUKA_LBR_param_.dblLink7CogX*sin(q7)) + sin(q5)*(KUKA_LBR_param_.dblLink7CogX*cos(q7) - KUKA_LBR_param_.dblLink7CogY*sin(q7))))))) + KUKA_LBR_param_.dblLink7Mass*sin(q1)*sin(q2)*(cos(q3)*(cos(q5)*(KUKA_LBR_param_.dblLink7CogY*cos(q7) + KUKA_LBR_param_.dblLink7CogX*sin(q7)) + sin(q5)*(KUKA_LBR_param_.dblLink7CogX*cos(q6)*cos(q7) - KUKA_LBR_param_.dblLink7CogZ*sin(q6) - KUKA_LBR_param_.dblLink7CogY*cos(q6)*sin(q7))) + sin(q3)*(sin(q4)*(KUKA_LBR_param_.dblLink45Len + KUKA_LBR_param_.dblLink7CogZ*cos(q6) + KUKA_LBR_param_.dblLink7CogX*cos(q7)*sin(q6) - KUKA_LBR_param_.dblLink7CogY*sin(q6)*sin(q7)) - cos(q4)*(sin(q5)*(KUKA_LBR_param_.dblLink7CogY*cos(q7) + KUKA_LBR_param_.dblLink7CogX*sin(q7)) + cos(q5)*(-(KUKA_LBR_param_.dblLink7CogX*cos(q6)*cos(q7)) + KUKA_LBR_param_.dblLink7CogZ*sin(q6) + KUKA_LBR_param_.dblLink7CogY*cos(q6)*sin(q7)))))*(cos(q1)*(cos(q3)*(cos(q6)*sin(q5)*(KUKA_LBR_param_.dblLink7CogY*cos(q7) + KUKA_LBR_param_.dblLink7CogX*sin(q7)) + cos(q5)*(-(KUKA_LBR_param_.dblLink7CogX*cos(q7)) + KUKA_LBR_param_.dblLink7CogY*sin(q7))) + sin(q3)*(sin(q4)*sin(q6)*(KUKA_LBR_param_.dblLink7CogY*cos(q7) + KUKA_LBR_param_.dblLink7CogX*sin(q7)) + cos(q4)*(cos(q5)*cos(q6)*(KUKA_LBR_param_.dblLink7CogY*cos(q7) + KUKA_LBR_param_.dblLink7CogX*sin(q7)) + sin(q5)*(KUKA_LBR_param_.dblLink7CogX*cos(q7) - KUKA_LBR_param_.dblLink7CogY*sin(q7))))) + sin(q1)*(sin(q2)*(cos(q7)*(KUKA_LBR_param_.dblLink7CogX*sin(q4)*sin(q5) - KUKA_LBR_param_.dblLink7CogY*cos(q4)*sin(q6)) - (KUKA_LBR_param_.dblLink7CogY*sin(q4)*sin(q5) + KUKA_LBR_param_.dblLink7CogX*cos(q4)*sin(q6))*sin(q7) + cos(q5)*cos(q6)*sin(q4)*(KUKA_LBR_param_.dblLink7CogY*cos(q7) + KUKA_LBR_param_.dblLink7CogX*sin(q7))) + cos(q2)*(sin(q3)*(-(cos(q6)*sin(q5)*(KUKA_LBR_param_.dblLink7CogY*cos(q7) + KUKA_LBR_param_.dblLink7CogX*sin(q7))) + cos(q5)*(KUKA_LBR_param_.dblLink7CogX*cos(q7) - KUKA_LBR_param_.dblLink7CogY*sin(q7))) + cos(q3)*(sin(q4)*sin(q6)*(KUKA_LBR_param_.dblLink7CogY*cos(q7) + KUKA_LBR_param_.dblLink7CogX*sin(q7)) + cos(q4)*(cos(q5)*cos(q6)*(KUKA_LBR_param_.dblLink7CogY*cos(q7) + KUKA_LBR_param_.dblLink7CogX*sin(q7)) + sin(q5)*(KUKA_LBR_param_.dblLink7CogX*cos(q7) - KUKA_LBR_param_.dblLink7CogY*sin(q7))))))) + KUKA_LBR_param_.dblLink7Mass*sin(q1)*sin(q2)*(-(cos(q3)*(cos(q5)*(KUKA_LBR_param_.dblLink7CogY*cos(q7) + KUKA_LBR_param_.dblLink7CogX*sin(q7)) + sin(q5)*(KUKA_LBR_param_.dblLink7CogX*cos(q6)*cos(q7) - KUKA_LBR_param_.dblLink7CogZ*sin(q6) - KUKA_LBR_param_.dblLink7CogY*cos(q6)*sin(q7)))) + sin(q3)*(-(sin(q4)*(KUKA_LBR_param_.dblLink45Len + KUKA_LBR_param_.dblLink7CogZ*cos(q6) + KUKA_LBR_param_.dblLink7CogX*cos(q7)*sin(q6) - KUKA_LBR_param_.dblLink7CogY*sin(q6)*sin(q7))) + cos(q4)*(sin(q5)*(KUKA_LBR_param_.dblLink7CogY*cos(q7) + KUKA_LBR_param_.dblLink7CogX*sin(q7)) + cos(q5)*(-(KUKA_LBR_param_.dblLink7CogX*cos(q6)*cos(q7)) + KUKA_LBR_param_.dblLink7CogZ*sin(q6) + KUKA_LBR_param_.dblLink7CogY*cos(q6)*sin(q7)))))*(cos(q1)*(cos(q3)*(cos(q6)*sin(q5)*(KUKA_LBR_param_.dblLink7CogY*cos(q7) + KUKA_LBR_param_.dblLink7CogX*sin(q7)) + cos(q5)*(-(KUKA_LBR_param_.dblLink7CogX*cos(q7)) + KUKA_LBR_param_.dblLink7CogY*sin(q7))) + sin(q3)*(sin(q4)*sin(q6)*(KUKA_LBR_param_.dblLink7CogY*cos(q7) + KUKA_LBR_param_.dblLink7CogX*sin(q7)) + cos(q4)*(cos(q5)*cos(q6)*(KUKA_LBR_param_.dblLink7CogY*cos(q7) + KUKA_LBR_param_.dblLink7CogX*sin(q7)) + sin(q5)*(KUKA_LBR_param_.dblLink7CogX*cos(q7) - KUKA_LBR_param_.dblLink7CogY*sin(q7))))) + sin(q1)*(sin(q2)*(cos(q7)*(KUKA_LBR_param_.dblLink7CogX*sin(q4)*sin(q5) - KUKA_LBR_param_.dblLink7CogY*cos(q4)*sin(q6)) - (KUKA_LBR_param_.dblLink7CogY*sin(q4)*sin(q5) + KUKA_LBR_param_.dblLink7CogX*cos(q4)*sin(q6))*sin(q7) + cos(q5)*cos(q6)*sin(q4)*(KUKA_LBR_param_.dblLink7CogY*cos(q7) + KUKA_LBR_param_.dblLink7CogX*sin(q7))) + cos(q2)*(sin(q3)*(-(cos(q6)*sin(q5)*(KUKA_LBR_param_.dblLink7CogY*cos(q7) + KUKA_LBR_param_.dblLink7CogX*sin(q7))) + cos(q5)*(KUKA_LBR_param_.dblLink7CogX*cos(q7) - KUKA_LBR_param_.dblLink7CogY*sin(q7))) + cos(q3)*(sin(q4)*sin(q6)*(KUKA_LBR_param_.dblLink7CogY*cos(q7) + KUKA_LBR_param_.dblLink7CogX*sin(q7)) + cos(q4)*(cos(q5)*cos(q6)*(KUKA_LBR_param_.dblLink7CogY*cos(q7) + KUKA_LBR_param_.dblLink7CogX*sin(q7)) + sin(q5)*(KUKA_LBR_param_.dblLink7CogX*cos(q7) - KUKA_LBR_param_.dblLink7CogY*sin(q7)))))))))/2.0;
